simulink model "FeedBack_Linearization"  (R2021b)
(part 5 of 9)

t1997 = t961.*1.9738e-1;
t2000 = t869+t1374;
t2035 = t863+t1515;
t2039 = t1011.*1.9738e-1;
t2045 = t1013.*1.9738e-1;
t2053 = t919+t1532;
t2058 = (t1386+t7.*(t88-t617)).^2;
t2071 = t1060.*3.466000000000001e-2;
t2073 = t1064.*3.466000000000001e-2;
t2085 = t1061.*2.324e-2;
t2089 = t1063.*2.324e-2;
t2102 = t920+t1601;
t2116 = -dq7.*t8.*(t1386+t7.*(t88-t617));
t2119 = -dq7.*t15.*(t1386+t7.*(t88-t617));
t2140 = dq7.*t8.*(t1386+t7.*(t88-t617));
t2206 = t14.*t2179;
t2207 = t8.*t2182;
t2208 = t15.*t2182;
t2210 = -t2184;
t2213 = -t2186;
t2215 = -t2187;
t2216 = t6.*t2164;
t2218 = t7.*t2164;
t2220 = t7.*t2165;
t2221 = t8.*t2165;
t2222 = t13.*t2164;
t2223 = t14.*t2164;
t2224 = t14.*t2165;
t2225 = t15.*t2165;
t2229 = dq6.*t2180.*2.0;
t2231 = -t2202;
t2232 = dq5.*t2181.*2.0;
t2233 = dq6.*t2184.*2.0;
t2236 = dq5.*t2186.*2.0;
t2240 = t7.*t2179;
t2256 = t7.*t2212;
t2258 = t14.*t2212;
t2259 = t8.*t2217;
t2260 = -t2211;
t2261 = t15.*t2217;
t2265 = -t2219;
t2270 = dq7.*t1601.*(-2.324e-2);
t2273 = t1626.*(-2.324e-2);
t2278 = dq6.*t2214.*2.0;
t2280 = dq6.*t2219.*2.0;
t2288 = t1647.*(-3.466000000000001e-2);
t2289 = t916+t1792;
t2290 = t1626.*2.324e-2;
t2299 = t22.*t1601.*(-3.466000000000001e-2);
t2300 = t8.*t2262;
t2301 = t15.*t2262;
t2307 = dq7.*t2263.*2.0;
t2308 = dq7.*t2267.*2.0;
t2311 = t22.*t1601.*3.466000000000001e-2;
t2315 = t969+t1795;
t2352 = t1387+t1594;
t2357 = -t2351;
t2359 = t573.*t2165;
t2363 = t1375+t1633;
t2372 = t604.*t2164;
t2374 = t1528+t1631;
t2377 = -t2369;
t2378 = -t2370;
t2380 = t1516+t1668;
t2430 = -t2164.*(t88-t617);
C = ft_5({dq1,dq2,dq3,dq4,dq5,dq6,dq7,t10,t1000,t1001,t1003,t1004,t1007,t1008,t1010,t1012,t1013,t1014,t1015,t1016,t1017,t1018,t1019,t1020,t1021,t1022,t1023,t1024,t1025,t1026,t1029,t1031,t1032,t1033,t1034,t1035,t1036,t1038,t1039,t1040,t1041,t1044,t1045,t1046,t105,t1050,t1051,t1052,t1053,t1054,t1055,t1056,t1058,t1059,t1060,t1062,t1063,t1064,t1066,t1067,t1069,t107,t1070,t1072,t1074,t1075,t1076,t1077,t1079,t1081,t1089,t1091,t1092,t1094,t1096,t1097,t11,t1101,t1102,t1103,t1104,t1105,t1106,t1109,t1110,t1113,t1114,t1115,t1117,t1118,t1119,t112,t1123,t1125,t1126,t1128,t1130,t1132,t1135,t1136,t1137,t1138,t1139,t114,t1140,t1141,t1142,t1143,t1144,t1145,t1146,t1147,t1159,t1161,t1164,t1165,t1166,t1167,t1168,t1169,t1172,t1173,t1174,t1175,t1176,t1177,t1178,t1179,t1180,t1181,t1182,t1183,t1184,t1187,t1188,t1189,t119,t1190,t1193,t1194,t1195,t1197,t1198,t1199,t12,t1200,t1201,t1202,t1203,t1204,t1205,t1206,t1207,t1208,t1209,t1211,t1212,t1213,t1214,t1215,t1216,t1217,t1218,t1219,t122,t1220,t1224,t1225,t1226,t1228,t1229,t1231,t1232,t1238,t1242,t1243,t1244,t1246,t1249,t1250,t1253,t1256,t1257,t1263,t1264,t1265,t1267,t1268,t1269,t1270,t1273,t1274,t1275,t1286,t1287,t1288,t1289,t1290,t1291,t1292,t1293,t1295,t1296,t1299,t13,t130,t1300,t1304,t1305,t1306,t1309,t1312,t1313,t1315,t1318,t1325,t1327,t1328,t1329,t1330,t1339,t1341,t1342,t1346,t1347,t1348,t1349,t1350,t1351,t1352,t1356,t1357,t1360,t1361,t1362,t1363,t1364,t1365,t1368,t1369,t137,t1374,t1375,t1376,t1377,t1380,t1381,t1382,t1384,t1385,t1386,t1387,t1388,t1389,t139,t1390,t1391,t14,t1409,t1410,t1412,t1416,t1417,t1418,t1423,t1424,t1425,t1428,t1429,t1430,t1431,t1432,t1435,t1436,t144,t1441,t1449,t1450,t1451,t1453,t1455,t1456,t1462,t1467,t1471,t1472,t1473,t1474,t1475,t1480,t1487,t1488,t1489,t149,t1490,t1491,t1492,t1495,t1496,t1497,t1498,t15,t1506,t1508,t1509,t151,t1510,t1511,t1512,t1513,t1515,t1516,t1517,t1518,t1519,t152,t1526,t1527,t1528,t1529,t1530,t1537,t1538,t1539,t1540,t1541,t1542,t1543,t1544,t1545,t1546,t1547,t1548,t1549,t1550,t1551,t1552,t1553,t1554,t1556,t1557,t1561,t1562,t1563,t1564,t1565,t1566,t1567,t1568,t1569,t1570,t1571,t1572,t1574,t1577,t1578,t1579,t1581,t1582,t1583,t1584,t1585,t1589,t1591,t1596,t1598,t16,t160,t1601,t1603,t1604,t1605,t1606,t1607,t1608,t1609,t1611,t1612,t1613,t1616,t1618,t1622,t1624,t1625,t1626,t1627,t1629,t1630,t1633,t1634,t1635,t1636,t1637,t1638,t1642,t1643,t1644,t1647,t1648,t1649,t165,t1650,t1651,t1652,t1653,t1654,t1655,t1657,t1658,t1659,t1660,t1661,t1662,t1663,t1664,t1666,t1667,t1668,t1670,t1671,t1672,t1673,t1674,t1675,t1678,t1679,t1680,t1681,t1682,t1683,t1685,t1686,t1687,t1688,t1690,t1691,t1692,t1693,t1694,t1696,t1697,t1699,t17,t1700,t1701,t1702,t1704,t1705,t1706,t1707,t171,t1710,t1711,t1715,t1716,t1717,t1718,t1719,t1720,t1721,t1722,t1723,t1725,t1726,t1727,t1729,t1731,t1734,t1735,t1736,t1738,t1740,t1742,t1744,t1746,t1748,t1749,t175,t1751,t1752,t1757,t1759,t1760,t1761,t1762,t1763,t1765,t1766,t1769,t1770,t1772,t1773,t1774,t1775,t1776,t1779,t1780,t1782,t1786,t1790,t1791,t1792,t1793,t1795,t1798,t1799,t180,t1800,t1801,t1802,t1803,t1804,t1805,t1806,t1807,t1811,t1812,t1813,t1814,t1815,t1816,t1817,t1819,t182,t1822,t1823,t1824,t1825,t1826,t1827,t1828,t1829,t1830,t1831,t1834,t1835,t1836,t1837,t1839,t1840,t1841,t1842,t1843,t1844,t1846,t1847,t1849,t185,t1850,t1851,t1852,t1855,t1856,t1859,t186,t1860,t1861,t1863,t1864,t1865,t1866,t1867,t187,t1871,t1872,t1873,t1874,t1875,t1876,t1877,t1878,t1880,t1881,t1882,t1884,t1885,t1886,t1887,t1888,t189,t1890,t1891,t1892,t1893,t1896,t1897,t1898,t1900,t1901,t1902,t1903,t1905,t1907,t1908,t1909,t1911,t1912,t1913,t1914,t1915,t1917,t1918,t1919,t1921,t1922,t1924,t1927,t1928,t1932,t1933,t1934,t1935,t1936,t1937,t1941,t1942,t1944,t1945,t1946,t1949,t1950,t1951,t1952,t1953,t1955,t1957,t1959,t1960,t1962,t1963,t1967,t1968,t1969,t1970,t1971,t1974,t1975,t1976,t1977,t1978,t1980,t1982,t1983,t1984,t1985,t1986,t1988,t1990,t1992,t1997,t1998,t2,t2000,t2001,t2002,t2003,t2006,t2008,t2009,t2010,t2011,t2013,t2014,t2015,t2016,t2018,t2020,t2022,t2023,t2026,t2028,t2029,t2030,t2032,t2033,t2034,t2035,t2036,t2038,t2039,t2041,t2042,t2043,t2045,t2047,t2049,t2056,t2057,t2058,t2059,t2060,t2065,t2066,t2071,t2072,t2073,t2075,t2077,t2078,t208,t2082,t2083,t2085,t2086,t2089,t2093,t2094,t2098,t2099,t21,t2101,t2104,t2105,t2109,t2111,t2113,t2114,t2117,t2119,t2120,t2121,t2123,t2125,t2126,t2129,t2130,t2133,t2134,t2140,t2141,t2146,t2147,t2148,t2149,t2150,t2152,t2155,t2156,t2157,t2158,t2160,t2162,t2163,t2164,t2165,t2166,t2167,t2170,t2171,t2172,t2173,t2174,t2175,t2177,t2179,t2180,t2181,t2182,t2183,t2184,t2186,t2187,t2192,t2193,t2196,t2197,t22,t2201,t2204,t2206,t2207,t2208,t2209,t221,t2210,t2212,t2213,t2214,t2215,t2216,t2217,t2218,t2219,t2220,t2221,t2222,t2223,t2224,t2225,t2226,t2229,t223,t2230,t2231,t2232,t2233,t2236,t2240,t2249,t2251,t2256,t2258,t2259,t2260,t2261,t2262,t2263,t2265,t2266,t2267,t2270,t2272,t2277,t2278,t2280,t2284,t2285,t2288,t2289,t2290,t2292,t2293,t2296,t2298,t23,t230,t2300,t2301,t2306,t2307,t2308,t2309,t231,t2310,t2311,t2313,t2315,t2316,t2317,t2318,t232,t2327,t2331,t2333,t2336,t2337,t234,t2341,t2342,t2344,t2348,t235,t2350,t2351,t2352,t2353,t2356,t2357,t2359,t236,t2360,t2361,t2363,t2365,t2368,t2369,t237,t2370,t2372,t2374,t2376,t2377,t2378,t238,t2380,t2381,t2382,t2384,t2385,t2387,t2388,t239,t2390,t2391,t2393,t2396,t2397,t24,t240,t2400,t2402,t2403,t2404,t2405,t2406,t2407,t2408,t2409,t241,t2411,t2412,t2414,t2416,t2418,t242,t2422,t2423,t2424,t2425,t2426,t2427,t2428,t2429,t243,t2431,t2432,t2433,t2435,t2436,t2439,t244,t2440,t2441,t2442,t2443,t2444,t2447,t2449,t2451,t2453,t2455,t2456,t2458,t2459,t2462,t2463,t2464,t2466,t2467,t2468,t2469,t2470,t2471,t2472,t2473,t2474,t2475,t2479,t2480,t2481,t2484,t2490,t2492,t2493,t2494,t2496,t25,t250,t2502,t2506,t2508,t2509,t251,t2512,t2518,t252,t2525,t2526,t2527,t2528,t2529,t253,t2532,t2533,t2534,t2536,t2538,t2539,t254,t2547,t2548,t2549,t2550,t2551,t2558,t2572,t258,t2582,t2586,t259,t2594,t26,t2606,t2607,t2612,t2618,t2619,t2620,t2622,t2623,t2624,t2634,t2635,t2636,t2638,t2639,t2652,t2653,t2659,t2668,t267,t2671,t2672,t2673,t2674,t2675,t2677,t2678,t2679,t268,t2684,t2687,t269,t2690,t2691,t2693,t2696,t27,t270,t2701,t2703,t2706,t2707,t2708,t2709,t271,t2710,t2711,t2712,t2713,t2718,t272,t2720,t2722,t2725,t273,t2730,t2731,t2734,t2735,t274,t2745,t2748,t275,t2755,t2756,t2757,t2758,t276,t2760,t2761,t2762,t2765,t2766,t2768,t277,t2770,t2771,t2774,t2775,t2776,t2778,t2779,t2784,t2785,t2786,t2787,t2788,t279,t28,t280,t2802,t2805,t281,t282,t2822,t2827,t283,t2830,t2833,t2834,t284,t2844,t285,t2854,t286,t2869,t287,t2870,t288,t289,t2891,t2897,t2898,t2899,t29,t290,t2924,t2929,t293,t294,t2943,t2944,t2946,t295,t2952,t296,t2963,t297,t2971,t2972,t298,t3,t30,t301,t307,t308,t309,t31,t310,t311,t312,t313,t315,t316,t317,t318,t319,t32,t320,t322,t3248,t3249,t3252,t327,t328,t329,t33,t330,t331,t3372,t338,t34,t342,t3440,t3443,t346,t347,t3476,t348,t349,t35,t358,t36,t3669,t3672,t3673,t3679,t37,t387,t39,t390,t394,t4,t40,t406,t408,t415,t416,t417,t418,t419,t420,t427,t428,t429,t43,t431,t432,t433,t434,t435,t436,t438,t439,t441,t442,t443,t444,t446,t448,t45,t450,t451,t452,t453,t455,t456,t457,t458,t459,t46,t460,t461,t463,t464,t465,t466,t467,t468,t469,t470,t476,t477,t478,t479,t480,t481,t483,t484,t49,t494,t495,t496,t5,t50,t51,t510,t511,t512,t515,t516,t517,t518,t522,t523,t524,t525,t526,t527,t528,t529,t530,t531,t533,t534,t535,t536,t537,t538,t542,t543,t545,t546,t547,t548,t549,t55,t550,t551,t552,t553,t554,t556,t557,t558,t561,t562,t563,t564,t565,t566,t567,t568,t569,t57,t570,t571,t572,t573,t574,t575,t576,t577,t578,t579,t58,t580,t581,t582,t583,t584,t585,t586,t587,t588,t589,t590,t591,t592,t593,t594,t595,t596,t597,t598,t599,t6,t600,t601,t602,t603,t604,t605,t606,t607,t608,t609,t61,t612,t613,t614,t615,t616,t617,t618,t619,t620,t621,t622,t623,t624,t626,t627,t628,t629,t63,t631,t632,t633,t634,t635,t637,t639,t64,t640,t642,t643,t644,t646,t647,t648,t649,t650,t651,t652,t653,t654,t656,t657,t658,t660,t661,t662,t663,t664,t665,t667,t67,t670,t671,t673,t675,t676,t677,t678,t679,t680,t681,t683,t684,t685,t686,t687,t688,t689,t69,t691,t692,t693,t694,t695,t696,t697,t698,t699,t7,t70,t700,t701,t702,t703,t704,t705,t706,t707,t708,t71,t712,t713,t714,t72,t720,t721,t722,t723,t724,t725,t726,t728,t729,t73,t730,t731,t735,t74,t740,t743,t745,t748,t75,t750,t751,t753,t754,t755,t756,t757,t758,t759,t76,t760,t762,t764,t765,t766,t769,t77,t770,t773,t774,t776,t777,t778,t779,t78,t780,t782,t783,t785,t786,t787,t788,t79,t791,t792,t794,t795,t796,t797,t799,t8,t80,t800,t802,t803,t805,t806,t807,t809,t81,t810,t811,t812,t813,t814,t815,t816,t817,t818,t819,t82,t820,t821,t822,t827,t83,t831,t834,t835,t836,t837,t838,t839,t84,t840,t841,t842,t843,t845,t846,t847,t848,t849,t85,t850,t851,t853,t854,t855,t856,t857,t859,t86,t860,t862,t863,t864,t866,t867,t868,t87,t870,t871,t872,t873,t876,t877,t878,t88,t880,t881,t882,t883,t884,t885,t887,t888,t889,t89,t890,t891,t892,t893,t894,t895,t896,t897,t898,t899,t9,t90,t900,t901,t902,t903,t904,t905,t907,t908,t91,t911,t918,t92,t921,t922,t923,t926,t927,t928,t930,t931,t932,t933,t934,t935,t936,t937,t938,t939,t94,t940,t941,t942,t943,t945,t946,t947,t948,t949,t950,t951,t952,t953,t955,t957,t958,t959,t961,t963,t964,t966,t967,t969,t97,t972,t973,t974,t975,t976,t977,t978,t979,t980,t982,t983,t985,t986,t987,t988,t992,t994,t995,t997,t999});
end
function C = ft_5(ct)
dq1 = ct{1};
dq2 = ct{2};
dq3 = ct{3};
dq4 = ct{4};
dq5 = ct{5};
dq6 = ct{6};
dq7 = ct{7};
t10 = ct{8};
t1000 = ct{9};
t1001 = ct{10};
t1003 = ct{11};
t1004 = ct{12};
t1007 = ct{13};
t1008 = ct{14};
t1010 = ct{15};
t1012 = ct{16};
t1013 = ct{17};
t1014 = ct{18};
t1015 = ct{19};
t1016 = ct{20};
t1017 = ct{21};
t1018 = ct{22};
t1019 = ct{23};
t1020 = ct{24};
t1021 = ct{25};
t1022 = ct{26};
t1023 = ct{27};
t1024 = ct{28};
t1025 = ct{29};
t1026 = ct{30};
t1029 = ct{31};
t1031 = ct{32};
t1032 = ct{33};
t1033 = ct{34};
t1034 = ct{35};
t1035 = ct{36};
t1036 = ct{37};
t1038 = ct{38};
t1039 = ct{39};
t1040 = ct{40};
t1041 = ct{41};
t1044 = ct{42};
t1045 = ct{43};
t1046 = ct{44};
t105 = ct{45};
t1050 = ct{46};
t1051 = ct{47};
t1052 = ct{48};
t1053 = ct{49};
t1054 = ct{50};
t1055 = ct{51};
t1056 = ct{52};
t1058 = ct{53};
t1059 = ct{54};
t1060 = ct{55};
t1062 = ct{56};
t1063 = ct{57};
t1064 = ct{58};
t1066 = ct{59};
t1067 = ct{60};
t1069 = ct{61};
t107 = ct{62};
t1070 = ct{63};
t1072 = ct{64};
t1074 = ct{65};
t1075 = ct{66};
t1076 = ct{67};
t1077 = ct{68};
t1079 = ct{69};
t1081 = ct{70};
t1089 = ct{71};
t1091 = ct{72};
t1092 = ct{73};
t1094 = ct{74};
t1096 = ct{75};
t1097 = ct{76};
t11 = ct{77};
t1101 = ct{78};
t1102 = ct{79};
t1103 = ct{80};
t1104 = ct{81};
t1105 = ct{82};
t1106 = ct{83};
t1109 = ct{84};
t1110 = ct{85};
t1113 = ct{86};
t1114 = ct{87};
t1115 = ct{88};
t1117 = ct{89};
t1118 = ct{90};
t1119 = ct{91};
t112 = ct{92};
t1123 = ct{93};
t1125 = ct{94};
t1126 = ct{95};
t1128 = ct{96};
t1130 = ct{97};
t1132 = ct{98};
t1135 = ct{99};
t1136 = ct{100};
t1137 = ct{101};
t1138 = ct{102};
t1139 = ct{103};
t114 = ct{104};
t1140 = ct{105};
t1141 = ct{106};
t1142 = ct{107};
t1143 = ct{108};
t1144 = ct{109};
t1145 = ct{110};
t1146 = ct{111};
t1147 = ct{112};
t1159 = ct{113};
t1161 = ct{114};
t1164 = ct{115};
t1165 = ct{116};
t1166 = ct{117};
t1167 = ct{118};
t1168 = ct{119};
t1169 = ct{120};
t1172 = ct{121};
t1173 = ct{122};
t1174 = ct{123};
t1175 = ct{124};
t1176 = ct{125};
t1177 = ct{126};
t1178 = ct{127};
t1179 = ct{128};
t1180 = ct{129};
t1181 = ct{130};
t1182 = ct{131};
t1183 = ct{132};
t1184 = ct{133};
t1187 = ct{134};
t1188 = ct{135};
t1189 = ct{136};
t119 = ct{137};
t1190 = ct{138};
t1193 = ct{139};
t1194 = ct{140};
t1195 = ct{141};
t1197 = ct{142};
t1198 = ct{143};
t1199 = ct{144};
t12 = ct{145};
t1200 = ct{146};
t1201 = ct{147};
t1202 = ct{148};
t1203 = ct{149};
t1204 = ct{150};
t1205 = ct{151};
t1206 = ct{152};
t1207 = ct{153};
t1208 = ct{154};
t1209 = ct{155};
t1211 = ct{156};
t1212 = ct{157};
t1213 = ct{158};
t1214 = ct{159};
t1215 = ct{160};
t1216 = ct{161};
t1217 = ct{162};
t1218 = ct{163};
t1219 = ct{164};
t122 = ct{165};
t1220 = ct{166};
t1224 = ct{167};
t1225 = ct{168};
t1226 = ct{169};
t1228 = ct{170};
t1229 = ct{171};
t1231 = ct{172};
t1232 = ct{173};
t1238 = ct{174};
t1242 = ct{175};
t1243 = ct{176};
t1244 = ct{177};
t1246 = ct{178};
t1249 = ct{179};
t1250 = ct{180};
t1253 = ct{181};
t1256 = ct{182};
t1257 = ct{183};
t1263 = ct{184};
t1264 = ct{185};
t1265 = ct{186};
t1267 = ct{187};
t1268 = ct{188};
t1269 = ct{189};
t1270 = ct{190};
t1273 = ct{191};
t1274 = ct{192};
t1275 = ct{193};
t1286 = ct{194};
t1287 = ct{195};
t1288 = ct{196};
t1289 = ct{197};
t1290 = ct{198};
t1291 = ct{199};
t1292 = ct{200};
t1293 = ct{201};
t1295 = ct{202};
t1296 = ct{203};
t1299 = ct{204};
t13 = ct{205};
t130 = ct{206};
t1300 = ct{207};
t1304 = ct{208};
t1305 = ct{209};
t1306 = ct{210};
t1309 = ct{211};
t1312 = ct{212};
t1313 = ct{213};
t1315 = ct{214};
t1318 = ct{215};
t1325 = ct{216};
t1327 = ct{217};
t1328 = ct{218};
t1329 = ct{219};
t1330 = ct{220};
t1339 = ct{221};
t1341 = ct{222};
t1342 = ct{223};
t1346 = ct{224};
t1347 = ct{225};
t1348 = ct{226};
t1349 = ct{227};
t1350 = ct{228};
t1351 = ct{229};
t1352 = ct{230};
t1356 = ct{231};
t1357 = ct{232};
t1360 = ct{233};
t1361 = ct{234};
t1362 = ct{235};
t1363 = ct{236};
t1364 = ct{237};
t1365 = ct{238};
t1368 = ct{239};
t1369 = ct{240};
t137 = ct{241};
t1374 = ct{242};
t1375 = ct{243};
t1376 = ct{244};
t1377 = ct{245};
t1380 = ct{246};
t1381 = ct{247};
t1382 = ct{248};
t1384 = ct{249};
t1385 = ct{250};
t1386 = ct{251};
t1387 = ct{252};
t1388 = ct{253};
t1389 = ct{254};
t139 = ct{255};
t1390 = ct{256};
t1391 = ct{257};
t14 = ct{258};
t1409 = ct{259};
t1410 = ct{260};
t1412 = ct{261};
t1416 = ct{262};
t1417 = ct{263};
t1418 = ct{264};
t1423 = ct{265};
t1424 = ct{266};
t1425 = ct{267};
t1428 = ct{268};
t1429 = ct{269};
t1430 = ct{270};
t1431 = ct{271};
t1432 = ct{272};
t1435 = ct{273};
t1436 = ct{274};
t144 = ct{275};
t1441 = ct{276};
t1449 = ct{277};
t1450 = ct{278};
t1451 = ct{279};
t1453 = ct{280};
t1455 = ct{281};
t1456 = ct{282};
t1462 = ct{283};
t1467 = ct{284};
t1471 = ct{285};
t1472 = ct{286};
t1473 = ct{287};
t1474 = ct{288};
t1475 = ct{289};
t1480 = ct{290};
t1487 = ct{291};
t1488 = ct{292};
t1489 = ct{293};
t149 = ct{294};
t1490 = ct{295};
t1491 = ct{296};
t1492 = ct{297};
t1495 = ct{298};
t1496 = ct{299};
t1497 = ct{300};
t1498 = ct{301};
t15 = ct{302};
t1506 = ct{303};
t1508 = ct{304};
t1509 = ct{305};
t151 = ct{306};
t1510 = ct{307};
t1511 = ct{308};
t1512 = ct{309};
t1513 = ct{310};
t1515 = ct{311};
t1516 = ct{312};
t1517 = ct{313};
t1518 = ct{314};
t1519 = ct{315};
t152 = ct{316};
t1526 = ct{317};
t1527 = ct{318};
t1528 = ct{319};
t1529 = ct{320};
t1530 = ct{321};
t1537 = ct{322};
t1538 = ct{323};
t1539 = ct{324};
t1540 = ct{325};
t1541 = ct{326};
t1542 = ct{327};
t1543 = ct{328};
t1544 = ct{329};
t1545 = ct{330};
t1546 = ct{331};
t1547 = ct{332};
t1548 = ct{333};
t1549 = ct{334};
t1550 = ct{335};
t1551 = ct{336};
t1552 = ct{337};
t1553 = ct{338};
t1554 = ct{339};
t1556 = ct{340};
t1557 = ct{341};
t1561 = ct{342};
t1562 = ct{343};
t1563 = ct{344};
t1564 = ct{345};
t1565 = ct{346};
t1566 = ct{347};
t1567 = ct{348};
t1568 = ct{349};
t1569 = ct{350};
t1570 = ct{351};
t1571 = ct{352};
t1572 = ct{353};
t1574 = ct{354};
t1577 = ct{355};
t1578 = ct{356};
t1579 = ct{357};
t1581 = ct{358};
t1582 = ct{359};
t1583 = ct{360};
t1584 = ct{361};
t1585 = ct{362};
t1589 = ct{363};
t1591 = ct{364};
t1596 = ct{365};
t1598 = ct{366};
t16 = ct{367};
t160 = ct{368};
t1601 = ct{369};
t1603 = ct{370};
t1604 = ct{371};
t1605 = ct{372};
t1606 = ct{373};
t1607 = ct{374};
t1608 = ct{375};
t1609 = ct{376};
t1611 = ct{377};
t1612 = ct{378};
t1613 = ct{379};
t1616 = ct{380};
t1618 = ct{381};
t1622 = ct{382};
t1624 = ct{383};
t1625 = ct{384};
t1626 = ct{385};
t1627 = ct{386};
t1629 = ct{387};
t1630 = ct{388};
t1633 = ct{389};
t1634 = ct{390};
t1635 = ct{391};
t1636 = ct{392};
t1637 = ct{393};
t1638 = ct{394};
t1642 = ct{395};
t1643 = ct{396};
t1644 = ct{397};
t1647 = ct{398};
t1648 = ct{399};
t1649 = ct{400};
t165 = ct{401};
t1650 = ct{402};
t1651 = ct{403};
t1652 = ct{404};
t1653 = ct{405};
t1654 = ct{406};
t1655 = ct{407};
t1657 = ct{408};
t1658 = ct{409};
t1659 = ct{410};
t1660 = ct{411};
t1661 = ct{412};
t1662 = ct{413};
t1663 = ct{414};
t1664 = ct{415};
t1666 = ct{416};
t1667 = ct{417};
t1668 = ct{418};
t1670 = ct{419};
t1671 = ct{420};
t1672 = ct{421};
t1673 = ct{422};
t1674 = ct{423};
t1675 = ct{424};
t1678 = ct{425};
t1679 = ct{426};
t1680 = ct{427};
t1681 = ct{428};
t1682 = ct{429};
t1683 = ct{430};
t1685 = ct{431};
t1686 = ct{432};
t1687 = ct{433};
t1688 = ct{434};
t1690 = ct{435};
t1691 = ct{436};
t1692 = ct{437};
t1693 = ct{438};
t1694 = ct{439};
t1696 = ct{440};
t1697 = ct{441};
t1699 = ct{442};
t17 = ct{443};
t1700 = ct{444};
t1701 = ct{445};
t1702 = ct{446};
t1704 = ct{447};
t1705 = ct{448};
t1706 = ct{449};
t1707 = ct{450};
t171 = ct{451};
t1710 = ct{452};
t1711 = ct{453};
t1715 = ct{454};
t1716 = ct{455};
t1717 = ct{456};
t1718 = ct{457};
t1719 = ct{458};
t1720 = ct{459};
t1721 = ct{460};
t1722 = ct{461};
t1723 = ct{462};
t1725 = ct{463};
t1726 = ct{464};
t1727 = ct{465};
t1729 = ct{466};
t1731 = ct{467};
t1734 = ct{468};
t1735 = ct{469};
t1736 = ct{470};
t1738 = ct{471};
t1740 = ct{472};
t1742 = ct{473};
t1744 = ct{474};
t1746 = ct{475};
t1748 = ct{476};
t1749 = ct{477};
t175 = ct{478};
t1751 = ct{479};
t1752 = ct{480};
t1757 = ct{481};
t1759 = ct{482};
t1760 = ct{483};
t1761 = ct{484};
t1762 = ct{485};
t1763 = ct{486};
t1765 = ct{487};
t1766 = ct{488};
t1769 = ct{489};
t1770 = ct{490};
t1772 = ct{491};
t1773 = ct{492};
t1774 = ct{493};
t1775 = ct{494};
t1776 = ct{495};
t1779 = ct{496};
t1780 = ct{497};
t1782 = ct{498};
t1786 = ct{499};
t1790 = ct{500};
t1791 = ct{501};
t1792 = ct{502};
t1793 = ct{503};
t1795 = ct{504};
t1798 = ct{505};
t1799 = ct{506};
t180 = ct{507};
t1800 = ct{508};
t1801 = ct{509};
t1802 = ct{510};
t1803 = ct{511};
t1804 = ct{512};
t1805 = ct{513};
t1806 = ct{514};
t1807 = ct{515};
t1811 = ct{516};
t1812 = ct{517};
t1813 = ct{518};
t1814 = ct{519};
t1815 = ct{520};
t1816 = ct{521};
t1817 = ct{522};
t1819 = ct{523};
t182 = ct{524};
t1822 = ct{525};
t1823 = ct{526};
t1824 = ct{527};
t1825 = ct{528};
t1826 = ct{529};
t1827 = ct{530};
t1828 = ct{531};
t1829 = ct{532};
t1830 = ct{533};
t1831 = ct{534};
t1834 = ct{535};
t1835 = ct{536};
t1836 = ct{537};
t1837 = ct{538};
t1839 = ct{539};
t1840 = ct{540};
t1841 = ct{541};
t1842 = ct{542};
t1843 = ct{543};
t1844 = ct{544};
t1846 = ct{545};
t1847 = ct{546};
t1849 = ct{547};
t185 = ct{548};
t1850 = ct{549};
t1851 = ct{550};
t1852 = ct{551};
t1855 = ct{552};
t1856 = ct{553};
t1859 = ct{554};
t186 = ct{555};
t1860 = ct{556};
t1861 = ct{557};
t1863 = ct{558};
t1864 = ct{559};
t1865 = ct{560};
t1866 = ct{561};
t1867 = ct{562};
t187 = ct{563};
t1871 = ct{564};
t1872 = ct{565};
t1873 = ct{566};
t1874 = ct{567};
t1875 = ct{568};
t1876 = ct{569};
t1877 = ct{570};
t1878 = ct{571};
t1880 = ct{572};
t1881 = ct{573};
t1882 = ct{574};
t1884 = ct{575};
t1885 = ct{576};
t1886 = ct{577};
t1887 = ct{578};
t1888 = ct{579};
t189 = ct{580};
t1890 = ct{581};
t1891 = ct{582};
t1892 = ct{583};
t1893 = ct{584};
t1896 = ct{585};
t1897 = ct{586};
t1898 = ct{587};
t1900 = ct{588};
t1901 = ct{589};
t1902 = ct{590};
t1903 = ct{591};
t1905 = ct{592};
t1907 = ct{593};
t1908 = ct{594};
t1909 = ct{595};
t1911 = ct{596};
t1912 = ct{597};
t1913 = ct{598};
t1914 = ct{599};
t1915 = ct{600};
t1917 = ct{601};
t1918 = ct{602};
t1919 = ct{603};
t1921 = ct{604};
t1922 = ct{605};
t1924 = ct{606};
t1927 = ct{607};
t1928 = ct{608};
t1932 = ct{609};
t1933 = ct{610};
t1934 = ct{611};
t1935 = ct{612};
t1936 = ct{613};
t1937 = ct{614};
t1941 = ct{615};
t1942 = ct{616};
t1944 = ct{617};
t1945 = ct{618};
t1946 = ct{619};
t1949 = ct{620};
t1950 = ct{621};
t1951 = ct{622};
t1952 = ct{623};
t1953 = ct{624};
t1955 = ct{625};
t1957 = ct{626};
t1959 = ct{627};
t1960 = ct{628};
t1962 = ct{629};
t1963 = ct{630};
t1967 = ct{631};
t1968 = ct{632};
t1969 = ct{633};
t1970 = ct{634};
t1971 = ct{635};
t1974 = ct{636};
t1975 = ct{637};
t1976 = ct{638};
t1977 = ct{639};
t1978 = ct{640};
t1980 = ct{641};
t1982 = ct{642};
t1983 = ct{643};
t1984 = ct{644};
t1985 = ct{645};
t1986 = ct{646};
t1988 = ct{647};
t1990 = ct{648};
t1992 = ct{649};
t1997 = ct{650};
t1998 = ct{651};
t2 = ct{652};
t2000 = ct{653};
t2001 = ct{654};
t2002 = ct{655};
t2003 = ct{656};
t2006 = ct{657};
t2008 = ct{658};
t2009 = ct{659};
t2010 = ct{660};
t2011 = ct{661};
t2013 = ct{662};
t2014 = ct{663};
t2015 = ct{664};
t2016 = ct{665};
t2018 = ct{666};
t2020 = ct{667};
t2022 = ct{668};
t2023 = ct{669};
t2026 = ct{670};
t2028 = ct{671};
t2029 = ct{672};
t2030 = ct{673};
t2032 = ct{674};
t2033 = ct{675};
t2034 = ct{676};
t2035 = ct{677};
t2036 = ct{678};
t2038 = ct{679};
t2039 = ct{680};
t2041 = ct{681};
t2042 = ct{682};
t2043 = ct{683};
t2045 = ct{684};
t2047 = ct{685};
t2049 = ct{686};
t2056 = ct{687};
t2057 = ct{688};
t2058 = ct{689};
t2059 = ct{690};
t2060 = ct{691};
t2065 = ct{692};
t2066 = ct{693};
t2071 = ct{694};
t2072 = ct{695};
t2073 = ct{696};
t2075 = ct{697};
t2077 = ct{698};
t2078 = ct{699};
t208 = ct{700};
t2082 = ct{701};
t2083 = ct{702};
t2085 = ct{703};
t2086 = ct{704};
t2089 = ct{705};
t2093 = ct{706};
t2094 = ct{707};
t2098 = ct{708};
t2099 = ct{709};
t21 = ct{710};
t2101 = ct{711};
t2104 = ct{712};
t2105 = ct{713};
t2109 = ct{714};
t2111 = ct{715};
t2113 = ct{716};
t2114 = ct{717};
t2117 = ct{718};
t2119 = ct{719};
t2120 = ct{720};
t2121 = ct{721};
t2123 = ct{722};
t2125 = ct{723};
t2126 = ct{724};
t2129 = ct{725};
t2130 = ct{726};
t2133 = ct{727};
t2134 = ct{728};
t2140 = ct{729};
t2141 = ct{730};
t2146 = ct{731};
t2147 = ct{732};
t2148 = ct{733};
t2149 = ct{734};
t2150 = ct{735};
t2152 = ct{736};
t2155 = ct{737};
t2156 = ct{738};
t2157 = ct{739};
t2158 = ct{740};
t2160 = ct{741};
t2162 = ct{742};
t2163 = ct{743};
t2164 = ct{744};
t2165 = ct{745};
t2166 = ct{746};
t2167 = ct{747};
t2170 = ct{748};
t2171 = ct{749};
t2172 = ct{750};
t2173 = ct{751};
t2174 = ct{752};
t2175 = ct{753};
t2177 = ct{754};
t2179 = ct{755};
t2180 = ct{756};
t2181 = ct{757};
t2182 = ct{758};
t2183 = ct{759};
t2184 = ct{760};
t2186 = ct{761};
t2187 = ct{762};
t2192 = ct{763};
t2193 = ct{764};
t2196 = ct{765};
t2197 = ct{766};
t22 = ct{767};
t2201 = ct{768};
t2204 = ct{769};
t2206 = ct{770};
t2207 = ct{771};
t2208 = ct{772};
t2209 = ct{773};
t221 = ct{774};
t2210 = ct{775};
t2212 = ct{776};
t2213 = ct{777};
t2214 = ct{778};
t2215 = ct{779};
t2216 = ct{780};
t2217 = ct{781};
t2218 = ct{782};
t2219 = ct{783};
t2220 = ct{784};
t2221 = ct{785};
t2222 = ct{786};
t2223 = ct{787};
t2224 = ct{788};
t2225 = ct{789};
t2226 = ct{790};
t2229 = ct{791};
t223 = ct{792};
t2230 = ct{793};
t2231 = ct{794};
t2232 = ct{795};
t2233 = ct{796};
t2236 = ct{797};
t2240 = ct{798};
t2249 = ct{799};
t2251 = ct{800};
t2256 = ct{801};
t2258 = ct{802};
t2259 = ct{803};
t2260 = ct{804};
t2261 = ct{805};
t2262 = ct{806};
t2263 = ct{807};
t2265 = ct{808};
t2266 = ct{809};
t2267 = ct{810};
t2270 = ct{811};
t2272 = ct{812};
t2277 = ct{813};
t2278 = ct{814};
t2280 = ct{815};
t2284 = ct{816};
t2285 = ct{817};
t2288 = ct{818};
t2289 = ct{819};
t2290 = ct{820};
t2292 = ct{821};
t2293 = ct{822};
t2296 = ct{823};
t2298 = ct{824};
t23 = ct{825};
t230 = ct{826};
t2300 = ct{827};
t2301 = ct{828};
t2306 = ct{829};
t2307 = ct{830};
t2308 = ct{831};
t2309 = ct{832};
t231 = ct{833};
t2310 = ct{834};
t2311 = ct{835};
t2313 = ct{836};
t2315 = ct{837};
t2316 = ct{838};
t2317 = ct{839};
t2318 = ct{840};
t232 = ct{841};
t2327 = ct{842};
t2331 = ct{843};
t2333 = ct{844};
t2336 = ct{845};
t2337 = ct{846};
t234 = ct{847};
t2341 = ct{848};
t2342 = ct{849};
t2344 = ct{850};
t2348 = ct{851};
t235 = ct{852};
t2350 = ct{853};
t2351 = ct{854};
t2352 = ct{855};
t2353 = ct{856};
t2356 = ct{857};
t2357 = ct{858};
t2359 = ct{859};
t236 = ct{860};
t2360 = ct{861};
t2361 = ct{862};
t2363 = ct{863};
t2365 = ct{864};
t2368 = ct{865};
t2369 = ct{866};
t237 = ct{867};
t2370 = ct{868};
t2372 = ct{869};
t2374 = ct{870};
t2376 = ct{871};
t2377 = ct{872};
t2378 = ct{873};
t238 = ct{874};
t2380 = ct{875};
t2381 = ct{876};
t2382 = ct{877};
t2384 = ct{878};
t2385 = ct{879};
t2387 = ct{880};
t2388 = ct{881};
t239 = ct{882};
t2390 = ct{883};
t2391 = ct{884};
t2393 = ct{885};
t2396 = ct{886};
t2397 = ct{887};
t24 = ct{888};
t240 = ct{889};
t2400 = ct{890};
t2402 = ct{891};
t2403 = ct{892};
t2404 = ct{893};
t2405 = ct{894};
t2406 = ct{895};
t2407 = ct{896};
t2408 = ct{897};
t2409 = ct{898};
t241 = ct{899};
t2411 = ct{900};
t2412 = ct{901};
t2414 = ct{902};
t2416 = ct{903};
t2418 = ct{904};
t242 = ct{905};
t2422 = ct{906};
t2423 = ct{907};
t2424 = ct{908};
t2425 = ct{909};
t2426 = ct{910};
t2427 = ct{911};
t2428 = ct{912};
t2429 = ct{913};
t243 = ct{914};
t2431 = ct{915};
t2432 = ct{916};
t2433 = ct{917};
t2435 = ct{918};
t2436 = ct{919};
t2439 = ct{920};
t244 = ct{921};
t2440 = ct{922};
t2441 = ct{923};
t2442 = ct{924};
t2443 = ct{925};
t2444 = ct{926};
t2447 = ct{927};
t2449 = ct{928};
t2451 = ct{929};
t2453 = ct{930};
t2455 = ct{931};
t2456 = ct{932};
t2458 = ct{933};
t2459 = ct{934};
t2462 = ct{935};
t2463 = ct{936};
t2464 = ct{937};
t2466 = ct{938};
t2467 = ct{939};
t2468 = ct{940};
t2469 = ct{941};
t2470 = ct{942};
t2471 = ct{943};
t2472 = ct{944};
t2473 = ct{945};
t2474 = ct{946};
t2475 = ct{947};
t2479 = ct{948};
t2480 = ct{949};
t2481 = ct{950};
t2484 = ct{951};
t2490 = ct{952};
t2492 = ct{953};
t2493 = ct{954};
t2494 = ct{955};
t2496 = ct{956};
t25 = ct{957};
t250 = ct{958};
t2502 = ct{959};
t2506 = ct{960};
t2508 = ct{961};
t2509 = ct{962};
t251 = ct{963};
t2512 = ct{964};
t2518 = ct{965};
t252 = ct{966};
t2525 = ct{967};
t2526 = ct{968};
t2527 = ct{969};
t2528 = ct{970};
t2529 = ct{971};
t253 = ct{972};
t2532 = ct{973};
t2533 = ct{974};
t2534 = ct{975};
t2536 = ct{976};
t2538 = ct{977};
t2539 = ct{978};
t254 = ct{979};
t2547 = ct{980};
t2548 = ct{981};
t2549 = ct{982};
t2550 = ct{983};
t2551 = ct{984};
t2558 = ct{985};
t2572 = ct{986};
t258 = ct{987};
t2582 = ct{988};
t2586 = ct{989};
t259 = ct{990};
t2594 = ct{991};
t26 = ct{992};
t2606 = ct{993};
t2607 = ct{994};
t2612 = ct{995};
t2618 = ct{996};
t2619 = ct{997};
t2620 = ct{998};
t2622 = ct{999};
t2623 = ct{1000};
t2624 = ct{1001};
t2634 = ct{1002};
t2635 = ct{1003};
t2636 = ct{1004};
t2638 = ct{1005};
t2639 = ct{1006};
t2652 = ct{1007};
t2653 = ct{1008};
t2659 = ct{1009};
t2668 = ct{1010};
t267 = ct{1011};
t2671 = ct{1012};
t2672 = ct{1013};
t2673 = ct{1014};
t2674 = ct{1015};
t2675 = ct{1016};
t2677 = ct{1017};
t2678 = ct{1018};
t2679 = ct{1019};
t268 = ct{1020};
t2684 = ct{1021};
t2687 = ct{1022};
t269 = ct{1023};
t2690 = ct{1024};
t2691 = ct{1025};
t2693 = ct{1026};
t2696 = ct{1027};
t27 = ct{1028};
t270 = ct{1029};
t2701 = ct{1030};
t2703 = ct{1031};
t2706 = ct{1032};
t2707 = ct{1033};
t2708 = ct{1034};
t2709 = ct{1035};
t271 = ct{1036};
t2710 = ct{1037};
t2711 = ct{1038};
t2712 = ct{1039};
t2713 = ct{1040};
t2718 = ct{1041};
t272 = ct{1042};
t2720 = ct{1043};
t2722 = ct{1044};
t2725 = ct{1045};
t273 = ct{1046};
t2730 = ct{1047};
t2731 = ct{1048};
t2734 = ct{1049};
t2735 = ct{1050};
t274 = ct{1051};
t2745 = ct{1052};
t2748 = ct{1053};
t275 = ct{1054};
t2755 = ct{1055};
t2756 = ct{1056};
t2757 = ct{1057};
t2758 = ct{1058};
t276 = ct{1059};
t2760 = ct{1060};
t2761 = ct{1061};
t2762 = ct{1062};
t2765 = ct{1063};
t2766 = ct{1064};
t2768 = ct{1065};
t277 = ct{1066};
t2770 = ct{1067};
t2771 = ct{1068};
t2774 = ct{1069};
t2775 = ct{1070};
t2776 = ct{1071};
t2778 = ct{1072};
t2779 = ct{1073};
t2784 = ct{1074};
t2785 = ct{1075};
t2786 = ct{1076};
t2787 = ct{1077};
t2788 = ct{1078};
t279 = ct{1079};
t28 = ct{1080};
t280 = ct{1081};
t2802 = ct{1082};
t2805 = ct{1083};
t281 = ct{1084};
t282 = ct{1085};
t2822 = ct{1086};
t2827 = ct{1087};
t283 = ct{1088};
t2830 = ct{1089};
t2833 = ct{1090};
t2834 = ct{1091};
t284 = ct{1092};
t2844 = ct{1093};
t285 = ct{1094};
t2854 = ct{1095};
t286 = ct{1096};
t2869 = ct{1097};
t287 = ct{1098};
t2870 = ct{1099};
t288 = ct{1100};
t289 = ct{1101};
t2891 = ct{1102};
t2897 = ct{1103};
t2898 = ct{1104};
t2899 = ct{1105};
t29 = ct{1106};
t290 = ct{1107};
t2924 = ct{1108};
t2929 = ct{1109};
t293 = ct{1110};
t294 = ct{1111};
t2943 = ct{1112};
t2944 = ct{1113};
t2946 = ct{1114};
t295 = ct{1115};
t2952 = ct{1116};
t296 = ct{1117};
t2963 = ct{1118};
t297 = ct{1119};
t2971 = ct{1120};
t2972 = ct{1121};
t298 = ct{1122};
t3 = ct{1123};
t30 = ct{1124};
t301 = ct{1125};
t307 = ct{1126};
t308 = ct{1127};
t309 = ct{1128};
t31 = ct{1129};
t310 = ct{1130};
t311 = ct{1131};
t312 = ct{1132};
t313 = ct{1133};
t315 = ct{1134};
t316 = ct{1135};
t317 = ct{1136};
t318 = ct{1137};
t319 = ct{1138};
t32 = ct{1139};
t320 = ct{1140};
t322 = ct{1141};
t3248 = ct{1142};
t3249 = ct{1143};
t3252 = ct{1144};
t327 = ct{1145};
t328 = ct{1146};
t329 = ct{1147};
t33 = ct{1148};
t330 = ct{1149};
t331 = ct{1150};
t3372 = ct{1151};
t338 = ct{1152};
t34 = ct{1153};
t342 = ct{1154};
t3440 = ct{1155};
t3443 = ct{1156};
t346 = ct{1157};
t347 = ct{1158};
t3476 = ct{1159};
t348 = ct{1160};
t349 = ct{1161};
t35 = ct{1162};
t358 = ct{1163};
t36 = ct{1164};
t3669 = ct{1165};
t3672 = ct{1166};
t3673 = ct{1167};
t3679 = ct{1168};
t37 = ct{1169};
t387 = ct{1170};
t39 = ct{1171};
t390 = ct{1172};
t394 = ct{1173};
t4 = ct{1174};
t40 = ct{1175};
t406 = ct{1176};
t408 = ct{1177};
t415 = ct{1178};
t416 = ct{1179};
t417 = ct{1180};
t418 = ct{1181};
t419 = ct{1182};
t420 = ct{1183};
t427 = ct{1184};
t428 = ct{1185};
t429 = ct{1186};
t43 = ct{1187};
t431 = ct{1188};
t432 = ct{1189};
t433 = ct{1190};
t434 = ct{1191};
t435 = ct{1192};
t436 = ct{1193};
t438 = ct{1194};
t439 = ct{1195};
t441 = ct{1196};
t442 = ct{1197};
t443 = ct{1198};
t444 = ct{1199};
t446 = ct{1200};
t448 = ct{1201};
t45 = ct{1202};
t450 = ct{1203};
t451 = ct{1204};
t452 = ct{1205};
t453 = ct{1206};
t455 = ct{1207};
t456 = ct{1208};
t457 = ct{1209};
t458 = ct{1210};
t459 = ct{1211};
t46 = ct{1212};
t460 = ct{1213};
t461 = ct{1214};
t463 = ct{1215};
t464 = ct{1216};
t465 = ct{1217};
t466 = ct{1218};
t467 = ct{1219};
t468 = ct{1220};
t469 = ct{1221};
t470 = ct{1222};
t476 = ct{1223};
t477 = ct{1224};
t478 = ct{1225};
t479 = ct{1226};
t480 = ct{1227};
t481 = ct{1228};
t483 = ct{1229};
t484 = ct{1230};
t49 = ct{1231};
t494 = ct{1232};
t495 = ct{1233};
t496 = ct{1234};
t5 = ct{1235};
t50 = ct{1236};
t51 = ct{1237};
t510 = ct{1238};
t511 = ct{1239};
t512 = ct{1240};
t515 = ct{1241};
t516 = ct{1242};
t517 = ct{1243};
t518 = ct{1244};
t522 = ct{1245};
t523 = ct{1246};
t524 = ct{1247};
t525 = ct{1248};
t526 = ct{1249};
t527 = ct{1250};
t528 = ct{1251};
t529 = ct{1252};
t530 = ct{1253};
t531 = ct{1254};
t533 = ct{1255};
t534 = ct{1256};
t535 = ct{1257};
t536 = ct{1258};
t537 = ct{1259};
t538 = ct{1260};
t542 = ct{1261};
t543 = ct{1262};
t545 = ct{1263};
t546 = ct{1264};
t547 = ct{1265};
t548 = ct{1266};
t549 = ct{1267};
t55 = ct{1268};
t550 = ct{1269};
t551 = ct{1270};
t552 = ct{1271};
t553 = ct{1272};
t554 = ct{1273};
t556 = ct{1274};
t557 = ct{1275};
t558 = ct{1276};
t561 = ct{1277};
t562 = ct{1278};
t563 = ct{1279};
t564 = ct{1280};
t565 = ct{1281};
t566 = ct{1282};
t567 = ct{1283};
t568 = ct{1284};
t569 = ct{1285};
t57 = ct{1286};
t570 = ct{1287};
t571 = ct{1288};
t572 = ct{1289};
t573 = ct{1290};
t574 = ct{1291};
t575 = ct{1292};
t576 = ct{1293};
t577 = ct{1294};
t578 = ct{1295};
t579 = ct{1296};
t58 = ct{1297};
t580 = ct{1298};
t581 = ct{1299};
t582 = ct{1300};
t583 = ct{1301};
t584 = ct{1302};
t585 = ct{1303};
t586 = ct{1304};
t587 = ct{1305};
t588 = ct{1306};
t589 = ct{1307};
t590 = ct{1308};
t591 = ct{1309};
t592 = ct{1310};
t593 = ct{1311};
t594 = ct{1312};
t595 = ct{1313};
t596 = ct{1314};
t597 = ct{1315};
t598 = ct{1316};
t599 = ct{1317};
t6 = ct{1318};
t600 = ct{1319};
t601 = ct{1320};
t602 = ct{1321};
t603 = ct{1322};
t604 = ct{1323};
t605 = ct{1324};
t606 = ct{1325};
t607 = ct{1326};
t608 = ct{1327};
t609 = ct{1328};
t61 = ct{1329};
t612 = ct{1330};
t613 = ct{1331};
t614 = ct{1332};
t615 = ct{1333};
t616 = ct{1334};
t617 = ct{1335};
t618 = ct{1336};
t619 = ct{1337};
t620 = ct{1338};
t621 = ct{1339};
t622 = ct{1340};
t623 = ct{1341};
t624 = ct{1342};
t626 = ct{1343};
t627 = ct{1344};
t628 = ct{1345};
t629 = ct{1346};
t63 = ct{1347};
t631 = ct{1348};
t632 = ct{1349};
t633 = ct{1350};
t634 = ct{1351};
t635 = ct{1352};
t637 = ct{1353};
t639 = ct{1354};
t64 = ct{1355};
t640 = ct{1356};
t642 = ct{1357};
t643 = ct{1358};
t644 = ct{1359};
t646 = ct{1360};
t647 = ct{1361};
t648 = ct{1362};
t649 = ct{1363};
t650 = ct{1364};
t651 = ct{1365};
t652 = ct{1366};
t653 = ct{1367};
t654 = ct{1368};
t656 = ct{1369};
t657 = ct{1370};
t658 = ct{1371};
t660 = ct{1372};
t661 = ct{1373};
t662 = ct{1374};
t663 = ct{1375};
t664 = ct{1376};
t665 = ct{1377};
t667 = ct{1378};
t67 = ct{1379};
t670 = ct{1380};
t671 = ct{1381};
t673 = ct{1382};
t675 = ct{1383};
t676 = ct{1384};
t677 = ct{1385};
t678 = ct{1386};
t679 = ct{1387};
t680 = ct{1388};
t681 = ct{1389};
t683 = ct{1390};
t684 = ct{1391};
t685 = ct{1392};
t686 = ct{1393};
t687 = ct{1394};
t688 = ct{1395};
t689 = ct{1396};
t69 = ct{1397};
t691 = ct{1398};
t692 = ct{1399};
t693 = ct{1400};
t694 = ct{1401};
t695 = ct{1402};
t696 = ct{1403};
t697 = ct{1404};
t698 = ct{1405};
t699 = ct{1406};
t7 = ct{1407};
t70 = ct{1408};
t700 = ct{1409};
t701 = ct{1410};
t702 = ct{1411};
t703 = ct{1412};
t704 = ct{1413};
t705 = ct{1414};
t706 = ct{1415};
t707 = ct{1416};
t708 = ct{1417};
t71 = ct{1418};
t712 = ct{1419};
t713 = ct{1420};
t714 = ct{1421};
t72 = ct{1422};
t720 = ct{1423};
t721 = ct{1424};
t722 = ct{1425};
t723 = ct{1426};
t724 = ct{1427};
t725 = ct{1428};
t726 = ct{1429};
t728 = ct{1430};
t729 = ct{1431};
t73 = ct{1432};
t730 = ct{1433};
t731 = ct{1434};
t735 = ct{1435};
t74 = ct{1436};
t740 = ct{1437};
t743 = ct{1438};
t745 = ct{1439};
t748 = ct{1440};
t75 = ct{1441};
t750 = ct{1442};
t751 = ct{1443};
t753 = ct{1444};
t754 = ct{1445};
t755 = ct{1446};
t756 = ct{1447};
t757 = ct{1448};
t758 = ct{1449};
t759 = ct{1450};
t76 = ct{1451};
t760 = ct{1452};
t762 = ct{1453};
t764 = ct{1454};
t765 = ct{1455};
t766 = ct{1456};
t769 = ct{1457};
t77 = ct{1458};
t770 = ct{1459};
t773 = ct{1460};
t774 = ct{1461};
t776 = ct{1462};
t777 = ct{1463};
t778 = ct{1464};
t779 = ct{1465};
t78 = ct{1466};
t780 = ct{1467};
t782 = ct{1468};
t783 = ct{1469};
t785 = ct{1470};
t786 = ct{1471};
t787 = ct{1472};
t788 = ct{1473};
t79 = ct{1474};
t791 = ct{1475};
t792 = ct{1476};
t794 = ct{1477};
t795 = ct{1478};
t796 = ct{1479};
t797 = ct{1480};
t799 = ct{1481};
t8 = ct{1482};
t80 = ct{1483};
t800 = ct{1484};
t802 = ct{1485};
t803 = ct{1486};
t805 = ct{1487};
t806 = ct{1488};
t807 = ct{1489};
t809 = ct{1490};
t81 = ct{1491};
t810 = ct{1492};
t811 = ct{1493};
t812 = ct{1494};
t813 = ct{1495};
t814 = ct{1496};
t815 = ct{1497};
t816 = ct{1498};
t817 = ct{1499};
t818 = ct{1500};
t819 = ct{1501};
t82 = ct{1502};
t820 = ct{1503};
t821 = ct{1504};
t822 = ct{1505};
t827 = ct{1506};
t83 = ct{1507};
t831 = ct{1508};
t834 = ct{1509};
t835 = ct{1510};
t836 = ct{1511};
t837 = ct{1512};
t838 = ct{1513};
t839 = ct{1514};
t84 = ct{1515};
t840 = ct{1516};
t841 = ct{1517};
t842 = ct{1518};
t843 = ct{1519};
t845 = ct{1520};
t846 = ct{1521};
t847 = ct{1522};
t848 = ct{1523};
t849 = ct{1524};
t85 = ct{1525};
t850 = ct{1526};
t851 = ct{1527};
t853 = ct{1528};
t854 = ct{1529};
t855 = ct{1530};
t856 = ct{1531};
t857 = ct{1532};
t859 = ct{1533};
t86 = ct{1534};
t860 = ct{1535};
t862 = ct{1536};
t863 = ct{1537};
t864 = ct{1538};
t866 = ct{1539};
t867 = ct{1540};
t868 = ct{1541};
t87 = ct{1542};
t870 = ct{1543};
t871 = ct{1544};
t872 = ct{1545};
t873 = ct{1546};
t876 = ct{1547};
t877 = ct{1548};
t878 = ct{1549};
t88 = ct{1550};
t880 = ct{1551};
t881 = ct{1552};
t882 = ct{1553};
t883 = ct{1554};
t884 = ct{1555};
t885 = ct{1556};
t887 = ct{1557};
t888 = ct{1558};
t889 = ct{1559};
t89 = ct{1560};
t890 = ct{1561};
t891 = ct{1562};
t892 = ct{1563};
t893 = ct{1564};
t894 = ct{1565};
t895 = ct{1566};
t896 = ct{1567};
t897 = ct{1568};
t898 = ct{1569};
t899 = ct{1570};
t9 = ct{1571};
t90 = ct{1572};
t900 = ct{1573};
t901 = ct{1574};
t902 = ct{1575};
t903 = ct{1576};
t904 = ct{1577};
t905 = ct{1578};
t907 = ct{1579};
t908 = ct{1580};
t91 = ct{1581};
t911 = ct{1582};
t918 = ct{1583};
t92 = ct{1584};
t921 = ct{1585};
t922 = ct{1586};
t923 = ct{1587};
t926 = ct{1588};
t927 = ct{1589};
t928 = ct{1590};
t930 = ct{1591};
t931 = ct{1592};
t932 = ct{1593};
t933 = ct{1594};
t934 = ct{1595};
t935 = ct{1596};
t936 = ct{1597};
t937 = ct{1598};
t938 = ct{1599};
t939 = ct{1600};
t94 = ct{1601};
t940 = ct{1602};
t941 = ct{1603};
t942 = ct{1604};
t943 = ct{1605};
t945 = ct{1606};
t946 = ct{1607};
t947 = ct{1608};
t948 = ct{1609};
t949 = ct{1610};
t950 = ct{1611};
t951 = ct{1612};
t952 = ct{1613};
t953 = ct{1614};
t955 = ct{1615};
t957 = ct{1616};
t958 = ct{1617};
t959 = ct{1618};
t961 = ct{1619};
t963 = ct{1620};
t964 = ct{1621};
t966 = ct{1622};
t967 = ct{1623};
t969 = ct{1624};
t97 = ct{1625};
t972 = ct{1626};
t973 = ct{1627};
t974 = ct{1628};
t975 = ct{1629};
t976 = ct{1630};
t977 = ct{1631};
t978 = ct{1632};
t979 = ct{1633};
t980 = ct{1634};
t982 = ct{1635};
t983 = ct{1636};
t985 = ct{1637};
t986 = ct{1638};
t987 = ct{1639};
t988 = ct{1640};
t992 = ct{1641};
t994 = ct{1642};
t995 = ct{1643};
t997 = ct{1644};
t999 = ct{1645};
t2445 = t2164.*(t88-t617);
t2446 = -t2165.*(t92-t663);
t2460 = t877+t2182;
t2476 = t949+t2179;
t2477 = t892+t2212;
t2486 = -t2481;
t2488 = t948+t2217;
t2497 = -t7.*(t882-t2179);
t2498 = -t14.*(t882-t2179);
t2507 = t952+t2266;
t2513 = t14.*(t882-t2179);
t2519 = t2186.*2.37e-3;
t2520 = dq5.*t2181.*4.74e-3;
t2521 = t994+t2262;
t2522 = t2182.*2.75e-2;
t2523 = t2186.*2.75e-2;
t2530 = t1040.*t2164;
t2537 = t2184.*4.9e-4;
t2541 = t2187.*4.9e-4;
t2545 = -t2526;
t2546 = dq5.*t2181.*5.5e-2;
t2552 = t2181.*5.000000000000001e-5;
t2554 = t2217.*2.75e-2;
t2555 = dq6.*t2180.*9.8e-4;
t2557 = -t2527;
t2560 = t2180.*2.019e-2;
t2561 = t2183.*2.019e-2;
t2563 = t1070.*t2165;
t2564 = -t2550;
t2565 = dq6.*t2184.*4.038e-2;
t2566 = t2219.*4.9e-4;
t2573 = dq5.*t2186.*1.0e-4;
t2581 = dq6.*t2214.*9.8e-4;
t2584 = t322+t810+t857+t1914;
t2585 = t331+t760+t903+t1919;
t2588 = t2214.*2.019e-2;
t2592 = dq6.*t2219.*4.038e-2;
t2596 = -t2582;
t2605 = -t2594;
t2614 = t2267.*3.466000000000001e-2;
t2616 = t2180.*1.9738e-1;
t2617 = t2183.*1.9738e-1;
t2621 = t1206.*t2164;
t2629 = dq7.*t2267.*4.648e-2;
t2630 = t294+t820+t900+t1903;
t2631 = t315+t802+t955+t1907;
t2632 = dq7.*t2263.*6.932000000000001e-2;
t2633 = dq6.*t2184.*3.9476e-1;
t2637 = t2263.*2.324e-2;
t2644 = t2214.*1.9738e-1;
t2648 = -t2619;
t2650 = -t2620;
t2651 = -t2165.*(t621-t864);
t2657 = dq6.*t2219.*3.9476e-1;
t2662 = t15.*t2634;
t2663 = t2266.*1.9738e-1;
t2670 = t8.*t2634;
t2680 = t14.*t2659;
t2681 = -t2673;
t2685 = t7.*t2659;
t2689 = t695+t713+t1050+t1799;
t2692 = t7.*t2672;
t2694 = t14.*t2672;
t2699 = t7.*t2687;
t2700 = t14.*t2687;
t2702 = -t2691;
t2714 = t671+t764+t1074+t1801;
t2717 = -t2709;
t2721 = t627+t807+t1118+t1804;
t2723 = t627+t778+t807+t1113+t1118;
t2728 = t8.*t2707;
t2729 = t15.*t2707;
t2732 = t699+t783+t1229+t1802;
t2733 = t745+t766+t1123+t1805;
t2737 = t7.*t2720;
t2739 = t14.*t2720;
t2741 = t7.*t2722;
t2742 = t14.*t2722;
t2753 = t8.*t2734;
t2754 = t15.*t2734;
t2759 = -t2758;
t2763 = -t2761;
t2764 = -t2762;
t2767 = -t2765;
t2773 = -t2770;
t2777 = t2165.*(t92-t663).*(-4.466636216449161e-20);
t2780 = t2356.*9.999999999999998e-6;
t2783 = t2370.*9.999999999999998e-6;
t2789 = t2350.*3.844e-2;
t2790 = t2351.*3.844e-2;
t2791 = t2356.*2.769999999999999e-3;
t2793 = -t2787;
t2794 = t2356.*1.0e-5;
t2796 = t2350.*1.12e-3;
t2797 = t2351.*1.12e-3;
t2798 = t2350.*8.8e-4;
t2799 = t2351.*8.8e-4;
t2800 = t2370.*2.769999999999999e-3;
t2801 = t2370.*1.0e-5;
t2803 = t2369.*3.844e-2;
t2807 = t2163.*t2164;
t2810 = t2369.*8.8e-4;
t2812 = -t2805;
t2813 = t2369.*1.12e-3;
t2817 = t2165.*t2196;
t2829 = t2412.*1.11e-3;
t2831 = t714+t947+t1128+t2181;
t2835 = t8.*t2822;
t2836 = t15.*t2822;
t2839 = t2618.*4.466636216449161e-20;
t2840 = t2619.*4.466636216449161e-20;
t2841 = t2620.*4.466636216449161e-20;
t2847 = -t2830;
t2848 = -t2834;
t2849 = t2165.*(t92-t663).*(-9.999999999999998e-6);
t2855 = t2165.*(t92-t663).*9.999999999999998e-6;
t2856 = -t7.*(t639-t1128-t2181+dq5.*t13.*(t86-t652));
t2858 = -t8.*(t639-t1128-t2181+dq5.*t13.*(t86-t652));
t2860 = -t14.*(t639-t1128-t2181+dq5.*t13.*(t86-t652));
t2862 = -t15.*(t639-t1128-t2181+dq5.*t13.*(t86-t652));
t2868 = t2412.*1.12e-3;
t2877 = dq6.*t7.*(t639-t1128-t2181+dq5.*t13.*(t86-t652)).*-2.0;
t2879 = dq6.*t14.*(t639-t1128-t2181+dq5.*t13.*(t86-t652)).*-2.0;
t2885 = -t2870;
t2886 = dq6.*t7.*(t639-t1128-t2181+dq5.*t13.*(t86-t652)).*2.0;
t2887 = dq6.*t14.*(t639-t1128-t2181+dq5.*t13.*(t86-t652)).*2.0;
t2895 = -t2891;
t2900 = t2412.*4.988e-2;
t2901 = -t2899;
t2903 = t2165.*(t92-t663).*(-1.2e-4);
t2906 = t2528.*1.11e-3;
t2907 = t2586.*9.999999999999998e-6;
t2909 = t2529.*3.844e-2;
t2910 = t2527.*3.844e-2;
t2911 = t2529.*8.8e-4;
t2913 = t2527.*1.12e-3;
t2916 = t2527.*8.8e-4;
t2917 = t2529.*1.12e-3;
t2918 = t2528.*8.8e-4;
t2922 = t2586.*2.769999999999999e-3;
t2923 = t2586.*1.0e-5;
t2925 = t2165.*(t621-t864).*(-4.000000000000028e-5);
t2930 = t2618.*1.0e-5;
t2931 = t2619.*1.0e-5;
t2933 = t2620.*1.0e-5;
t2934 = t2528.*1.144e-2;
t2936 = t2165.*(t621-t864).*(-5.0e-5);
t2942 = t2165.*(t621-t864).*5.0e-5;
t2945 = t2165.*(t621-t864).*(-2.81e-3);
t2948 = -t831.*(t639-t1128-t2181+dq5.*t13.*(t86-t652));
t2951 = t2165.*(t621-t864).*2.81e-3;
t2954 = t2618.*2.840000000000012e-3;
t2955 = t2619.*2.840000000000012e-3;
t2956 = t2620.*2.840000000000012e-3;
t2958 = -t2854.*(t92-t663);
t2962 = t415+t416+t417+t476+t477+t478+t679+t1242+t2156;
t2964 = t387+t390+t394+t406+t408+t470+t750+t1290+t2192;
t2968 = t7.*t2963;
t2969 = t14.*t2963;
t2974 = t418+t419+t420+t479+t480+t481+t748+t1187+t2292;
t2975 = t15.*t2972;
t2977 = t6.*t2971;
t2978 = t13.*t2971;
t2979 = t8.*t2972;
t2989 = t7.*(t639-t1128-t2181+dq5.*t13.*(t86-t652)).*(-4.9e-4);
t2990 = dq6.*t14.*(t639-t1128-t2181+dq5.*t13.*(t86-t652)).*(-9.8e-4);
t2992 = t14.*(t639-t1128-t2181+dq5.*t13.*(t86-t652)).*(-2.019e-2);
t2994 = t7.*(t639-t1128-t2181+dq5.*t13.*(t86-t652)).*4.9e-4;
t2995 = dq6.*t7.*(t639-t1128-t2181+dq5.*t13.*(t86-t652)).*(-4.038e-2);
t2999 = t1207.*t2822;
t3000 = t15.*(t639-t1128-t2181+dq5.*t13.*(t86-t652)).*(-3.466000000000001e-2);
t3006 = t8.*(t639-t1128-t2181+dq5.*t13.*(t86-t652)).*(-2.324e-2);
t3015 = t572.*t2963;
t3019 = t14.*(t639-t1128-t2181+dq5.*t13.*(t86-t652)).*(-1.9738e-1);
t3026 = t14.*(t639-t1128-t2181+dq5.*t13.*(t86-t652)).*1.9738e-1;
t3028 = dq6.*t7.*(t639-t1128-t2181+dq5.*t13.*(t86-t652)).*(-3.9476e-1);
t3031 = (t614+t13.*(t86-t652)).*(t639-t1128-t2181+dq5.*t13.*(t86-t652));
t3032 = dq6.*t7.*(t639-t1128-t2181+dq5.*t13.*(t86-t652)).*3.9476e-1;
t3034 = t573.*t2972;
t3046 = t2788.*1.11e-3;
t3051 = t831.*t2971;
t3053 = t2788.*1.12e-3;
t3063 = t2788.*4.988e-2;
t3092 = t1295.*t2963;
t3108 = -t2972.*(t621-t864);
t3111 = -t2854.*(t1529+t15.*(t92-t663));
t3114 = -t2147.*(t639-t1128-t2181+dq5.*t13.*(t86-t652));
t3142 = t831.*(t639-t1128-t2181+dq5.*t13.*(t86-t652)).*(-9.999999999999998e-6);
t3150 = t831.*(t639-t1128-t2181+dq5.*t13.*(t86-t652)).*9.999999999999998e-6;
t3175 = t831.*(t639-t1128-t2181+dq5.*t13.*(t86-t652)).*(-2.769999999999999e-3);
t3178 = t831.*(t639-t1128-t2181+dq5.*t13.*(t86-t652)).*(-1.0e-5);
t3180 = t2854.*(t92-t663).*(-3.0e-5);
t3186 = t2854.*(t92-t663).*(-5.0e-5);
t3200 = t2854.*(t92-t663).*(-5.000000000000004e-4);
t3243 = t2147.*(t639-t1128-t2181+dq5.*t13.*(t86-t652)).*(-4.466636216449161e-20);
t3271 = t2972.*(t621-t864).*(-4.000000000000028e-5);
t3275 = t2972.*(t621-t864).*4.000000000000028e-5;
t3276 = t2972.*(t621-t864).*(-5.0e-5);
t3278 = t2972.*(t621-t864).*(-2.81e-3);
t3282 = t2972.*(t621-t864).*2.81e-3;
t3285 = t2854.*(t1529+t15.*(t92-t663)).*(-1.089e-2);
t3286 = t2854.*(t1529+t15.*(t92-t663)).*(-2.9e-4);
t3287 = t2854.*(t1529+t15.*(t92-t663)).*(-2.2e-4);
t3295 = t2147.*(t639-t1128-t2181+dq5.*t13.*(t86-t652)).*(-1.0e-5);
t3297 = t2147.*(t639-t1128-t2181+dq5.*t13.*(t86-t652)).*1.0e-5;
t3309 = t2147.*(t639-t1128-t2181+dq5.*t13.*(t86-t652)).*(-2.840000000000012e-3);
t3364 = t623+t868+t1181+t1182+t1287+t1409+t2226+t2306;
t3628 = t358+t1101+t1102+t1145+t1147+t1184+t1193+t1291+t1292+t1380+t1381+t1382+t1670+t1722+t2043+t2113;
t3640 = t468+t531+t1253+t1293+t1300+t1348+t1349+t1388+t1390+t1430+t1480+t1544+t1545+t1692+t1763+t2016+t2038;
t3641 = t464+t467+t1249+t1250+t1327+t1376+t1377+t1425+t1428+t1432+t1492+t1495+t1496+t1666+t1716+t2120+t2134;
t3667 = t2003+t2150+t2158+t2317+t2353+t2423+t2442+t2453+t2490;
t3668 = t1983+t2099+t2272+t2298+t2344+t2403+t2416+t2480+t2548;
t3780 = t588+t592+t593+t1270+t1364+t1365+t1410+t1436+t1450+t1451+t1490+t1491+t1517+t1518+t1519+t1547+t1548+t1549+t1561+t1562+t1563+t1570+t1571+t1572+t1696+t1744+t2101+t2146+t2518+t2532;
t3781 = t557+t590+t591+t1265+t1356+t1357+t1384+t1385+t1429+t1453+t1474+t1475+t1508+t1509+t1510+t1511+t1512+t1540+t1541+t1542+t1556+t1566+t1567+t1568+t1761+t1793+t2020+t2082+t2607+t2639;
t3816 = t2059+t2121+t2155+t2174+t2175+t2336+t2342+t2408+t2425+t2427+t2428+t2436+t2441+t2493+t2512+t2713+t2725+t2760+t2768+t2779+t2785;
t981 = -t927;
t984 = -t932;
t1088 = dq6.*t1077;
t1090 = -t1059;
t1093 = dq6.*t1081;
t1587 = -t1487;
t1590 = -t1489;
t1617 = -t1578;
t1619 = -t1579;
t1645 = t21.*t1598;
t1732 = t8.*t1681;
t1737 = t15.*t1681;
t1743 = t8.*t1685;
t1745 = t15.*t1685;
t1778 = t731+t1081;
t1809 = t918+t976;
t1810 = t794+t1077;
t1833 = -t1806;
t1845 = -t8.*(t735-t1077);
t1848 = -t15.*(t735-t1077);
t1853 = dq7.*t1844;
t1857 = dq7.*t1847;
t1883 = t15.*(t735-t1077);
t1899 = -t1890;
t1906 = t932.*4.9e-4;
t1923 = t927.*2.019e-2;
t1929 = -t1902;
t1938 = -t1921;
t1939 = -t1922;
t1954 = -t1933;
t1961 = -t1942;
t1993 = t927.*1.9738e-1;
t2021 = t862+t1530;
t2044 = t8.*t2000;
t2046 = t15.*t2000;
t2054 = -t2039;
t2070 = t1059.*3.466000000000001e-2;
t2074 = t860+t1598;
t2080 = t8.*t2035;
t2081 = t15.*t2035;
t2088 = t1062.*2.324e-2;
t2096 = -t2071;
t2176 = t1487.*4.9e-4;
t2191 = t1471.*2.019e-2;
t2198 = t1557.*4.9e-4;
t2203 = t1472.*3.466000000000001e-2;
t2205 = t1582.*4.9e-4;
t2227 = t1578.*2.019e-2;
t2228 = t1488.*2.324e-2;
t2239 = t1564.*2.019e-2;
t2241 = t1606.*4.9e-4;
t2245 = -t2229;
t2246 = t1579.*3.466000000000001e-2;
t2248 = -t2232;
t2250 = -t2236;
t2254 = -t2206;
t2255 = -t2207;
t2264 = -t2218;
t2268 = -t2221;
t2269 = t1584.*2.324e-2;
t2279 = dq5.*t2216.*2.0;
t2281 = dq6.*t2220.*2.0;
t2282 = dq5.*t2222.*2.0;
t2283 = dq6.*t2224.*2.0;
t2286 = t1607.*2.019e-2;
t2287 = -t2240;
t2291 = t1658.*(-3.466000000000001e-2);
t2297 = t1471.*1.9738e-1;
t2302 = -t2261;
t2312 = t1564.*1.9738e-1;
t2319 = t1578.*1.9738e-1;
t2329 = t1607.*1.9738e-1;
t2330 = t911+t1844;
t2346 = t967+t1847;
t2375 = t1806.*3.466000000000001e-2;
t2379 = t1803.*2.324e-2;
t2394 = t1888.*(-3.466000000000001e-2);
t2398 = t1886.*(-2.324e-2);
t2399 = dq7.*t8.*(t735-t1077).*(-2.324e-2);
t2482 = t8.*t2460;
t2483 = t15.*t2460;
t2501 = t7.*t2477;
t2503 = t14.*t2477;
t2514 = t8.*t2488;
t2516 = t15.*t2488;
t2531 = t2222.*2.37e-3;
t2540 = -t2520;
t2543 = -t2523;
t2553 = dq5.*t2216.*4.74e-3;
t2556 = t2222.*2.75e-2;
t2559 = -t2546;
t2562 = -t2530;
t2567 = t2220.*4.9e-4;
t2569 = t2223.*4.9e-4;
t2570 = t8.*t2521;
t2571 = t15.*t2521;
t2574 = dq5.*t2216.*5.5e-2;
t2575 = t2224.*2.019e-2;
t2577 = -t2565;
t2578 = -t2566;
t2580 = t2216.*5.000000000000001e-5;
t2583 = dq6.*t2224.*9.8e-4;
t2589 = -t2563;
t2590 = t2218.*2.019e-2;
t2591 = t2225.*3.466000000000001e-2;
t2593 = dq6.*t2220.*4.038e-2;
t2598 = dq5.*t2222.*1.0e-4;
t2599 = -t2588;
t2602 = -t2592;
t2609 = t316+t822+t856+t1912;
t2610 = t329+t805+t901+t1918;
t2611 = t2221.*2.324e-2;
t2613 = t8.*t2584;
t2615 = t15.*t2584;
t2628 = -t2616;
t2645 = t2218.*1.9738e-1;
t2646 = -t2632;
t2647 = t2224.*1.9738e-1;
t2658 = dq6.*t2220.*3.9476e-1;
t2664 = t7.*t2630;
t2665 = t8.*t2631;
t2666 = t14.*t2630;
t2667 = t15.*t2631;
t2686 = -t2670;
t2695 = -t2685;
t2697 = t7.*t2689;
t2698 = t14.*t2689;
t2704 = -t2694;
t2716 = -t2699;
t2726 = t8.*t2714;
t2727 = t15.*t2714;
t2738 = t8.*t2721;
t2740 = t15.*t2721;
t2743 = t8.*t2723;
t2744 = t15.*t2723;
t2747 = t8.*t2732;
t2749 = -t2739;
t2751 = t15.*t2732;
t2752 = -t2741;
t2781 = t2359.*9.999999999999998e-6;
t2792 = t2359.*2.769999999999999e-3;
t2795 = t2359.*1.0e-5;
t2804 = t2372.*3.844e-2;
t2806 = -t2800;
t2808 = -t2801;
t2809 = -t2803;
t2811 = t2372.*8.8e-4;
t2814 = t2372.*1.12e-3;
t2815 = -t2810;
t2816 = t670+t849+t1076+t2222;
t2818 = t2563.*4.466636216449161e-20;
t2819 = -t2813;
t2821 = -t2817;
t2828 = t712+t893+t1135+t2216;
t2832 = t628+t941+t1117+t2213;
t2842 = t2621.*4.466636216449161e-20;
t2843 = -t2829;
t2850 = t720+t957+t1137+t2220;
t2851 = t675+t885+t1228+t2224;
t2852 = -t2841;
t2853 = t2445.*(-1.11e-3);
t2872 = -t8.*(t642+t896-t1137-t2220);
t2873 = -t8.*(t631-t885+t1132-t2224);
t2874 = -t15.*(t642+t896-t1137-t2220);
t2875 = -t15.*(t631-t885+t1132-t2224);
t2876 = -t2868;
t2888 = t2445.*(-1.12e-3);
t2890 = t8.*(t642+t896-t1137-t2220);
t2893 = dq7.*t15.*(t642+t896-t1137-t2220).*-2.0;
t2902 = -t2900;
t2904 = t2445.*(-4.988e-2);
t2905 = t2530.*1.11e-3;
t2908 = -t2906;
t2912 = t2530.*8.8e-4;
t2914 = t2563.*1.0e-5;
t2915 = -t2910;
t2919 = -t2913;
t2920 = -t2916;
t2921 = -t2918;
t2926 = -t2923;
t2935 = t2621.*1.0e-5;
t2937 = t2530.*1.144e-2;
t2938 = -t2931;
t2939 = -t2933;
t2940 = -t2934;
t2941 = t2563.*2.840000000000012e-3;
t2957 = t2621.*2.840000000000012e-3;
t2959 = -t2956;
t2960 = (t92-t663).*(t642+t896-t1137-t2220);
t2961 = (t92-t663).*(t631-t885+t1132-t2224);
t2965 = t6.*t2962;
t2966 = t13.*t2962;
t2967 = t14.*t2964;
t2970 = t7.*t2964;
t2983 = t7.*t2974;
t2984 = t14.*t2974;
t2987 = -t2977;
t2988 = -t2979;
t3011 = t2817.*4.466636216449161e-20;
t3017 = dq7.*t15.*(t642+t896-t1137-t2220).*(-6.932000000000001e-2);
t3018 = t15.*(t642+t896-t1137-t2220).*(-2.324e-2);
t3023 = dq7.*t15.*(t642+t896-t1137-t2220).*6.932000000000001e-2;
t3025 = -t1207.*(t642+t896-t1137-t2220);
t3027 = -t3015;
t3029 = t604.*t2964;
t3036 = -t3031;
t3037 = -t3034;
t3044 = -t2962.*(t88-t617);
t3049 = -t3046;
t3052 = t2817.*9.999999999999998e-6;
t3054 = t2807.*1.11e-3;
t3056 = -t3053;
t3058 = -t3051;
t3059 = -t2974.*(t92-t663);
t3060 = t1225+t2350+t2377;
t3061 = t2807.*1.12e-3;
t3064 = -t3063;
t3067 = t2817.*1.2e-4;
t3069 = t2807.*4.988e-2;
t3074 = t2969.*4.9e-4;
t3077 = t2968.*2.019e-2;
t3081 = t2978.*2.37e-3;
t3084 = t2978.*2.75e-2;
t3085 = t1206.*t2964;
t3087 = -t2035.*(t639-t1128-t2181+dq5.*t13.*(t86-t652));
t3089 = t2977.*5.000000000000001e-5;
t3094 = t2968.*1.9738e-1;
t3095 = t2975.*3.466000000000001e-2;
t3097 = t811+t978+t1911+t2662;
t3100 = t2979.*2.324e-2;
t3112 = (t1529+t15.*(t92-t663)).*(t642+t896-t1137-t2220);
t3113 = (t1529+t15.*(t92-t663)).*(t631-t885+t1132-t2224);
t3120 = t809+t1013+t1952+t2680;
t3125 = t803+t1035+t1905+t2692;
t3127 = t689+t780+t1089+t1309+t2700;
t3132 = t850+t934+t937+t2223+t2256;
t3135 = -t8.*(-t694+t777+t1161+t1215+t2699);
t3136 = -t15.*(-t694+t777+t1161+t1215+t2699);
t3137 = -t8.*(t755+t1012-t1905-t2692);
t3138 = -t15.*(t755+t1012-t1905-t2692);
t3139 = -t2196.*(t642+t896-t1137-t2220);
t3140 = -t2196.*(t631-t885+t1132-t2224);
t3141 = t698+t700+t1064+t1325+t2753;
t3148 = t15.*(-t694+t777+t1161+t1215+t2699);
t3149 = t2196.*(t631-t885+t1132-t2224);
t3159 = t706+t765+t1092+t1220+t2754;
t3181 = t3031.*4.466636216449161e-20;
t3188 = -t8.*(t932+t942+t2215+t7.*(t882-t2179));
t3189 = -t15.*(t932+t942+t2215+t7.*(t882-t2179));
t3192 = t1630+t2412+t2445;
t3203 = t887+t1016+t1017+t2225+t2300;
t3205 = t2999.*4.000000000000028e-5;
t3206 = t2999.*3.0e-5;
t3209 = t1207.*(t642+t896-t1137-t2220).*(-4.000000000000028e-5);
t3210 = t2999.*2.32e-3;
t3211 = t1207.*(t642+t896-t1137-t2220).*(-3.0e-5);
t3212 = t1207.*(t642+t896-t1137-t2220).*4.000000000000028e-5;
t3213 = t3031.*9.999999999999998e-6;
t3214 = t2974.*(t92-t663).*(-4.466636216449161e-20);
t3215 = t3034.*9.999999999999998e-6;
t3217 = t3015.*3.844e-2;
t3218 = t1207.*(t642+t896-t1137-t2220).*(-2.32e-3);
t3219 = t3015.*1.12e-3;
t3221 = t3015.*8.8e-4;
t3222 = t1207.*(t642+t896-t1137-t2220).*2.32e-3;
t3226 = t3034.*1.0e-5;
t3229 = t3034.*2.769999999999999e-3;
t3232 = t3031.*1.2e-4;
t3234 = t2962.*(t88-t617).*(-1.11e-3);
t3236 = t2962.*(t88-t617).*1.11e-3;
t3238 = t3092.*4.466636216449161e-20;
t3239 = t2962.*(t88-t617).*(-1.12e-3);
t3240 = t2962.*(t88-t617).*1.12e-3;
t3241 = t3051.*1.11e-3;
t3242 = t2974.*(t92-t663).*(-9.999999999999998e-6);
t3244 = t3051.*1.12e-3;
t3245 = t2962.*(t88-t617).*(-4.988e-2);
t3247 = t2962.*(t88-t617).*4.988e-2;
t3251 = t3051.*4.988e-2;
t3254 = t2974.*(t92-t663).*(-1.2e-4);
t3258 = t2035.*(t639-t1128-t2181+dq5.*t13.*(t86-t652)).*(-4.000000000000028e-5);
t3261 = t2035.*(t639-t1128-t2181+dq5.*t13.*(t86-t652)).*(-5.0e-5);
t3266 = t2035.*(t639-t1128-t2181+dq5.*t13.*(t86-t652)).*(-2.81e-3);
t3269 = t3092.*1.0e-5;
t3272 = t1846+t2618+t2650;
C = ft_6({dq1,dq2,dq3,dq4,dq5,dq6,dq7,t10,t1000,t1001,t1003,t1004,t1007,t1008,t1010,t1012,t1013,t1014,t1015,t1016,t1017,t1018,t1019,t1020,t1021,t1022,t1023,t1024,t1025,t1026,t1029,t1031,t1032,t1033,t1034,t1035,t1036,t1038,t1039,t1040,t1041,t1044,t1045,t1046,t105,t1051,t1052,t1053,t1054,t1055,t1056,t1058,t1059,t1060,t1062,t1063,t1064,t1066,t1067,t1069,t107,t1070,t1072,t1075,t1077,t1079,t1081,t1088,t1090,t1091,t1092,t1093,t1094,t1096,t1097,t11,t1103,t1104,t1105,t1106,t1109,t1110,t1113,t1114,t1115,t1119,t112,t1123,t1125,t1126,t1128,t1130,t1132,t1136,t1137,t1138,t1139,t114,t1140,t1141,t1142,t1143,t1144,t1146,t1159,t1161,t1164,t1165,t1166,t1167,t1168,t1169,t1172,t1173,t1174,t1175,t1176,t1177,t1178,t1179,t1180,t1183,t1188,t1189,t119,t1190,t1194,t1195,t1197,t1198,t1199,t12,t1200,t1201,t1202,t1203,t1204,t1205,t1206,t1207,t1208,t1209,t1211,t1212,t1213,t1214,t1215,t1216,t1217,t1218,t1219,t122,t1220,t1224,t1226,t1231,t1232,t1238,t1243,t1244,t1246,t1256,t1257,t1263,t1264,t1267,t1268,t1269,t1273,t1274,t1275,t1286,t1288,t1289,t1295,t1296,t1299,t13,t130,t1304,t1305,t1306,t1312,t1313,t1315,t1318,t1328,t1329,t1330,t1339,t1341,t1342,t1346,t1347,t1350,t1351,t1352,t1360,t1361,t1362,t1363,t1368,t1369,t137,t1374,t1375,t1386,t1387,t1389,t139,t1391,t14,t1412,t1416,t1417,t1418,t1423,t1424,t1431,t1435,t144,t1441,t1449,t1455,t1456,t1462,t1467,t1471,t1472,t1473,t1487,t1488,t1489,t149,t1497,t1498,t15,t1506,t151,t1513,t1515,t1516,t152,t1526,t1527,t1528,t1529,t1537,t1538,t1539,t1543,t1546,t1550,t1551,t1552,t1553,t1554,t1557,t1564,t1565,t1569,t1574,t1577,t1578,t1579,t1581,t1582,t1583,t1584,t1585,t1587,t1589,t1590,t1591,t1596,t16,t160,t1601,t1603,t1604,t1605,t1606,t1608,t1609,t1611,t1612,t1613,t1616,t1617,t1618,t1619,t1622,t1624,t1625,t1626,t1627,t1629,t1633,t1634,t1635,t1636,t1637,t1638,t1642,t1643,t1644,t1645,t1647,t1648,t1649,t165,t1650,t1651,t1652,t1653,t1654,t1655,t1657,t1658,t1659,t1660,t1661,t1662,t1663,t1664,t1667,t1668,t1671,t1672,t1673,t1674,t1675,t1678,t1679,t1680,t1681,t1682,t1683,t1685,t1686,t1687,t1688,t1690,t1691,t1693,t1694,t1697,t1699,t17,t1700,t1701,t1702,t1704,t1705,t1706,t1707,t171,t1710,t1711,t1715,t1717,t1718,t1719,t1720,t1721,t1723,t1725,t1726,t1727,t1729,t1731,t1732,t1734,t1735,t1736,t1737,t1738,t1740,t1742,t1743,t1745,t1746,t1748,t1749,t175,t1751,t1752,t1757,t1759,t1760,t1762,t1765,t1766,t1769,t1770,t1772,t1773,t1774,t1775,t1776,t1778,t1779,t1780,t1782,t1786,t1790,t1791,t1792,t1795,t1798,t1799,t180,t1800,t1801,t1802,t1803,t1804,t1805,t1806,t1807,t1811,t1812,t1813,t1814,t1815,t1816,t1817,t1819,t182,t1822,t1823,t1824,t1825,t1826,t1827,t1828,t1829,t1830,t1831,t1833,t1834,t1835,t1836,t1837,t1839,t1840,t1841,t1842,t1843,t1845,t1846,t1848,t1849,t185,t1850,t1851,t1852,t1853,t1855,t1856,t1857,t1859,t186,t1860,t1861,t1863,t1864,t1865,t1866,t1867,t187,t1871,t1872,t1873,t1874,t1875,t1876,t1877,t1878,t1880,t1881,t1882,t1883,t1884,t1885,t1886,t1887,t1888,t189,t1890,t1891,t1892,t1893,t1896,t1897,t1898,t1899,t1900,t1901,t1902,t1903,t1905,t1906,t1907,t1908,t1909,t1911,t1912,t1913,t1914,t1915,t1917,t1918,t1919,t1923,t1924,t1927,t1928,t1932,t1934,t1935,t1936,t1937,t1938,t1939,t1941,t1942,t1944,t1945,t1946,t1949,t1950,t1951,t1952,t1953,t1954,t1955,t1957,t1959,t1960,t1962,t1963,t1967,t1968,t1969,t1970,t1971,t1974,t1975,t1976,t1977,t1978,t1980,t1982,t1984,t1985,t1986,t1988,t1990,t1992,t1993,t1997,t1998,t2,t2000,t2001,t2002,t2003,t2006,t2008,t2009,t2010,t2011,t2013,t2014,t2015,t2018,t2022,t2023,t2026,t2028,t2029,t2030,t2032,t2033,t2034,t2035,t2036,t2041,t2042,t2044,t2045,t2046,t2047,t2049,t2054,t2056,t2057,t2058,t2060,t2065,t2066,t2070,t2071,t2072,t2073,t2074,t2075,t2077,t2078,t208,t2080,t2081,t2083,t2085,t2086,t2088,t2089,t2093,t2094,t2096,t2098,t2104,t2105,t2109,t2111,t2114,t2117,t2119,t2123,t2125,t2126,t2129,t2130,t2133,t2140,t2141,t2147,t2148,t2149,t2152,t2157,t2160,t2162,t2163,t2164,t2165,t2166,t2167,t2170,t2171,t2172,t2173,t2176,t2177,t2179,t2180,t2181,t2182,t2183,t2184,t2187,t2191,t2193,t2196,t2197,t2198,t22,t2201,t2203,t2204,t2205,t2206,t2207,t2208,t2209,t221,t2210,t2212,t2214,t2215,t2217,t2218,t2219,t2220,t2223,t2224,t2225,t2227,t2228,t223,t2230,t2231,t2233,t2239,t2240,t2241,t2245,t2246,t2248,t2249,t2250,t2251,t2254,t2255,t2256,t2258,t2259,t2260,t2261,t2262,t2263,t2264,t2265,t2266,t2267,t2268,t2269,t2270,t2277,t2278,t2279,t2280,t2281,t2282,t2283,t2284,t2285,t2286,t2287,t2288,t2289,t2290,t2293,t2296,t2297,t23,t230,t2300,t2301,t2302,t2307,t2308,t2309,t231,t2310,t2311,t2312,t2313,t2315,t2316,t2318,t2319,t232,t2327,t2329,t2330,t2331,t2333,t2337,t234,t2341,t2348,t235,t2350,t2351,t2352,t2356,t2357,t2359,t236,t2360,t2361,t2363,t2365,t2368,t2369,t237,t2370,t2372,t2374,t2375,t2376,t2378,t2379,t238,t2380,t2381,t2382,t2384,t2385,t2387,t2388,t239,t2390,t2391,t2393,t2396,t2397,t2399,t24,t240,t2400,t2402,t2404,t2405,t2406,t2407,t2409,t241,t2411,t2414,t2418,t242,t2422,t2424,t2426,t2429,t243,t2431,t2432,t2433,t2435,t2439,t244,t2440,t2443,t2444,t2445,t2446,t2447,t2449,t2451,t2455,t2456,t2458,t2459,t2460,t2462,t2463,t2464,t2466,t2467,t2468,t2469,t2470,t2471,t2472,t2473,t2474,t2475,t2477,t2479,t2482,t2483,t2484,t2486,t2488,t2492,t2494,t2496,t2497,t25,t250,t2501,t2502,t2503,t2506,t2507,t2508,t2509,t251,t2513,t2514,t2516,t2519,t252,t2521,t2522,t2523,t2525,t2528,t2529,t253,t2531,t2533,t2534,t2536,t2537,t2538,t2539,t254,t2540,t2541,t2543,t2545,t2547,t2549,t2551,t2552,t2553,t2554,t2555,t2556,t2557,t2558,t2559,t2560,t2561,t2562,t2563,t2564,t2567,t2569,t2570,t2571,t2572,t2573,t2574,t2575,t2577,t2578,t258,t2580,t2581,t2583,t2584,t2585,t2586,t2589,t259,t2590,t2591,t2593,t2596,t2598,t2599,t26,t2602,t2605,t2606,t2609,t2610,t2611,t2612,t2613,t2614,t2615,t2617,t2618,t2620,t2621,t2622,t2623,t2624,t2628,t2629,t2630,t2631,t2633,t2634,t2635,t2636,t2637,t2638,t2644,t2645,t2646,t2647,t2648,t2651,t2652,t2653,t2657,t2658,t2659,t2662,t2663,t2664,t2665,t2666,t2667,t2668,t267,t2670,t2671,t2672,t2674,t2675,t2677,t2678,t2679,t268,t2680,t2681,t2684,t2685,t2686,t2687,t2689,t269,t2690,t2691,t2692,t2693,t2694,t2695,t2696,t2697,t2698,t2699,t27,t270,t2700,t2701,t2702,t2703,t2704,t2706,t2707,t2708,t271,t2710,t2711,t2712,t2714,t2716,t2717,t2718,t272,t2720,t2721,t2722,t2723,t2726,t2727,t2728,t2729,t273,t2730,t2731,t2732,t2734,t2735,t2737,t2738,t2739,t274,t2740,t2741,t2742,t2743,t2744,t2745,t2747,t2748,t2749,t275,t2751,t2752,t2753,t2754,t2755,t2756,t2757,t2759,t276,t2763,t2764,t2765,t2766,t2767,t277,t2771,t2773,t2774,t2775,t2776,t2777,t2778,t2780,t2781,t2783,t2784,t2786,t2788,t2789,t279,t2790,t2791,t2792,t2793,t2794,t2795,t2796,t2797,t2798,t2799,t28,t280,t2801,t2802,t2803,t2804,t2806,t2807,t2808,t2809,t281,t2810,t2811,t2812,t2813,t2814,t2815,t2816,t2817,t2818,t2819,t282,t2821,t2827,t2828,t2829,t283,t2832,t2833,t2835,t2836,t2839,t284,t2840,t2841,t2842,t2843,t2844,t2847,t2848,t285,t2852,t2853,t2854,t2855,t2856,t2858,t286,t2860,t2862,t2868,t2869,t287,t2873,t2874,t2875,t2876,t288,t2885,t2886,t2887,t2888,t289,t2890,t2891,t2893,t2895,t2897,t2898,t29,t290,t2900,t2901,t2902,t2903,t2904,t2905,t2907,t2908,t2909,t2911,t2912,t2914,t2915,t2917,t2919,t2920,t2921,t2922,t2923,t2924,t2925,t2926,t2929,t293,t2930,t2931,t2935,t2936,t2937,t2939,t2940,t2941,t2942,t2943,t2944,t2945,t2946,t2948,t295,t2952,t2954,t2955,t2956,t2957,t2959,t296,t2960,t2961,t2962,t2965,t2966,t2967,t2968,t2969,t297,t2970,t2972,t2974,t2975,t2978,t2979,t298,t2983,t2984,t2987,t2988,t2989,t2990,t2992,t2994,t2995,t2999,t3,t30,t301,t3011,t3018,t3023,t3025,t3026,t3027,t3029,t3031,t3032,t3036,t3037,t3044,t3049,t3051,t3052,t3054,t3056,t3058,t3059,t3060,t3061,t3064,t3067,t3069,t307,t3074,t3077,t308,t3081,t3084,t3085,t3089,t309,t3092,t3094,t3095,t3097,t31,t310,t3100,t3108,t311,t3112,t3113,t3114,t312,t3120,t313,t3132,t3135,t3137,t3138,t3139,t3140,t3141,t3142,t3148,t3149,t3159,t317,t3175,t318,t3181,t3186,t3188,t3189,t319,t3192,t32,t320,t3203,t3205,t3206,t3210,t3211,t3212,t3213,t3214,t3215,t3217,t3219,t3221,t3222,t3226,t3229,t3232,t3236,t3238,t3240,t3241,t3242,t3243,t3244,t3247,t3248,t3249,t3251,t3252,t3254,t3261,t3269,t327,t3272,t3275,t3276,t328,t3282,t3285,t3286,t3287,t329,t3295,t3297,t33,t330,t3309,t331,t3364,t3372,t338,t34,t342,t3440,t3443,t346,t347,t3476,t348,t349,t35,t358,t36,t3628,t3640,t3641,t3667,t3668,t3669,t3672,t3673,t3679,t37,t3780,t3781,t3816,t39,t4,t40,t427,t428,t429,t43,t431,t432,t433,t434,t435,t436,t438,t439,t441,t442,t443,t444,t446,t448,t45,t450,t451,t452,t453,t455,t456,t457,t458,t459,t46,t460,t461,t463,t464,t465,t466,t467,t468,t469,t483,t484,t49,t494,t495,t496,t5,t50,t51,t510,t511,t512,t515,t516,t517,t518,t522,t523,t524,t525,t526,t527,t528,t529,t530,t531,t533,t534,t535,t536,t537,t538,t542,t543,t545,t546,t547,t548,t549,t55,t550,t551,t552,t553,t554,t556,t557,t558,t561,t562,t563,t564,t565,t566,t567,t568,t569,t57,t570,t571,t572,t573,t574,t575,t576,t577,t578,t579,t58,t580,t581,t582,t583,t584,t585,t586,t587,t588,t589,t590,t591,t592,t593,t594,t595,t596,t597,t598,t599,t6,t600,t601,t602,t603,t604,t605,t606,t607,t608,t609,t61,t612,t613,t614,t615,t616,t617,t618,t619,t620,t621,t622,t624,t626,t629,t63,t631,t632,t633,t634,t635,t637,t639,t64,t640,t642,t643,t644,t646,t647,t648,t649,t650,t651,t652,t653,t654,t656,t657,t658,t660,t661,t662,t663,t664,t665,t667,t67,t673,t676,t677,t678,t680,t681,t683,t684,t685,t686,t687,t688,t689,t69,t691,t692,t693,t694,t696,t697,t698,t7,t70,t700,t701,t702,t703,t704,t705,t706,t707,t708,t71,t72,t721,t722,t723,t724,t725,t726,t728,t729,t73,t730,t731,t735,t74,t740,t743,t75,t751,t753,t754,t755,t756,t757,t758,t759,t76,t760,t762,t769,t77,t770,t773,t774,t776,t777,t778,t779,t78,t782,t785,t786,t787,t788,t79,t791,t792,t795,t796,t797,t799,t8,t80,t800,t803,t805,t806,t809,t81,t811,t812,t813,t814,t815,t816,t817,t818,t819,t82,t821,t827,t83,t831,t834,t835,t836,t837,t838,t839,t84,t840,t841,t842,t843,t845,t846,t847,t848,t85,t850,t851,t853,t854,t855,t856,t857,t859,t86,t860,t863,t864,t866,t867,t87,t870,t871,t872,t873,t876,t877,t878,t88,t880,t881,t882,t883,t884,t885,t887,t888,t889,t89,t890,t891,t894,t895,t896,t897,t898,t899,t9,t90,t900,t902,t904,t905,t907,t908,t91,t911,t92,t921,t922,t923,t926,t927,t928,t930,t931,t932,t933,t935,t936,t937,t938,t939,t94,t940,t942,t943,t945,t946,t948,t949,t950,t951,t952,t953,t958,t959,t961,t963,t964,t966,t969,t97,t972,t973,t974,t975,t977,t978,t979,t980,t981,t982,t983,t984,t985,t986,t987,t988,t992,t994,t995,t997,t999});
end
function C = ft_6(ct)
dq1 = ct{1};
dq2 = ct{2};
dq3 = ct{3};
dq4 = ct{4};
dq5 = ct{5};
dq6 = ct{6};
dq7 = ct{7};
t10 = ct{8};
t1000 = ct{9};
t1001 = ct{10};
t1003 = ct{11};
t1004 = ct{12};
t1007 = ct{13};
t1008 = ct{14};
t1010 = ct{15};
t1012 = ct{16};
t1013 = ct{17};
t1014 = ct{18};
t1015 = ct{19};
t1016 = ct{20};
t1017 = ct{21};
t1018 = ct{22};
t1019 = ct{23};
t1020 = ct{24};
t1021 = ct{25};
t1022 = ct{26};
t1023 = ct{27};
t1024 = ct{28};
t1025 = ct{29};
t1026 = ct{30};
t1029 = ct{31};
t1031 = ct{32};
t1032 = ct{33};
t1033 = ct{34};
t1034 = ct{35};
t1035 = ct{36};
t1036 = ct{37};
t1038 = ct{38};
t1039 = ct{39};
t1040 = ct{40};
t1041 = ct{41};
t1044 = ct{42};
t1045 = ct{43};
t1046 = ct{44};
t105 = ct{45};
t1051 = ct{46};
t1052 = ct{47};
t1053 = ct{48};
t1054 = ct{49};
t1055 = ct{50};
t1056 = ct{51};
t1058 = ct{52};
t1059 = ct{53};
t1060 = ct{54};
t1062 = ct{55};
t1063 = ct{56};
t1064 = ct{57};
t1066 = ct{58};
t1067 = ct{59};
t1069 = ct{60};
t107 = ct{61};
t1070 = ct{62};
t1072 = ct{63};
t1075 = ct{64};
t1077 = ct{65};
t1079 = ct{66};
t1081 = ct{67};
t1088 = ct{68};
t1090 = ct{69};
t1091 = ct{70};
t1092 = ct{71};
t1093 = ct{72};
t1094 = ct{73};
t1096 = ct{74};
t1097 = ct{75};
t11 = ct{76};
t1103 = ct{77};
t1104 = ct{78};
t1105 = ct{79};
t1106 = ct{80};
t1109 = ct{81};
t1110 = ct{82};
t1113 = ct{83};
t1114 = ct{84};
t1115 = ct{85};
t1119 = ct{86};
t112 = ct{87};
t1123 = ct{88};
t1125 = ct{89};
t1126 = ct{90};
t1128 = ct{91};
t1130 = ct{92};
t1132 = ct{93};
t1136 = ct{94};
t1137 = ct{95};
t1138 = ct{96};
t1139 = ct{97};
t114 = ct{98};
t1140 = ct{99};
t1141 = ct{100};
t1142 = ct{101};
t1143 = ct{102};
t1144 = ct{103};
t1146 = ct{104};
t1159 = ct{105};
t1161 = ct{106};
t1164 = ct{107};
t1165 = ct{108};
t1166 = ct{109};
t1167 = ct{110};
t1168 = ct{111};
t1169 = ct{112};
t1172 = ct{113};
t1173 = ct{114};
t1174 = ct{115};
t1175 = ct{116};
t1176 = ct{117};
t1177 = ct{118};
t1178 = ct{119};
t1179 = ct{120};
t1180 = ct{121};
t1183 = ct{122};
t1188 = ct{123};
t1189 = ct{124};
t119 = ct{125};
t1190 = ct{126};
t1194 = ct{127};
t1195 = ct{128};
t1197 = ct{129};
t1198 = ct{130};
t1199 = ct{131};
t12 = ct{132};
t1200 = ct{133};
t1201 = ct{134};
t1202 = ct{135};
t1203 = ct{136};
t1204 = ct{137};
t1205 = ct{138};
t1206 = ct{139};
t1207 = ct{140};
t1208 = ct{141};
t1209 = ct{142};
t1211 = ct{143};
t1212 = ct{144};
t1213 = ct{145};
t1214 = ct{146};
t1215 = ct{147};
t1216 = ct{148};
t1217 = ct{149};
t1218 = ct{150};
t1219 = ct{151};
t122 = ct{152};
t1220 = ct{153};
t1224 = ct{154};
t1226 = ct{155};
t1231 = ct{156};
t1232 = ct{157};
t1238 = ct{158};
t1243 = ct{159};
t1244 = ct{160};
t1246 = ct{161};
t1256 = ct{162};
t1257 = ct{163};
t1263 = ct{164};
t1264 = ct{165};
t1267 = ct{166};
t1268 = ct{167};
t1269 = ct{168};
t1273 = ct{169};
t1274 = ct{170};
t1275 = ct{171};
t1286 = ct{172};
t1288 = ct{173};
t1289 = ct{174};
t1295 = ct{175};
t1296 = ct{176};
t1299 = ct{177};
t13 = ct{178};
t130 = ct{179};
t1304 = ct{180};
t1305 = ct{181};
t1306 = ct{182};
t1312 = ct{183};
t1313 = ct{184};
t1315 = ct{185};
t1318 = ct{186};
t1328 = ct{187};
t1329 = ct{188};
t1330 = ct{189};
t1339 = ct{190};
t1341 = ct{191};
t1342 = ct{192};
t1346 = ct{193};
t1347 = ct{194};
t1350 = ct{195};
t1351 = ct{196};
t1352 = ct{197};
t1360 = ct{198};
t1361 = ct{199};
t1362 = ct{200};
t1363 = ct{201};
t1368 = ct{202};
t1369 = ct{203};
t137 = ct{204};
t1374 = ct{205};
t1375 = ct{206};
t1386 = ct{207};
t1387 = ct{208};
t1389 = ct{209};
t139 = ct{210};
t1391 = ct{211};
t14 = ct{212};
t1412 = ct{213};
t1416 = ct{214};
t1417 = ct{215};
t1418 = ct{216};
t1423 = ct{217};
t1424 = ct{218};
t1431 = ct{219};
t1435 = ct{220};
t144 = ct{221};
t1441 = ct{222};
t1449 = ct{223};
t1455 = ct{224};
t1456 = ct{225};
t1462 = ct{226};
t1467 = ct{227};
t1471 = ct{228};
t1472 = ct{229};
t1473 = ct{230};
t1487 = ct{231};
t1488 = ct{232};
t1489 = ct{233};
t149 = ct{234};
t1497 = ct{235};
t1498 = ct{236};
t15 = ct{237};
t1506 = ct{238};
t151 = ct{239};
t1513 = ct{240};
t1515 = ct{241};
t1516 = ct{242};
t152 = ct{243};
t1526 = ct{244};
t1527 = ct{245};
t1528 = ct{246};
t1529 = ct{247};
t1537 = ct{248};
t1538 = ct{249};
t1539 = ct{250};
t1543 = ct{251};
t1546 = ct{252};
t1550 = ct{253};
t1551 = ct{254};
t1552 = ct{255};
t1553 = ct{256};
t1554 = ct{257};
t1557 = ct{258};
t1564 = ct{259};
t1565 = ct{260};
t1569 = ct{261};
t1574 = ct{262};
t1577 = ct{263};
t1578 = ct{264};
t1579 = ct{265};
t1581 = ct{266};
t1582 = ct{267};
t1583 = ct{268};
t1584 = ct{269};
t1585 = ct{270};
t1587 = ct{271};
t1589 = ct{272};
t1590 = ct{273};
t1591 = ct{274};
t1596 = ct{275};
t16 = ct{276};
t160 = ct{277};
t1601 = ct{278};
t1603 = ct{279};
t1604 = ct{280};
t1605 = ct{281};
t1606 = ct{282};
t1608 = ct{283};
t1609 = ct{284};
t1611 = ct{285};
t1612 = ct{286};
t1613 = ct{287};
t1616 = ct{288};
t1617 = ct{289};
t1618 = ct{290};
t1619 = ct{291};
t1622 = ct{292};
t1624 = ct{293};
t1625 = ct{294};
t1626 = ct{295};
t1627 = ct{296};
t1629 = ct{297};
t1633 = ct{298};
t1634 = ct{299};
t1635 = ct{300};
t1636 = ct{301};
t1637 = ct{302};
t1638 = ct{303};
t1642 = ct{304};
t1643 = ct{305};
t1644 = ct{306};
t1645 = ct{307};
t1647 = ct{308};
t1648 = ct{309};
t1649 = ct{310};
t165 = ct{311};
t1650 = ct{312};
t1651 = ct{313};
t1652 = ct{314};
t1653 = ct{315};
t1654 = ct{316};
t1655 = ct{317};
t1657 = ct{318};
t1658 = ct{319};
t1659 = ct{320};
t1660 = ct{321};
t1661 = ct{322};
t1662 = ct{323};
t1663 = ct{324};
t1664 = ct{325};
t1667 = ct{326};
t1668 = ct{327};
t1671 = ct{328};
t1672 = ct{329};
t1673 = ct{330};
t1674 = ct{331};
t1675 = ct{332};
t1678 = ct{333};
t1679 = ct{334};
t1680 = ct{335};
t1681 = ct{336};
t1682 = ct{337};
t1683 = ct{338};
t1685 = ct{339};
t1686 = ct{340};
t1687 = ct{341};
t1688 = ct{342};
t1690 = ct{343};
t1691 = ct{344};
t1693 = ct{345};
t1694 = ct{346};
t1697 = ct{347};
t1699 = ct{348};
t17 = ct{349};
t1700 = ct{350};
t1701 = ct{351};
t1702 = ct{352};
t1704 = ct{353};
t1705 = ct{354};
t1706 = ct{355};
t1707 = ct{356};
t171 = ct{357};
t1710 = ct{358};
t1711 = ct{359};
t1715 = ct{360};
t1717 = ct{361};
t1718 = ct{362};
t1719 = ct{363};
t1720 = ct{364};
t1721 = ct{365};
t1723 = ct{366};
t1725 = ct{367};
t1726 = ct{368};
t1727 = ct{369};
t1729 = ct{370};
t1731 = ct{371};
t1732 = ct{372};
t1734 = ct{373};
t1735 = ct{374};
t1736 = ct{375};
t1737 = ct{376};
t1738 = ct{377};
t1740 = ct{378};
t1742 = ct{379};
t1743 = ct{380};
t1745 = ct{381};
t1746 = ct{382};
t1748 = ct{383};
t1749 = ct{384};
t175 = ct{385};
t1751 = ct{386};
t1752 = ct{387};
t1757 = ct{388};
t1759 = ct{389};
t1760 = ct{390};
t1762 = ct{391};
t1765 = ct{392};
t1766 = ct{393};
t1769 = ct{394};
t1770 = ct{395};
t1772 = ct{396};
t1773 = ct{397};
t1774 = ct{398};
t1775 = ct{399};
t1776 = ct{400};
t1778 = ct{401};
t1779 = ct{402};
t1780 = ct{403};
t1782 = ct{404};
t1786 = ct{405};
t1790 = ct{406};
t1791 = ct{407};
t1792 = ct{408};
t1795 = ct{409};
t1798 = ct{410};
t1799 = ct{411};
t180 = ct{412};
t1800 = ct{413};
t1801 = ct{414};
t1802 = ct{415};
t1803 = ct{416};
t1804 = ct{417};
t1805 = ct{418};
t1806 = ct{419};
t1807 = ct{420};
t1811 = ct{421};
t1812 = ct{422};
t1813 = ct{423};
t1814 = ct{424};
t1815 = ct{425};
t1816 = ct{426};
t1817 = ct{427};
t1819 = ct{428};
t182 = ct{429};
t1822 = ct{430};
t1823 = ct{431};
t1824 = ct{432};
t1825 = ct{433};
t1826 = ct{434};
t1827 = ct{435};
t1828 = ct{436};
t1829 = ct{437};
t1830 = ct{438};
t1831 = ct{439};
t1833 = ct{440};
t1834 = ct{441};
t1835 = ct{442};
t1836 = ct{443};
t1837 = ct{444};
t1839 = ct{445};
t1840 = ct{446};
t1841 = ct{447};
t1842 = ct{448};
t1843 = ct{449};
t1845 = ct{450};
t1846 = ct{451};
t1848 = ct{452};
t1849 = ct{453};
t185 = ct{454};
t1850 = ct{455};
t1851 = ct{456};
t1852 = ct{457};
t1853 = ct{458};
t1855 = ct{459};
t1856 = ct{460};
t1857 = ct{461};
t1859 = ct{462};
t186 = ct{463};
t1860 = ct{464};
t1861 = ct{465};
t1863 = ct{466};
t1864 = ct{467};
t1865 = ct{468};
t1866 = ct{469};
t1867 = ct{470};
t187 = ct{471};
t1871 = ct{472};
t1872 = ct{473};
t1873 = ct{474};
t1874 = ct{475};
t1875 = ct{476};
t1876 = ct{477};
t1877 = ct{478};
t1878 = ct{479};
t1880 = ct{480};
t1881 = ct{481};
t1882 = ct{482};
t1883 = ct{483};
t1884 = ct{484};
t1885 = ct{485};
t1886 = ct{486};
t1887 = ct{487};
t1888 = ct{488};
t189 = ct{489};
t1890 = ct{490};
t1891 = ct{491};
t1892 = ct{492};
t1893 = ct{493};
t1896 = ct{494};
t1897 = ct{495};
t1898 = ct{496};
t1899 = ct{497};
t1900 = ct{498};
t1901 = ct{499};
t1902 = ct{500};
t1903 = ct{501};
t1905 = ct{502};
t1906 = ct{503};
t1907 = ct{504};
t1908 = ct{505};
t1909 = ct{506};
t1911 = ct{507};
t1912 = ct{508};
t1913 = ct{509};
t1914 = ct{510};
t1915 = ct{511};
t1917 = ct{512};
t1918 = ct{513};
t1919 = ct{514};
t1923 = ct{515};
t1924 = ct{516};
t1927 = ct{517};
t1928 = ct{518};
t1932 = ct{519};
t1934 = ct{520};
t1935 = ct{521};
t1936 = ct{522};
t1937 = ct{523};
t1938 = ct{524};
t1939 = ct{525};
t1941 = ct{526};
t1942 = ct{527};
t1944 = ct{528};
t1945 = ct{529};
t1946 = ct{530};
t1949 = ct{531};
t1950 = ct{532};
t1951 = ct{533};
t1952 = ct{534};
t1953 = ct{535};
t1954 = ct{536};
t1955 = ct{537};
t1957 = ct{538};
t1959 = ct{539};
t1960 = ct{540};
t1962 = ct{541};
t1963 = ct{542};
t1967 = ct{543};
t1968 = ct{544};
t1969 = ct{545};
t1970 = ct{546};
t1971 = ct{547};
t1974 = ct{548};
t1975 = ct{549};
t1976 = ct{550};
t1977 = ct{551};
t1978 = ct{552};
t1980 = ct{553};
t1982 = ct{554};
t1984 = ct{555};
t1985 = ct{556};
t1986 = ct{557};
t1988 = ct{558};
t1990 = ct{559};
t1992 = ct{560};
t1993 = ct{561};
t1997 = ct{562};
t1998 = ct{563};
t2 = ct{564};
t2000 = ct{565};
t2001 = ct{566};
t2002 = ct{567};
t2003 = ct{568};
t2006 = ct{569};
t2008 = ct{570};
t2009 = ct{571};
t2010 = ct{572};
t2011 = ct{573};
t2013 = ct{574};
t2014 = ct{575};
t2015 = ct{576};
t2018 = ct{577};
t2022 = ct{578};
t2023 = ct{579};
t2026 = ct{580};
t2028 = ct{581};
t2029 = ct{582};
t2030 = ct{583};
t2032 = ct{584};
t2033 = ct{585};
t2034 = ct{586};
t2035 = ct{587};
t2036 = ct{588};
t2041 = ct{589};
t2042 = ct{590};
t2044 = ct{591};
t2045 = ct{592};
t2046 = ct{593};
t2047 = ct{594};
t2049 = ct{595};
t2054 = ct{596};
t2056 = ct{597};
t2057 = ct{598};
t2058 = ct{599};
t2060 = ct{600};
t2065 = ct{601};
t2066 = ct{602};
t2070 = ct{603};
t2071 = ct{604};
t2072 = ct{605};
t2073 = ct{606};
t2074 = ct{607};
t2075 = ct{608};
t2077 = ct{609};
t2078 = ct{610};
t208 = ct{611};
t2080 = ct{612};
t2081 = ct{613};
t2083 = ct{614};
t2085 = ct{615};
t2086 = ct{616};
t2088 = ct{617};
t2089 = ct{618};
t2093 = ct{619};
t2094 = ct{620};
t2096 = ct{621};
t2098 = ct{622};
t2104 = ct{623};
t2105 = ct{624};
t2109 = ct{625};
t2111 = ct{626};
t2114 = ct{627};
t2117 = ct{628};
t2119 = ct{629};
t2123 = ct{630};
t2125 = ct{631};
t2126 = ct{632};
t2129 = ct{633};
t2130 = ct{634};
t2133 = ct{635};
t2140 = ct{636};
t2141 = ct{637};
t2147 = ct{638};
t2148 = ct{639};
t2149 = ct{640};
t2152 = ct{641};
t2157 = ct{642};
t2160 = ct{643};
t2162 = ct{644};
t2163 = ct{645};
t2164 = ct{646};
t2165 = ct{647};
t2166 = ct{648};
t2167 = ct{649};
t2170 = ct{650};
t2171 = ct{651};
t2172 = ct{652};
t2173 = ct{653};
t2176 = ct{654};
t2177 = ct{655};
t2179 = ct{656};
t2180 = ct{657};
t2181 = ct{658};
t2182 = ct{659};
t2183 = ct{660};
t2184 = ct{661};
t2187 = ct{662};
t2191 = ct{663};
t2193 = ct{664};
t2196 = ct{665};
t2197 = ct{666};
t2198 = ct{667};
t22 = ct{668};
t2201 = ct{669};
t2203 = ct{670};
t2204 = ct{671};
t2205 = ct{672};
t2206 = ct{673};
t2207 = ct{674};
t2208 = ct{675};
t2209 = ct{676};
t221 = ct{677};
t2210 = ct{678};
t2212 = ct{679};
t2214 = ct{680};
t2215 = ct{681};
t2217 = ct{682};
t2218 = ct{683};
t2219 = ct{684};
t2220 = ct{685};
t2223 = ct{686};
t2224 = ct{687};
t2225 = ct{688};
t2227 = ct{689};
t2228 = ct{690};
t223 = ct{691};
t2230 = ct{692};
t2231 = ct{693};
t2233 = ct{694};
t2239 = ct{695};
t2240 = ct{696};
t2241 = ct{697};
t2245 = ct{698};
t2246 = ct{699};
t2248 = ct{700};
t2249 = ct{701};
t2250 = ct{702};
t2251 = ct{703};
t2254 = ct{704};
t2255 = ct{705};
t2256 = ct{706};
t2258 = ct{707};
t2259 = ct{708};
t2260 = ct{709};
t2261 = ct{710};
t2262 = ct{711};
t2263 = ct{712};
t2264 = ct{713};
t2265 = ct{714};
t2266 = ct{715};
t2267 = ct{716};
t2268 = ct{717};
t2269 = ct{718};
t2270 = ct{719};
t2277 = ct{720};
t2278 = ct{721};
t2279 = ct{722};
t2280 = ct{723};
t2281 = ct{724};
t2282 = ct{725};
t2283 = ct{726};
t2284 = ct{727};
t2285 = ct{728};
t2286 = ct{729};
t2287 = ct{730};
t2288 = ct{731};
t2289 = ct{732};
t2290 = ct{733};
t2293 = ct{734};
t2296 = ct{735};
t2297 = ct{736};
t23 = ct{737};
t230 = ct{738};
t2300 = ct{739};
t2301 = ct{740};
t2302 = ct{741};
t2307 = ct{742};
t2308 = ct{743};
t2309 = ct{744};
t231 = ct{745};
t2310 = ct{746};
t2311 = ct{747};
t2312 = ct{748};
t2313 = ct{749};
t2315 = ct{750};
t2316 = ct{751};
t2318 = ct{752};
t2319 = ct{753};
t232 = ct{754};
t2327 = ct{755};
t2329 = ct{756};
t2330 = ct{757};
t2331 = ct{758};
t2333 = ct{759};
t2337 = ct{760};
t234 = ct{761};
t2341 = ct{762};
t2348 = ct{763};
t235 = ct{764};
t2350 = ct{765};
t2351 = ct{766};
t2352 = ct{767};
t2356 = ct{768};
t2357 = ct{769};
t2359 = ct{770};
t236 = ct{771};
t2360 = ct{772};
t2361 = ct{773};
t2363 = ct{774};
t2365 = ct{775};
t2368 = ct{776};
t2369 = ct{777};
t237 = ct{778};
t2370 = ct{779};
t2372 = ct{780};
t2374 = ct{781};
t2375 = ct{782};
t2376 = ct{783};
t2378 = ct{784};
t2379 = ct{785};
t238 = ct{786};
t2380 = ct{787};
t2381 = ct{788};
t2382 = ct{789};
t2384 = ct{790};
t2385 = ct{791};
t2387 = ct{792};
t2388 = ct{793};
t239 = ct{794};
t2390 = ct{795};
t2391 = ct{796};
t2393 = ct{797};
t2396 = ct{798};
t2397 = ct{799};
t2399 = ct{800};
t24 = ct{801};
t240 = ct{802};
t2400 = ct{803};
t2402 = ct{804};
t2404 = ct{805};
t2405 = ct{806};
t2406 = ct{807};
t2407 = ct{808};
t2409 = ct{809};
t241 = ct{810};
t2411 = ct{811};
t2414 = ct{812};
t2418 = ct{813};
t242 = ct{814};
t2422 = ct{815};
t2424 = ct{816};
t2426 = ct{817};
t2429 = ct{818};
t243 = ct{819};
t2431 = ct{820};
t2432 = ct{821};
t2433 = ct{822};
t2435 = ct{823};
t2439 = ct{824};
t244 = ct{825};
t2440 = ct{826};
t2443 = ct{827};
t2444 = ct{828};
t2445 = ct{829};
t2446 = ct{830};
t2447 = ct{831};
t2449 = ct{832};
t2451 = ct{833};
t2455 = ct{834};
t2456 = ct{835};
t2458 = ct{836};
t2459 = ct{837};
t2460 = ct{838};
t2462 = ct{839};
t2463 = ct{840};
t2464 = ct{841};
t2466 = ct{842};
t2467 = ct{843};
t2468 = ct{844};
t2469 = ct{845};
t2470 = ct{846};
t2471 = ct{847};
t2472 = ct{848};
t2473 = ct{849};
t2474 = ct{850};
t2475 = ct{851};
t2477 = ct{852};
t2479 = ct{853};
t2482 = ct{854};
t2483 = ct{855};
t2484 = ct{856};
t2486 = ct{857};
t2488 = ct{858};
t2492 = ct{859};
t2494 = ct{860};
t2496 = ct{861};
t2497 = ct{862};
t25 = ct{863};
t250 = ct{864};
t2501 = ct{865};
t2502 = ct{866};
t2503 = ct{867};
t2506 = ct{868};
t2507 = ct{869};
t2508 = ct{870};
t2509 = ct{871};
t251 = ct{872};
t2513 = ct{873};
t2514 = ct{874};
t2516 = ct{875};
t2519 = ct{876};
t252 = ct{877};
t2521 = ct{878};
t2522 = ct{879};
t2523 = ct{880};
t2525 = ct{881};
t2528 = ct{882};
t2529 = ct{883};
t253 = ct{884};
t2531 = ct{885};
t2533 = ct{886};
t2534 = ct{887};
t2536 = ct{888};
t2537 = ct{889};
t2538 = ct{890};
t2539 = ct{891};
t254 = ct{892};
t2540 = ct{893};
t2541 = ct{894};
t2543 = ct{895};
t2545 = ct{896};
t2547 = ct{897};
t2549 = ct{898};
t2551 = ct{899};
t2552 = ct{900};
t2553 = ct{901};
t2554 = ct{902};
t2555 = ct{903};
t2556 = ct{904};
t2557 = ct{905};
t2558 = ct{906};
t2559 = ct{907};
t2560 = ct{908};
t2561 = ct{909};
t2562 = ct{910};
t2563 = ct{911};
t2564 = ct{912};
t2567 = ct{913};
t2569 = ct{914};
t2570 = ct{915};
t2571 = ct{916};
t2572 = ct{917};
t2573 = ct{918};
t2574 = ct{919};
t2575 = ct{920};
t2577 = ct{921};
t2578 = ct{922};
t258 = ct{923};
t2580 = ct{924};
t2581 = ct{925};
t2583 = ct{926};
t2584 = ct{927};
t2585 = ct{928};
t2586 = ct{929};
t2589 = ct{930};
t259 = ct{931};
t2590 = ct{932};
t2591 = ct{933};
t2593 = ct{934};
t2596 = ct{935};
t2598 = ct{936};
t2599 = ct{937};
t26 = ct{938};
t2602 = ct{939};
t2605 = ct{940};
t2606 = ct{941};
t2609 = ct{942};
t2610 = ct{943};
t2611 = ct{944};
t2612 = ct{945};
t2613 = ct{946};
t2614 = ct{947};
t2615 = ct{948};
t2617 = ct{949};
t2618 = ct{950};
t2620 = ct{951};
t2621 = ct{952};
t2622 = ct{953};
t2623 = ct{954};
t2624 = ct{955};
t2628 = ct{956};
t2629 = ct{957};
t2630 = ct{958};
t2631 = ct{959};
t2633 = ct{960};
t2634 = ct{961};
t2635 = ct{962};
t2636 = ct{963};
t2637 = ct{964};
t2638 = ct{965};
t2644 = ct{966};
t2645 = ct{967};
t2646 = ct{968};
t2647 = ct{969};
t2648 = ct{970};
t2651 = ct{971};
t2652 = ct{972};
t2653 = ct{973};
t2657 = ct{974};
t2658 = ct{975};
t2659 = ct{976};
t2662 = ct{977};
t2663 = ct{978};
t2664 = ct{979};
t2665 = ct{980};
t2666 = ct{981};
t2667 = ct{982};
t2668 = ct{983};
t267 = ct{984};
t2670 = ct{985};
t2671 = ct{986};
t2672 = ct{987};
t2674 = ct{988};
t2675 = ct{989};
t2677 = ct{990};
t2678 = ct{991};
t2679 = ct{992};
t268 = ct{993};
t2680 = ct{994};
t2681 = ct{995};
t2684 = ct{996};
t2685 = ct{997};
t2686 = ct{998};
t2687 = ct{999};
t2689 = ct{1000};
t269 = ct{1001};
t2690 = ct{1002};
t2691 = ct{1003};
t2692 = ct{1004};
t2693 = ct{1005};
t2694 = ct{1006};
t2695 = ct{1007};
t2696 = ct{1008};
t2697 = ct{1009};
t2698 = ct{1010};
t2699 = ct{1011};
t27 = ct{1012};
t270 = ct{1013};
t2700 = ct{1014};
t2701 = ct{1015};
t2702 = ct{1016};
t2703 = ct{1017};
t2704 = ct{1018};
t2706 = ct{1019};
t2707 = ct{1020};
t2708 = ct{1021};
t271 = ct{1022};
t2710 = ct{1023};
t2711 = ct{1024};
t2712 = ct{1025};
t2714 = ct{1026};
t2716 = ct{1027};
t2717 = ct{1028};
t2718 = ct{1029};
t272 = ct{1030};
t2720 = ct{1031};
t2721 = ct{1032};
t2722 = ct{1033};
t2723 = ct{1034};
t2726 = ct{1035};
t2727 = ct{1036};
t2728 = ct{1037};
t2729 = ct{1038};
t273 = ct{1039};
t2730 = ct{1040};
t2731 = ct{1041};
t2732 = ct{1042};
t2734 = ct{1043};
t2735 = ct{1044};
t2737 = ct{1045};
t2738 = ct{1046};
t2739 = ct{1047};
t274 = ct{1048};
t2740 = ct{1049};
t2741 = ct{1050};
t2742 = ct{1051};
t2743 = ct{1052};
t2744 = ct{1053};
t2745 = ct{1054};
t2747 = ct{1055};
t2748 = ct{1056};
t2749 = ct{1057};
t275 = ct{1058};
t2751 = ct{1059};
t2752 = ct{1060};
t2753 = ct{1061};
t2754 = ct{1062};
t2755 = ct{1063};
t2756 = ct{1064};
t2757 = ct{1065};
t2759 = ct{1066};
t276 = ct{1067};
t2763 = ct{1068};
t2764 = ct{1069};
t2765 = ct{1070};
t2766 = ct{1071};
t2767 = ct{1072};
t277 = ct{1073};
t2771 = ct{1074};
t2773 = ct{1075};
t2774 = ct{1076};
t2775 = ct{1077};
t2776 = ct{1078};
t2777 = ct{1079};
t2778 = ct{1080};
t2780 = ct{1081};
t2781 = ct{1082};
t2783 = ct{1083};
t2784 = ct{1084};
t2786 = ct{1085};
t2788 = ct{1086};
t2789 = ct{1087};
t279 = ct{1088};
t2790 = ct{1089};
t2791 = ct{1090};
t2792 = ct{1091};
t2793 = ct{1092};
t2794 = ct{1093};
t2795 = ct{1094};
t2796 = ct{1095};
t2797 = ct{1096};
t2798 = ct{1097};
t2799 = ct{1098};
t28 = ct{1099};
t280 = ct{1100};
t2801 = ct{1101};
t2802 = ct{1102};
t2803 = ct{1103};
t2804 = ct{1104};
t2806 = ct{1105};
t2807 = ct{1106};
t2808 = ct{1107};
t2809 = ct{1108};
t281 = ct{1109};
t2810 = ct{1110};
t2811 = ct{1111};
t2812 = ct{1112};
t2813 = ct{1113};
t2814 = ct{1114};
t2815 = ct{1115};
t2816 = ct{1116};
t2817 = ct{1117};
t2818 = ct{1118};
t2819 = ct{1119};
t282 = ct{1120};
t2821 = ct{1121};
t2827 = ct{1122};
t2828 = ct{1123};
t2829 = ct{1124};
t283 = ct{1125};
t2832 = ct{1126};
t2833 = ct{1127};
t2835 = ct{1128};
t2836 = ct{1129};
t2839 = ct{1130};
t284 = ct{1131};
t2840 = ct{1132};
t2841 = ct{1133};
t2842 = ct{1134};
t2843 = ct{1135};
t2844 = ct{1136};
t2847 = ct{1137};
t2848 = ct{1138};
t285 = ct{1139};
t2852 = ct{1140};
t2853 = ct{1141};
t2854 = ct{1142};
t2855 = ct{1143};
t2856 = ct{1144};
t2858 = ct{1145};
t286 = ct{1146};
t2860 = ct{1147};
t2862 = ct{1148};
t2868 = ct{1149};
t2869 = ct{1150};
t287 = ct{1151};
t2873 = ct{1152};
t2874 = ct{1153};
t2875 = ct{1154};
t2876 = ct{1155};
t288 = ct{1156};
t2885 = ct{1157};
t2886 = ct{1158};
t2887 = ct{1159};
t2888 = ct{1160};
t289 = ct{1161};
t2890 = ct{1162};
t2891 = ct{1163};
t2893 = ct{1164};
t2895 = ct{1165};
t2897 = ct{1166};
t2898 = ct{1167};
t29 = ct{1168};
t290 = ct{1169};
t2900 = ct{1170};
t2901 = ct{1171};
t2902 = ct{1172};
t2903 = ct{1173};
t2904 = ct{1174};
t2905 = ct{1175};
t2907 = ct{1176};
t2908 = ct{1177};
t2909 = ct{1178};
t2911 = ct{1179};
t2912 = ct{1180};
t2914 = ct{1181};
t2915 = ct{1182};
t2917 = ct{1183};
t2919 = ct{1184};
t2920 = ct{1185};
t2921 = ct{1186};
t2922 = ct{1187};
t2923 = ct{1188};
t2924 = ct{1189};
t2925 = ct{1190};
t2926 = ct{1191};
t2929 = ct{1192};
t293 = ct{1193};
t2930 = ct{1194};
t2931 = ct{1195};
t2935 = ct{1196};
t2936 = ct{1197};
t2937 = ct{1198};
t2939 = ct{1199};
t2940 = ct{1200};
t2941 = ct{1201};
t2942 = ct{1202};
t2943 = ct{1203};
t2944 = ct{1204};
t2945 = ct{1205};
t2946 = ct{1206};
t2948 = ct{1207};
t295 = ct{1208};
t2952 = ct{1209};
t2954 = ct{1210};
t2955 = ct{1211};
t2956 = ct{1212};
t2957 = ct{1213};
t2959 = ct{1214};
t296 = ct{1215};
t2960 = ct{1216};
t2961 = ct{1217};
t2962 = ct{1218};
t2965 = ct{1219};
t2966 = ct{1220};
t2967 = ct{1221};
t2968 = ct{1222};
t2969 = ct{1223};
t297 = ct{1224};
t2970 = ct{1225};
t2972 = ct{1226};
t2974 = ct{1227};
t2975 = ct{1228};
t2978 = ct{1229};
t2979 = ct{1230};
t298 = ct{1231};
t2983 = ct{1232};
t2984 = ct{1233};
t2987 = ct{1234};
t2988 = ct{1235};
t2989 = ct{1236};
t2990 = ct{1237};
t2992 = ct{1238};
t2994 = ct{1239};
t2995 = ct{1240};
t2999 = ct{1241};
t3 = ct{1242};
t30 = ct{1243};
t301 = ct{1244};
t3011 = ct{1245};
t3018 = ct{1246};
t3023 = ct{1247};
t3025 = ct{1248};
t3026 = ct{1249};
t3027 = ct{1250};
t3029 = ct{1251};
t3031 = ct{1252};
t3032 = ct{1253};
t3036 = ct{1254};
t3037 = ct{1255};
t3044 = ct{1256};
t3049 = ct{1257};
t3051 = ct{1258};
t3052 = ct{1259};
t3054 = ct{1260};
t3056 = ct{1261};
t3058 = ct{1262};
t3059 = ct{1263};
t3060 = ct{1264};
t3061 = ct{1265};
t3064 = ct{1266};
t3067 = ct{1267};
t3069 = ct{1268};
t307 = ct{1269};
t3074 = ct{1270};
t3077 = ct{1271};
t308 = ct{1272};
t3081 = ct{1273};
t3084 = ct{1274};
t3085 = ct{1275};
t3089 = ct{1276};
t309 = ct{1277};
t3092 = ct{1278};
t3094 = ct{1279};
t3095 = ct{1280};
t3097 = ct{1281};
t31 = ct{1282};
t310 = ct{1283};
t3100 = ct{1284};
t3108 = ct{1285};
t311 = ct{1286};
t3112 = ct{1287};
t3113 = ct{1288};
t3114 = ct{1289};
t312 = ct{1290};
t3120 = ct{1291};
t313 = ct{1292};
t3132 = ct{1293};
t3135 = ct{1294};
t3137 = ct{1295};
t3138 = ct{1296};
t3139 = ct{1297};
t3140 = ct{1298};
t3141 = ct{1299};
t3142 = ct{1300};
t3148 = ct{1301};
t3149 = ct{1302};
t3159 = ct{1303};
t317 = ct{1304};
t3175 = ct{1305};
t318 = ct{1306};
t3181 = ct{1307};
t3186 = ct{1308};
t3188 = ct{1309};
t3189 = ct{1310};
t319 = ct{1311};
t3192 = ct{1312};
t32 = ct{1313};
t320 = ct{1314};
t3203 = ct{1315};
t3205 = ct{1316};
t3206 = ct{1317};
t3210 = ct{1318};
t3211 = ct{1319};
t3212 = ct{1320};
t3213 = ct{1321};
t3214 = ct{1322};
t3215 = ct{1323};
t3217 = ct{1324};
t3219 = ct{1325};
t3221 = ct{1326};
t3222 = ct{1327};
t3226 = ct{1328};
t3229 = ct{1329};
t3232 = ct{1330};
t3236 = ct{1331};
t3238 = ct{1332};
t3240 = ct{1333};
t3241 = ct{1334};
t3242 = ct{1335};
t3243 = ct{1336};
t3244 = ct{1337};
t3247 = ct{1338};
t3248 = ct{1339};
t3249 = ct{1340};
t3251 = ct{1341};
t3252 = ct{1342};
t3254 = ct{1343};
t3261 = ct{1344};
t3269 = ct{1345};
t327 = ct{1346};
t3272 = ct{1347};
t3275 = ct{1348};
t3276 = ct{1349};
t328 = ct{1350};
t3282 = ct{1351};
t3285 = ct{1352};
t3286 = ct{1353};
t3287 = ct{1354};
t329 = ct{1355};
t3295 = ct{1356};
t3297 = ct{1357};
t33 = ct{1358};
t330 = ct{1359};
t3309 = ct{1360};
t331 = ct{1361};
t3364 = ct{1362};
t3372 = ct{1363};
t338 = ct{1364};
t34 = ct{1365};
t342 = ct{1366};
t3440 = ct{1367};
t3443 = ct{1368};
t346 = ct{1369};
t347 = ct{1370};
t3476 = ct{1371};
t348 = ct{1372};
t349 = ct{1373};
t35 = ct{1374};
t358 = ct{1375};
t36 = ct{1376};
t3628 = ct{1377};
t3640 = ct{1378};
t3641 = ct{1379};
t3667 = ct{1380};
t3668 = ct{1381};
t3669 = ct{1382};
t3672 = ct{1383};
t3673 = ct{1384};
t3679 = ct{1385};
t37 = ct{1386};
t3780 = ct{1387};
t3781 = ct{1388};
t3816 = ct{1389};
t39 = ct{1390};
t4 = ct{1391};
t40 = ct{1392};
t427 = ct{1393};
t428 = ct{1394};
t429 = ct{1395};
t43 = ct{1396};
t431 = ct{1397};
t432 = ct{1398};
t433 = ct{1399};
t434 = ct{1400};
t435 = ct{1401};
t436 = ct{1402};
t438 = ct{1403};
t439 = ct{1404};
t441 = ct{1405};
t442 = ct{1406};
t443 = ct{1407};
t444 = ct{1408};
t446 = ct{1409};
t448 = ct{1410};
t45 = ct{1411};
t450 = ct{1412};
t451 = ct{1413};
t452 = ct{1414};
t453 = ct{1415};
t455 = ct{1416};
t456 = ct{1417};
t457 = ct{1418};
t458 = ct{1419};
t459 = ct{1420};
t46 = ct{1421};
t460 = ct{1422};
t461 = ct{1423};
t463 = ct{1424};
t464 = ct{1425};
t465 = ct{1426};
t466 = ct{1427};
t467 = ct{1428};
t468 = ct{1429};
t469 = ct{1430};
t483 = ct{1431};
t484 = ct{1432};
t49 = ct{1433};
t494 = ct{1434};
t495 = ct{1435};
t496 = ct{1436};
t5 = ct{1437};
t50 = ct{1438};
t51 = ct{1439};
t510 = ct{1440};
t511 = ct{1441};
t512 = ct{1442};
t515 = ct{1443};
t516 = ct{1444};
t517 = ct{1445};
t518 = ct{1446};
t522 = ct{1447};
t523 = ct{1448};
t524 = ct{1449};
t525 = ct{1450};
t526 = ct{1451};
t527 = ct{1452};
t528 = ct{1453};
t529 = ct{1454};
t530 = ct{1455};
t531 = ct{1456};
t533 = ct{1457};
t534 = ct{1458};
t535 = ct{1459};
t536 = ct{1460};
t537 = ct{1461};
t538 = ct{1462};
t542 = ct{1463};
t543 = ct{1464};
t545 = ct{1465};
t546 = ct{1466};
t547 = ct{1467};
t548 = ct{1468};
t549 = ct{1469};
t55 = ct{1470};
t550 = ct{1471};
t551 = ct{1472};
t552 = ct{1473};
t553 = ct{1474};
t554 = ct{1475};
t556 = ct{1476};
t557 = ct{1477};
t558 = ct{1478};
t561 = ct{1479};
t562 = ct{1480};
t563 = ct{1481};
t564 = ct{1482};
t565 = ct{1483};
t566 = ct{1484};
t567 = ct{1485};
t568 = ct{1486};
t569 = ct{1487};
t57 = ct{1488};
t570 = ct{1489};
t571 = ct{1490};
t572 = ct{1491};
t573 = ct{1492};
t574 = ct{1493};
t575 = ct{1494};
t576 = ct{1495};
t577 = ct{1496};
t578 = ct{1497};
t579 = ct{1498};
t58 = ct{1499};
t580 = ct{1500};
t581 = ct{1501};
t582 = ct{1502};
t583 = ct{1503};
t584 = ct{1504};
t585 = ct{1505};
t586 = ct{1506};
t587 = ct{1507};
t588 = ct{1508};
t589 = ct{1509};
t590 = ct{1510};
t591 = ct{1511};
t592 = ct{1512};
t593 = ct{1513};
t594 = ct{1514};
t595 = ct{1515};
t596 = ct{1516};
t597 = ct{1517};
t598 = ct{1518};
t599 = ct{1519};
t6 = ct{1520};
t600 = ct{1521};
t601 = ct{1522};
t602 = ct{1523};
t603 = ct{1524};
t604 = ct{1525};
t605 = ct{1526};
t606 = ct{1527};
t607 = ct{1528};
t608 = ct{1529};
t609 = ct{1530};
t61 = ct{1531};
t612 = ct{1532};
t613 = ct{1533};
t614 = ct{1534};
t615 = ct{1535};
t616 = ct{1536};
t617 = ct{1537};
t618 = ct{1538};
t619 = ct{1539};
t620 = ct{1540};
t621 = ct{1541};
t622 = ct{1542};
t624 = ct{1543};
t626 = ct{1544};
t629 = ct{1545};
t63 = ct{1546};
t631 = ct{1547};
t632 = ct{1548};
t633 = ct{1549};
t634 = ct{1550};
t635 = ct{1551};
t637 = ct{1552};
t639 = ct{1553};
t64 = ct{1554};
t640 = ct{1555};
t642 = ct{1556};
t643 = ct{1557};
t644 = ct{1558};
t646 = ct{1559};
t647 = ct{1560};
t648 = ct{1561};
t649 = ct{1562};
t650 = ct{1563};
t651 = ct{1564};
t652 = ct{1565};
t653 = ct{1566};
t654 = ct{1567};
t656 = ct{1568};
t657 = ct{1569};
t658 = ct{1570};
t660 = ct{1571};
t661 = ct{1572};
t662 = ct{1573};
t663 = ct{1574};
t664 = ct{1575};
t665 = ct{1576};
t667 = ct{1577};
t67 = ct{1578};
t673 = ct{1579};
t676 = ct{1580};
t677 = ct{1581};
t678 = ct{1582};
t680 = ct{1583};
t681 = ct{1584};
t683 = ct{1585};
t684 = ct{1586};
t685 = ct{1587};
t686 = ct{1588};
t687 = ct{1589};
t688 = ct{1590};
t689 = ct{1591};
t69 = ct{1592};
t691 = ct{1593};
t692 = ct{1594};
t693 = ct{1595};
t694 = ct{1596};
t696 = ct{1597};
t697 = ct{1598};
t698 = ct{1599};
t7 = ct{1600};
t70 = ct{1601};
t700 = ct{1602};
t701 = ct{1603};
t702 = ct{1604};
t703 = ct{1605};
t704 = ct{1606};
t705 = ct{1607};
t706 = ct{1608};
t707 = ct{1609};
t708 = ct{1610};
t71 = ct{1611};
t72 = ct{1612};
t721 = ct{1613};
t722 = ct{1614};
t723 = ct{1615};
t724 = ct{1616};
t725 = ct{1617};
t726 = ct{1618};
t728 = ct{1619};
t729 = ct{1620};
t73 = ct{1621};
t730 = ct{1622};
t731 = ct{1623};
t735 = ct{1624};
t74 = ct{1625};
t740 = ct{1626};
t743 = ct{1627};
t75 = ct{1628};
t751 = ct{1629};
t753 = ct{1630};
t754 = ct{1631};
t755 = ct{1632};
t756 = ct{1633};
t757 = ct{1634};
t758 = ct{1635};
t759 = ct{1636};
t76 = ct{1637};
t760 = ct{1638};
t762 = ct{1639};
t769 = ct{1640};
t77 = ct{1641};
t770 = ct{1642};
t773 = ct{1643};
t774 = ct{1644};
t776 = ct{1645};
t777 = ct{1646};
t778 = ct{1647};
t779 = ct{1648};
t78 = ct{1649};
t782 = ct{1650};
t785 = ct{1651};
t786 = ct{1652};
t787 = ct{1653};
t788 = ct{1654};
t79 = ct{1655};
t791 = ct{1656};
t792 = ct{1657};
t795 = ct{1658};
t796 = ct{1659};
t797 = ct{1660};
t799 = ct{1661};
t8 = ct{1662};
t80 = ct{1663};
t800 = ct{1664};
t803 = ct{1665};
t805 = ct{1666};
t806 = ct{1667};
t809 = ct{1668};
t81 = ct{1669};
t811 = ct{1670};
t812 = ct{1671};
t813 = ct{1672};
t814 = ct{1673};
t815 = ct{1674};
t816 = ct{1675};
t817 = ct{1676};
t818 = ct{1677};
t819 = ct{1678};
t82 = ct{1679};
t821 = ct{1680};
t827 = ct{1681};
t83 = ct{1682};
t831 = ct{1683};
t834 = ct{1684};
t835 = ct{1685};
t836 = ct{1686};
t837 = ct{1687};
t838 = ct{1688};
t839 = ct{1689};
t84 = ct{1690};
t840 = ct{1691};
t841 = ct{1692};
t842 = ct{1693};
t843 = ct{1694};
t845 = ct{1695};
t846 = ct{1696};
t847 = ct{1697};
t848 = ct{1698};
t85 = ct{1699};
t850 = ct{1700};
t851 = ct{1701};
t853 = ct{1702};
t854 = ct{1703};
t855 = ct{1704};
t856 = ct{1705};
t857 = ct{1706};
t859 = ct{1707};
t86 = ct{1708};
t860 = ct{1709};
t863 = ct{1710};
t864 = ct{1711};
t866 = ct{1712};
t867 = ct{1713};
t87 = ct{1714};
t870 = ct{1715};
t871 = ct{1716};
t872 = ct{1717};
t873 = ct{1718};
t876 = ct{1719};
t877 = ct{1720};
t878 = ct{1721};
t88 = ct{1722};
t880 = ct{1723};
t881 = ct{1724};
t882 = ct{1725};
t883 = ct{1726};
t884 = ct{1727};
t885 = ct{1728};
t887 = ct{1729};
t888 = ct{1730};
t889 = ct{1731};
t89 = ct{1732};
t890 = ct{1733};
t891 = ct{1734};
t894 = ct{1735};
t895 = ct{1736};
t896 = ct{1737};
t897 = ct{1738};
t898 = ct{1739};
t899 = ct{1740};
t9 = ct{1741};
t90 = ct{1742};
t900 = ct{1743};
t902 = ct{1744};
t904 = ct{1745};
t905 = ct{1746};
t907 = ct{1747};
t908 = ct{1748};
t91 = ct{1749};
t911 = ct{1750};
t92 = ct{1751};
t921 = ct{1752};
t922 = ct{1753};
t923 = ct{1754};
t926 = ct{1755};
t927 = ct{1756};
t928 = ct{1757};
t930 = ct{1758};
t931 = ct{1759};
t932 = ct{1760};
t933 = ct{1761};
t935 = ct{1762};
t936 = ct{1763};
t937 = ct{1764};
t938 = ct{1765};
t939 = ct{1766};
t94 = ct{1767};
t940 = ct{1768};
t942 = ct{1769};
t943 = ct{1770};
t945 = ct{1771};
t946 = ct{1772};
t948 = ct{1773};
t949 = ct{1774};
t950 = ct{1775};
t951 = ct{1776};
t952 = ct{1777};
t953 = ct{1778};
t958 = ct{1779};
t959 = ct{1780};
t961 = ct{1781};
t963 = ct{1782};
t964 = ct{1783};
t966 = ct{1784};
t969 = ct{1785};
t97 = ct{1786};
t972 = ct{1787};
t973 = ct{1788};
t974 = ct{1789};
t975 = ct{1790};
t977 = ct{1791};
t978 = ct{1792};
t979 = ct{1793};
t980 = ct{1794};
t981 = ct{1795};
t982 = ct{1796};
t983 = ct{1797};
t984 = ct{1798};
t985 = ct{1799};
t986 = ct{1800};
t987 = ct{1801};
t988 = ct{1802};
t992 = ct{1803};
t994 = ct{1804};
t995 = ct{1805};
t997 = ct{1806};
t999 = ct{1807};
t3292 = t3092.*2.840000000000012e-3;
t3299 = t2196.*(t642+t896-t1137-t2220).*(-4.000000000000028e-5);
t3302 = t2196.*(t642+t896-t1137-t2220).*4.000000000000028e-5;
t3304 = t2196.*(t642+t896-t1137-t2220).*(-5.0e-5);
t3308 = t2196.*(t642+t896-t1137-t2220).*(-2.81e-3);
t3310 = t2196.*(t642+t896-t1137-t2220).*2.81e-3;
t3313 = t848+t1624+t2260+t2835;
t3314 = t851+t1659+t2209+t2836;
t3318 = t943+t1582+t2210+t2856;
t3320 = -t8.*(t878-t1582+t2184+t7.*(t639-t1128-t2181+dq5.*t13.*(t86-t652)));
t3321 = -t8.*(t884+t1578-t2180+t14.*(t639-t1128-t2181+dq5.*t13.*(t86-t652)));
t3322 = -t15.*(t878-t1582+t2184+t7.*(t639-t1128-t2181+dq5.*t13.*(t86-t652)));
t3323 = -t15.*(t884+t1578-t2180+t14.*(t639-t1128-t2181+dq5.*t13.*(t86-t652)));
t3329 = t15.*(t878-t1582+t2184+t7.*(t639-t1128-t2181+dq5.*t13.*(t86-t652)));
t3331 = dq7.*t8.*(t878-t1582+t2184+t7.*(t639-t1128-t2181+dq5.*t13.*(t86-t652))).*-2.0;
t3339 = (t631-t885+t1132-t2224).*(t642+t896-t1137-t2220);
t3343 = t8.*(t878-t1582+t2184+t7.*(t639-t1128-t2181+dq5.*t13.*(t86-t652))).*(-3.466000000000001e-2);
t3344 = dq7.*t8.*(t878-t1582+t2184+t7.*(t639-t1128-t2181+dq5.*t13.*(t86-t652))).*(-4.648e-2);
t3351 = dq7.*t8.*(t878-t1582+t2184+t7.*(t639-t1128-t2181+dq5.*t13.*(t86-t652))).*4.648e-2;
t3357 = (t614+t13.*(t86-t652)).*(t878-t1582+t2184+t7.*(t639-t1128-t2181+dq5.*t13.*(t86-t652)));
t3358 = (t614+t13.*(t86-t652)).*(t884+t1578-t2180+t14.*(t639-t1128-t2181+dq5.*t13.*(t86-t652)));
t3359 = -t1207.*(t958-t2263+dq7.*t1601+t15.*(t642+t896-t1137-t2220));
t3365 = t1207.*(t958-t2263+dq7.*t1601+t15.*(t642+t896-t1137-t2220));
t3522 = (t958-t2263+dq7.*t1601+t15.*(t642+t896-t1137-t2220)).*(t631-t885+t1132-t2224);
t3622 = (t878-t1582+t2184+t7.*(t639-t1128-t2181+dq5.*t13.*(t86-t652))).*(t884+t1578-t2180+t14.*(t639-t1128-t2181+dq5.*t13.*(t86-t652)));
t3671 = t460+t537+t1139+t1173+t1176+t1637+t1653+t1691+t1887+t1937+t1968+t2057+t2117+t2519+t2552;
t3779 = t496+t1105+t1106+t1109+t1168+t1169+t1195+t1202+t1204+t1205+t1257+t1305+t1306+t1361+t1362+t1363+t1537+t1538+t1539+t1550+t1551+t1552+t1690+t1757+t2083+t2123+t2564+t2605;
t3811 = t1990+t2015+t2129+t2284+t2285+t2318+t2361+t2381+t2390+t2405+t2406+t2422+t2426+t2468+t2479+t2745+t2755+t2759+t2764+t2786+t2802;
t3812 = t2023+t2030+t2162+t2166+t2167+t2331+t2337+t2396+t2397+t2432+t2433+t2449+t2451+t2484+t2502+t2712+t2731+t2763+t2773+t2778+t2784;
t1158 = -t1088;
t1160 = -t1093;
t1750 = dq7.*t1737;
t1753 = dq7.*t1743;
t1755 = dq7.*t1745;
t1771 = dq7.*t1732;
t1783 = -t1745;
t1854 = dq7.*t1845;
t1858 = dq7.*t1848;
t1889 = dq7.*t1883;
t1931 = -t1906;
t1940 = -t1923;
t2005 = -t1993;
t2051 = t1093.*4.9e-4;
t2064 = dq7.*t2044;
t2067 = dq7.*t2046;
t2090 = t1088.*2.019e-2;
t2095 = -t2070;
t2100 = t22.*t2044;
t2103 = t22.*t2046;
t2108 = t2074.^2;
t2110 = dq7.*t2080;
t2112 = dq7.*t2081;
t2132 = t22.*t2081;
t2138 = dq7.*t8.*t2074;
t2139 = dq7.*t15.*t2074;
t2142 = t22.*t2080;
t2151 = t1088.*1.9738e-1;
t2195 = -t2176;
t2200 = -t2191;
t2234 = -t2203;
t2237 = -t2205;
t2242 = -t2227;
t2253 = -t2239;
t2257 = -t2241;
t2276 = -t2246;
t2294 = -t2279;
t2295 = -t2281;
t2323 = t1032+t1743;
t2326 = t1029+t1732;
t2339 = -t2329;
t2343 = t1044+t1737;
t2383 = t1054+t1845;
t2392 = t1051+t1883;
t2499 = -t2483;
t2515 = -t2503;
t2568 = -t2553;
t2576 = t1527+t2046;
t2579 = -t2567;
t2587 = -t2574;
t2597 = -t2583;
t2600 = -t2591;
t2601 = t1604+t2044;
t2603 = -t2593;
t2625 = -t2611;
t2627 = t1596+t2081;
t2640 = t7.*t2609;
t2641 = t8.*t2610;
t2642 = t14.*t2609;
t2643 = t15.*t2610;
t2654 = t1635+t2080;
t2655 = -t2645;
t2669 = -t2658;
t2682 = -t2666;
t2683 = -t2667;
t2715 = -t2698;
t2736 = -t2727;
t2750 = -t2740;
t2782 = -t2781;
t2820 = -t2818;
t2823 = t7.*t2816;
t2824 = t8.*t2816;
t2825 = t14.*t2816;
t2826 = t15.*t2816;
t2857 = t7.*t2832;
t2859 = t8.*t2832;
t2861 = t14.*t2832;
t2863 = t15.*t2832;
t2864 = t7.*t2828;
t2865 = t8.*t2828;
t2866 = t14.*t2828;
t2867 = t15.*t2828;
t2892 = dq7.*t2890.*-2.0;
t2896 = dq7.*t2890.*2.0;
t2928 = -t2816.*(t88-t617);
t2947 = -t2941;
t2949 = t831.*t2832;
t2950 = -t2828.*(t88-t617);
t2953 = t2828.*(t88-t617);
t2973 = -t2967;
t3009 = t2890.*(-3.466000000000001e-2);
t3013 = t2890.*3.466000000000001e-2;
t3014 = dq7.*t2890.*(-4.648e-2);
t3016 = -t3011;
t3021 = dq7.*t2890.*4.648e-2;
t3024 = -t2828.*(t653-t838);
t3039 = t1473+t2875;
t3043 = t1590+t2873;
t3055 = -t3052;
t3057 = -t3054;
t3062 = -t3061;
t3065 = t2966.*2.37e-3;
t3066 = t2966.*2.75e-2;
t3068 = t2965.*5.000000000000001e-5;
t3070 = -t3067;
t3071 = t2000.*t2816;
t3072 = t2967.*4.9e-4;
t3073 = -t3069;
t3076 = t811+t978+t1874+t2615;
t3078 = t2970.*2.019e-2;
t3079 = -t3074;
t3080 = -t3077;
t3083 = t2000.*t2828;
t3086 = t806+t1015+t1915+t2613;
t3088 = t2035.*t2832;
t3090 = t2970.*1.9738e-1;
t3091 = t2983.*4.9e-4;
t3093 = -t3085;
t3101 = t2984.*2.019e-2;
t3102 = -t3095;
t3103 = -t3100;
t3105 = t803+t1035+t1873+t2664;
t3109 = t2163.*t2816;
t3110 = t821+t979+t1917+t2686;
t3115 = t2147.*t2832;
t3116 = t2984.*1.9738e-1;
t3117 = -t8.*(t755+t1012-t1873-t2664);
t3118 = -t15.*(t755+t1012-t1873-t2664);
t3121 = t759+t1014+t1955+t2695;
t3122 = t2163.*t2828;
t3123 = t694+t696+t1094+t1318+t2716;
t3124 = t758+t1033+t1901+t2704;
t3126 = t2816.*(t88-t617).*(-9.999999999999998e-6);
t3130 = t2816.*(t88-t617).*9.999999999999998e-6;
t3131 = t850+t937+t2223+t2501;
t3134 = t777+t1161+t1828+t2697;
t3145 = -t8.*(t696+t1094-t2697+t14.*(t637-t1126));
t3146 = -t15.*(t696+t1094-t2697+t14.*(t637-t1126));
t3147 = t2816.*(t88-t617).*(-1.0e-5);
t3154 = t8.*t3132;
t3155 = t15.*t3132;
t3156 = t2816.*(t88-t617).*(-2.769999999999999e-3);
t3157 = t928+t932+t942+t2215+t2287;
t3158 = t935+t950+t981+t2183+t2254;
t3161 = t853+t945+t983+t2258+t2264;
t3162 = t706+t1092+t1829+t2751;
t3163 = t700+t1064+t1861+t2747;
t3165 = t762+t813+t1088+t1216+t2742;
t3166 = t774+t776+t1093+t1224+t2752;
t3167 = t2828.*(t653-t838).*(-4.466636216449161e-20);
t3168 = t950+t981+t2183+t2513;
t3169 = t984+t992+t2187+t2497;
t3170 = t2960.*3.0e-5;
t3171 = t2961.*3.0e-5;
t3173 = -t8.*(-t928+t984+t992+t2187+t2240);
t3174 = -t15.*(-t928+t984+t992+t2187+t2240);
t3187 = -t3181;
t3190 = t2960.*5.0e-5;
t3191 = t2961.*5.0e-5;
t3195 = t2960.*5.000000000000004e-4;
t3196 = t2961.*5.000000000000004e-4;
t3197 = -t8.*(t776+t1093-t2737+t14.*(t708-t1079));
t3198 = -t15.*(t776+t1093-t2737+t14.*(t708-t1079));
t3201 = t887+t1017+t2225+t2570;
t3202 = t897+t986+t2268+t2571;
t3204 = t897+t986+t1018+t2268+t2301;
t3207 = t2828.*(t653-t838).*(-9.999999999999998e-6);
t3208 = t2828.*(t653-t838).*9.999999999999998e-6;
t3216 = -t3215;
t3220 = -t3217;
t3223 = -t3219;
t3224 = -t3221;
t3225 = t3029.*3.844e-2;
t3227 = t3029.*1.12e-3;
t3228 = t3029.*8.8e-4;
t3230 = -t3229;
t3231 = t2828.*(t653-t838).*(-1.2e-4);
t3233 = -t3232;
t3235 = t3085.*4.466636216449161e-20;
t3264 = t3085.*1.0e-5;
t3274 = -t3269;
t3277 = t3085.*2.840000000000012e-3;
t3288 = t3112.*1.089e-2;
t3289 = t3113.*1.089e-2;
t3290 = t3112.*2.9e-4;
t3291 = t3113.*2.9e-4;
t3293 = t3112.*2.2e-4;
t3294 = t3113.*2.2e-4;
t3300 = t3149.*(-3.0e-5);
t3305 = t3149.*(-5.0e-5);
t3306 = t3149.*5.0e-5;
t3307 = t3149.*(-5.000000000000004e-4);
t3319 = t951+t1617+t2180+t2860;
t3324 = t2816.*t2828;
t3332 = dq7.*t3329.*-2.0;
t3335 = t995+t1585+t2263+t2874;
t3336 = t953+t1589+t2267+t2890;
t3337 = dq7.*t3329.*2.0;
t3338 = -t2832.*(t639-t1128-t2181+dq5.*t13.*(t86-t652));
t3342 = t1207.*t3314;
t3346 = dq7.*t3329.*(-6.932000000000001e-2);
t3349 = t3329.*(-2.324e-2);
t3352 = dq7.*t3329.*6.932000000000001e-2;
t3354 = t3329.*2.324e-2;
t3361 = -t3357;
t3362 = -t3358;
t3368 = t2832.*(t639-t1128-t2181+dq5.*t13.*(t86-t652)).*(-4.466636216449161e-20);
t3371 = t2832.*(t639-t1128-t2181+dq5.*t13.*(t86-t652)).*(-9.999999999999998e-6);
t3373 = t3339.*4.000000000000028e-5;
t3374 = t3339.*3.0e-5;
t3376 = -t3313.*(t8.*(t92-t663)+t15.*(t621-t864));
t3379 = -t2074.*(t878-t1582+t2184+t7.*(t639-t1128-t2181+dq5.*t13.*(t86-t652)));
t3381 = t3339.*2.32e-3;
t3383 = t2832.*(t639-t1128-t2181+dq5.*t13.*(t86-t652)).*(-1.2e-4);
t3395 = t3357.*3.0e-5;
t3396 = t3358.*3.0e-5;
t3400 = t3357.*5.0e-5;
t3401 = t3358.*5.0e-5;
t3405 = t3357.*5.000000000000004e-4;
t3406 = t3358.*5.000000000000004e-4;
t3409 = t3365.*(-2.2e-4);
t3411 = t3365.*(-2.900000000000001e-4);
t3415 = t3365.*(-7.950000000000001e-3);
t3422 = t751+t904+t1103+t2277+t2282+t2965;
t3433 = t683+t997+t1238+t2160+t2250+t2987;
t3435 = t680+t1019+t1243+t2157+t2248+t2978;
t3447 = t753+t964+t1244+t2204+t2283+t2983;
t3453 = -t8.*(t684-t964+t1188+t2172-t2283-t2983);
t3454 = -t15.*(t684-t964+t1188+t2172-t2283-t2983);
t3456 = t988+t1886+t2482+t3189;
t3458 = t2074.*(t878-t1582+t2184+t7.*(t639-t1128-t2181+dq5.*t13.*(t86-t652))).*(-3.0e-5);
t3461 = t2074.*(t878-t1582+t2184+t7.*(t639-t1128-t2181+dq5.*t13.*(t86-t652))).*(-4.000000000000028e-5);
t3462 = t2074.*(t878-t1582+t2184+t7.*(t639-t1128-t2181+dq5.*t13.*(t86-t652))).*4.000000000000028e-5;
t3464 = t3313.*(t8.*(t92-t663)+t15.*(t621-t864)).*(-2.900000000000001e-4);
t3465 = t3313.*(t8.*(t92-t663)+t15.*(t621-t864)).*(-2.9e-4);
t3466 = t2074.*(t878-t1582+t2184+t7.*(t639-t1128-t2181+dq5.*t13.*(t86-t652))).*(-2.32e-3);
t3467 = t2074.*(t878-t1582+t2184+t7.*(t639-t1128-t2181+dq5.*t13.*(t86-t652))).*2.32e-3;
t3468 = t3313.*(t8.*(t92-t663)+t15.*(t621-t864)).*(-2.94e-3);
t3485 = t1091+t1826+t2729+t3135;
t3486 = t1063+t1824+t2728+t3148;
t3502 = -t2832.*(t878-t1582+t2184+t7.*(t639-t1128-t2181+dq5.*t13.*(t86-t652)));
t3503 = -t2832.*(t884+t1578-t2180+t14.*(t639-t1128-t2181+dq5.*t13.*(t86-t652)));
t3512 = t2832.*(t878-t1582+t2184+t7.*(t639-t1128-t2181+dq5.*t13.*(t86-t652)));
t3517 = t8.*(t684-t964+t1188+t2172-t2283-t2983).*(-3.466000000000001e-2);
t3519 = t15.*(t684-t964+t1188+t2172-t2283-t2983).*(-2.324e-2);
t3520 = t8.*(t684-t964+t1188+t2172-t2283-t2983).*3.466000000000001e-2;
t3524 = -t1207.*(t684-t964+t1188+t2172-t2283-t2983);
t3525 = t1207.*(t684-t964+t1188+t2172-t2283-t2983);
t3546 = t1140+t1629+t2414+t2431+t2528+t2562;
t3577 = t2832.*(t884+t1578-t2180+t14.*(t639-t1128-t2181+dq5.*t13.*(t86-t652))).*(-3.0e-5);
t3579 = t2832.*(t884+t1578-t2180+t14.*(t639-t1128-t2181+dq5.*t13.*(t86-t652))).*3.0e-5;
t3581 = t2832.*(t884+t1578-t2180+t14.*(t639-t1128-t2181+dq5.*t13.*(t86-t652))).*(-5.0e-5);
t3583 = t2832.*(t884+t1578-t2180+t14.*(t639-t1128-t2181+dq5.*t13.*(t86-t652))).*(-5.000000000000004e-4);
t3585 = t2832.*(t884+t1578-t2180+t14.*(t639-t1128-t2181+dq5.*t13.*(t86-t652))).*5.000000000000004e-4;
t3594 = t3522.*2.2e-4;
t3596 = t3522.*2.900000000000001e-4;
t3599 = t3522.*7.950000000000001e-3;
t3631 = t3622.*3.0e-5;
t3633 = t3622.*4.000000000000028e-5;
t3634 = t3622.*2.32e-3;
t3666 = t1288+t1289+t2201+t2529+t2557+t3027+t3029;
t3670 = t464+t467+t1141+t1144+t1183+t1612+t1671+t1706+t1815+t1882+t2013+t2014+t2094+t2531+t2580;
t3675 = t2104+t2360+t2788+t2807+t3044+t3058;
t3726 = (t8.*(t92-t663)+t15.*(t621-t864)).*(t977-t2307-t2975+t8.*(t684-t964+t1188+t2172-t2283-t2983)+t22.*t1601+dq7.*t15.*(t642+t896-t1137-t2220).*2.0);
t3765 = t2368+t2456+t2549+t2653+t2696+t2789+t2809+t2876+t2888;
t3767 = t2391+t2467+t2508+t2693+t2730+t2798+t2815+t2843+t2853;
t3768 = t2348+t2463+t2612+t2636+t2678+t2796+t2819+t2902+t2904;
t3786 = t557+t590+t591+t1164+t1165+t1197+t1198+t1199+t1208+t1664+t1673+t1727+t1935+t1967+t1992+t2086+t2133+t2492+t2540+t2545+t2547+t2573+t3081+t3089;
t1787 = -t1755;
t1797 = -t1771;
t2076 = -t2051;
t2115 = -t2090;
t2161 = -t2139;
t2338 = t1031+t1783;
t2355 = t1755.*3.466000000000001e-2;
t2358 = t1750.*3.466000000000001e-2;
t2366 = t1771.*2.324e-2;
t2367 = t1753.*2.324e-2;
t2395 = t1889.*(-3.466000000000001e-2);
t2485 = t2067.*3.466000000000001e-2;
t2487 = t2064.*2.324e-2;
t2500 = t2112.*3.466000000000001e-2;
t2504 = t2100.*3.466000000000001e-2;
t2505 = t2110.*2.324e-2;
t2510 = t2103.*2.324e-2;
t2517 = t2142.*3.466000000000001e-2;
t2524 = t2132.*2.324e-2;
t2604 = t2576.^2;
t2656 = t2627.^2;
t2660 = -t2640;
t2661 = -t2641;
t2837 = t8.*t2823;
t2838 = t15.*t2823;
t2845 = dq7.*t2824.*2.0;
t2846 = dq7.*t2826.*2.0;
t2871 = -t2865;
t2878 = dq7.*t2859.*2.0;
t2880 = dq7.*t2863.*2.0;
t2881 = dq6.*t2864.*2.0;
t2882 = dq6.*t2866.*2.0;
t2883 = t8.*t2857;
t2884 = t15.*t2857;
t2976 = t2826.*3.466000000000001e-2;
t2980 = dq7.*t2826.*4.648e-2;
t2981 = dq7.*t2824.*6.932000000000001e-2;
t2982 = t2824.*2.324e-2;
t2985 = t2864.*4.9e-4;
t2991 = dq6.*t2866.*9.8e-4;
t2993 = t2866.*2.019e-2;
t2996 = t2867.*3.466000000000001e-2;
t2997 = dq6.*t2864.*4.038e-2;
t2998 = t2825.*1.9738e-1;
t3001 = t2863.*3.466000000000001e-2;
t3003 = dq7.*t2863.*4.648e-2;
t3005 = dq7.*t2859.*6.932000000000001e-2;
t3007 = t2859.*2.324e-2;
t3008 = t2865.*2.324e-2;
t3020 = t2861.*1.9738e-1;
t3022 = t2866.*1.9738e-1;
t3030 = dq6.*t2864.*3.9476e-1;
t3035 = t1581+t2825;
t3038 = t1625+t2823;
t3042 = t1616+t2861;
t3045 = t1661+t2857;
t3075 = -t3072;
t3082 = -t3078;
t3096 = -t3091;
t3098 = t809+t1013+t1909+t2642;
t3104 = t758+t1033+t1871+t2682;
t3119 = -t3109;
t3128 = t8.*t3121;
t3129 = t15.*t3121;
t3133 = t704+t1159+t1825+t2715;
t3143 = t2949.*9.999999999999998e-6;
t3144 = t2953.*(-9.999999999999998e-6);
t3152 = t8.*t3131;
t3153 = t15.*t3131;
t3160 = t895+t931+t2218+t2515;
t3172 = t2953.*(-1.0e-5);
t3176 = t2949.*2.769999999999999e-3;
t3177 = t2953.*(-2.769999999999999e-3);
t3179 = t2949.*1.0e-5;
t3182 = -t3171;
t3183 = t2953.*1.0e-5;
t3184 = t779+t1158+t1827+t2749;
t3185 = t812+t1160+t1831+t2737;
t3193 = t8.*t3166;
t3194 = t15.*t3166;
t3237 = -t3235;
t3246 = t3122.*4.466636216449161e-20;
t3250 = t3071.*4.000000000000028e-5;
t3253 = t3071.*5.0e-5;
t3255 = t3083.*4.000000000000028e-5;
t3256 = t3071.*2.81e-3;
t3257 = t3083.*5.0e-5;
t3259 = t3088.*4.000000000000028e-5;
t3262 = t3088.*5.0e-5;
t3263 = t3083.*2.81e-3;
t3267 = t3088.*2.81e-3;
t3268 = t3109.*9.999999999999998e-6;
t3273 = t3115.*9.999999999999998e-6;
t3279 = t3109.*1.0e-5;
t3280 = t3109.*2.769999999999999e-3;
t3281 = -t3277;
t3284 = t3115.*2.769999999999999e-3;
t3296 = t3115.*1.0e-5;
t3301 = t3122.*1.0e-5;
t3311 = t3122.*2.840000000000012e-3;
t3312 = t894+t1471+t2214+t2866;
t3317 = t883+t1587+t2265+t2864;
t3325 = -t8.*(t1487+t2219-t2864+dq6.*t7.*(t88-t617));
t3326 = -t15.*(t1487+t2219-t2864+dq6.*t7.*(t88-t617));
t3327 = dq7.*t8.*(t1487+t2219-t2864+dq6.*t7.*(t88-t617)).*-2.0;
t3328 = dq7.*t15.*(t1487+t2219-t2864+dq6.*t7.*(t88-t617)).*-2.0;
t3330 = -t3324;
t3333 = t8.*(t1487+t2219-t2864+dq6.*t7.*(t88-t617));
t3345 = t15.*(t1487+t2219-t2864+dq6.*t7.*(t88-t617)).*(-2.324e-2);
t3350 = dq7.*t15.*(t1487+t2219-t2864+dq6.*t7.*(t88-t617)).*(-6.932000000000001e-2);
t3355 = dq7.*t15.*(t1487+t2219-t2864+dq6.*t7.*(t88-t617)).*6.932000000000001e-2;
t3356 = (t653-t838).*(t1487+t2219-t2864+dq6.*t7.*(t88-t617));
t3360 = t1207.*t3336;
t3363 = t3324.*4.466636216449161e-20;
t3369 = t3324.*9.999999999999998e-6;
t3375 = t3324.*1.2e-4;
t3377 = (t1386+t7.*(t88-t617)).*(t1487+t2219-t2864+dq6.*t7.*(t88-t617));
t3385 = -t3336.*(t8.*(t92-t663)+t15.*(t621-t864));
t3386 = t2138+t3323;
t3393 = t3342.*2.900000000000001e-4;
t3394 = t3342.*2.2e-4;
t3398 = -t3395;
t3399 = t3342.*7.950000000000001e-3;
t3403 = -t3400;
t3404 = -t3401;
t3407 = -t3405;
t3408 = -t3406;
t3420 = -t2601.*(t1487+t2219-t2864+dq6.*t7.*(t88-t617));
t3421 = t2601.*(t1487+t2219-t2864+dq6.*t7.*(t88-t617));
t3423 = t799+t872+t1104+t2230+t2294+t2966;
t3424 = -t2654.*(t878-t1582+t2184+t7.*(t639-t1128-t2181+dq5.*t13.*(t86-t652)));
t3425 = -t2654.*(t884+t1578-t2180+t14.*(t639-t1128-t2181+dq5.*t13.*(t86-t652)));
t3427 = t7.*t3422;
t3428 = t14.*t3422;
t3429 = t946+t982+t1803+t2259+t3155;
t3432 = t936+t938+t1833+t2302+t3154;
t3436 = t681+t923+t1246+t2170+t2295+t2984;
t3441 = t7.*t3433;
t3442 = t14.*t3433;
t3444 = t930+t933+t1888+t2208+t3173;
t3445 = t8.*t3435;
t3446 = t15.*t3435;
t3449 = t939+t980+t1853+t2255+t3174;
t3455 = t985+t1857+t2499+t3188;
t3459 = t1045+t1750+t2683+t3117;
t3471 = t1045+t1750+t2702+t3137;
t3473 = t3336.*(t8.*(t92-t663)+t15.*(t621-t864)).*(-2.9e-4);
t3474 = t3336.*(t8.*(t92-t663)+t15.*(t621-t864)).*(-2.900000000000001e-4);
t3475 = t2378+t2928+t2949;
t3477 = t3336.*(t8.*(t92-t663)+t15.*(t621-t864)).*(-2.94e-3);
t3484 = t831.*t3435;
t3488 = t1063+t1824+t2726+t3146;
t3490 = t1060+t1859+t2736+t3145;
t3497 = -t2816.*(t1487+t2219-t2864+dq6.*t7.*(t88-t617));
t3504 = t1062+t1854+t2738+t3198;
t3510 = -t3422.*(t653-t838);
t3514 = t1059+t1889+t2750+t3197;
t3521 = -t3433.*(t614+t13.*(t86-t652));
t3523 = -t3336.*(t631-t885+t1132-t2224);
t3538 = t2654.*(t878-t1582+t2184+t7.*(t639-t1128-t2181+dq5.*t13.*(t86-t652))).*(-1.089e-2);
t3539 = t2654.*(t884+t1578-t2180+t14.*(t639-t1128-t2181+dq5.*t13.*(t86-t652))).*(-1.089e-2);
t3540 = t2654.*(t878-t1582+t2184+t7.*(t639-t1128-t2181+dq5.*t13.*(t86-t652))).*(-2.9e-4);
t3541 = t2654.*(t884+t1578-t2180+t14.*(t639-t1128-t2181+dq5.*t13.*(t86-t652))).*(-2.9e-4);
t3542 = t2654.*(t878-t1582+t2184+t7.*(t639-t1128-t2181+dq5.*t13.*(t86-t652))).*(-2.2e-4);
t3543 = t2654.*(t884+t1578-t2180+t14.*(t639-t1128-t2181+dq5.*t13.*(t86-t652))).*(-2.2e-4);
t3547 = t2035.*t3435;
t3548 = t2446+t3024+t3036;
t3553 = t3422.*(t653-t838).*(-4.466636216449161e-20);
t3562 = t3433.*(t614+t13.*(t86-t652)).*(-4.466636216449161e-20);
t3570 = t2816.*(t1487+t2219-t2864+dq6.*t7.*(t88-t617)).*(-4.000000000000028e-5);
t3572 = t2816.*(t1487+t2219-t2864+dq6.*t7.*(t88-t617)).*4.000000000000028e-5;
t3573 = t2816.*(t1487+t2219-t2864+dq6.*t7.*(t88-t617)).*(-5.0e-5);
t3574 = t3422.*(t653-t838).*(-9.999999999999998e-6);
t3575 = t2816.*(t1487+t2219-t2864+dq6.*t7.*(t88-t617)).*(-2.81e-3);
t3576 = t3512.*(-4.000000000000028e-5);
t3578 = t2816.*(t1487+t2219-t2864+dq6.*t7.*(t88-t617)).*2.81e-3;
t3580 = t3512.*(-5.0e-5);
t3582 = t3512.*5.0e-5;
t3584 = t3512.*(-2.81e-3);
t3586 = t3433.*(t614+t13.*(t86-t652)).*(-9.999999999999998e-6);
t3587 = t3525.*(-4.000000000000028e-5);
t3588 = t3525.*(-3.0e-5);
t3589 = t3525.*4.000000000000028e-5;
t3590 = t3422.*(t653-t838).*(-1.2e-4);
t3591 = t3525.*3.0e-5;
t3592 = t3336.*(t631-t885+t1132-t2224).*(-1.089e-2);
t3593 = t3336.*(t631-t885+t1132-t2224).*(-2.9e-4);
t3595 = t3336.*(t631-t885+t1132-t2224).*(-2.2e-4);
t3597 = t3525.*(-2.32e-3);
t3598 = t3525.*2.32e-3;
t3600 = t3433.*(t614+t13.*(t86-t652)).*(-1.2e-4);
t3610 = t2668+t3071+t3088;
t3619 = t1618+t2112+t2863+t3320;
t3620 = t1662+t2110+t2859+t3329;
t3623 = -t3336.*(t958-t2263+dq7.*t1601+t15.*(t642+t896-t1137-t2220));
t3635 = t3336.*(t958-t2263+dq7.*t1601+t15.*(t642+t896-t1137-t2220)).*(-2.9e-4);
t3636 = t3336.*(t958-t2263+dq7.*t1601+t15.*(t642+t896-t1137-t2220)).*(-2.900000000000001e-4);
t3637 = t3336.*(t958-t2263+dq7.*t1601+t15.*(t642+t896-t1137-t2220)).*(-2.94e-3);
t3674 = t236+t237+t239+t463+t516+t518+t1263+t1264+t1328+t1674+t1693+t1699+t1878+t1891+t2093+t2114+t2126+t2575+t2579;
t3692 = t1010+t1609+t2307+t2893+t2975+t3453;
t3693 = t1000+t1611+t2308+t2896+t2988+t3454;
t3722 = -t1207.*(-t2308+t2892+t2979+t15.*(t684-t964+t1188+t2172-t2283-t2983)+t8.*t22.*(t92-t663)+t15.*t22.*(t621-t864));
t3723 = t1207.*(-t2308+t2892+t2979+t15.*(t684-t964+t1188+t2172-t2283-t2983)+t8.*t22.*(t92-t663)+t15.*t22.*(t621-t864));
C = ft_7({dq1,dq2,dq3,dq4,dq5,dq6,dq7,t10,t1001,t1003,t1004,t1007,t1008,t1012,t1014,t1015,t1016,t1017,t1018,t1020,t1021,t1022,t1023,t1024,t1025,t1026,t1034,t1036,t1038,t1039,t1040,t1041,t1044,t1046,t105,t1051,t1052,t1053,t1054,t1055,t1056,t1058,t1059,t1060,t1062,t1066,t1067,t1069,t107,t1070,t1072,t1075,t1077,t1079,t1081,t1088,t1090,t1093,t1094,t1096,t1097,t11,t1110,t1113,t1114,t1115,t1119,t112,t1123,t1125,t1126,t1128,t1130,t1132,t1136,t1137,t1138,t114,t1142,t1143,t1146,t1159,t1161,t1166,t1167,t1172,t1174,t1175,t1177,t1178,t1179,t1180,t1189,t119,t1190,t1194,t12,t1200,t1201,t1203,t1206,t1207,t1209,t1211,t1212,t1213,t1214,t1215,t1217,t1218,t1219,t122,t1220,t1226,t1231,t1232,t1256,t1267,t1268,t1269,t1273,t1274,t1275,t1286,t1295,t1296,t1299,t13,t130,t1304,t1312,t1313,t1315,t1329,t1330,t1339,t1341,t1342,t1346,t1347,t1350,t1351,t1352,t1360,t1368,t1369,t137,t1374,t1375,t1386,t1387,t1389,t139,t1391,t14,t1412,t1416,t1417,t1418,t1423,t1424,t1431,t1435,t144,t1441,t1449,t1455,t1456,t1462,t1467,t1472,t1487,t1488,t1489,t149,t1497,t1498,t15,t1506,t151,t1513,t1515,t1516,t152,t1526,t1528,t1529,t1543,t1546,t1553,t1554,t1557,t1564,t1565,t1569,t1574,t1577,t1578,t1579,t1581,t1582,t1583,t1584,t1591,t16,t160,t1601,t1603,t1604,t1605,t1606,t1608,t1613,t1616,t1619,t1622,t1625,t1626,t1627,t1633,t1634,t1635,t1636,t1638,t1642,t1643,t1644,t1645,t1647,t1648,t1649,t165,t1650,t1651,t1652,t1654,t1655,t1657,t1658,t1660,t1661,t1662,t1663,t1667,t1668,t1672,t1675,t1678,t1679,t1680,t1681,t1682,t1683,t1685,t1686,t1687,t1688,t1694,t1697,t17,t1700,t1701,t1702,t1704,t1705,t1707,t171,t1710,t1711,t1715,t1717,t1718,t1719,t1720,t1721,t1723,t1725,t1726,t1729,t1731,t1732,t1734,t1735,t1736,t1737,t1738,t1740,t1742,t1743,t1745,t1746,t1748,t1749,t175,t1750,t1751,t1752,t1753,t1755,t1759,t1760,t1762,t1765,t1766,t1769,t1770,t1771,t1772,t1773,t1774,t1775,t1776,t1778,t1779,t1780,t1782,t1786,t1787,t1790,t1791,t1792,t1795,t1797,t1798,t1799,t180,t1800,t1801,t1802,t1803,t1804,t1805,t1806,t1807,t1811,t1812,t1813,t1814,t1816,t1817,t1819,t182,t1822,t1823,t1830,t1834,t1835,t1836,t1837,t1839,t1840,t1841,t1842,t1843,t1846,t1849,t185,t1850,t1851,t1852,t1853,t1854,t1855,t1856,t1858,t1859,t186,t1860,t1861,t1863,t1864,t1865,t1866,t1867,t187,t1871,t1872,t1873,t1874,t1875,t1876,t1877,t1880,t1881,t1883,t1884,t1885,t1886,t1888,t1889,t189,t1890,t1892,t1893,t1896,t1897,t1898,t1899,t1900,t1901,t1902,t1903,t1905,t1907,t1908,t1909,t1911,t1912,t1913,t1914,t1917,t1918,t1919,t1924,t1927,t1928,t1931,t1932,t1934,t1936,t1938,t1939,t1940,t1941,t1942,t1944,t1945,t1946,t1949,t1950,t1951,t1952,t1953,t1954,t1955,t1957,t1959,t1960,t1962,t1963,t1969,t1970,t1971,t1974,t1975,t1976,t1977,t1978,t1980,t1982,t1984,t1985,t1986,t1988,t1993,t1997,t1998,t2,t2000,t2001,t2002,t2003,t2006,t2008,t2009,t2010,t2011,t2018,t2022,t2026,t2028,t2029,t2032,t2033,t2034,t2035,t2036,t2041,t2042,t2044,t2045,t2046,t2047,t2049,t2051,t2054,t2056,t2058,t2060,t2064,t2065,t2066,t2067,t2071,t2072,t2073,t2074,t2075,t2076,t2077,t2078,t208,t2080,t2081,t2085,t2088,t2089,t2090,t2095,t2096,t2098,t2100,t2103,t2105,t2108,t2109,t2111,t2115,t2119,t2125,t2130,t2132,t2139,t2140,t2141,t2142,t2147,t2148,t2149,t2151,t2152,t2161,t2163,t2164,t2165,t2171,t2173,t2177,t2179,t2180,t2181,t2182,t2183,t2184,t2187,t2193,t2195,t2196,t2197,t2198,t22,t2200,t2203,t2205,t2206,t2207,t2208,t221,t2212,t2215,t2217,t2219,t2220,t2224,t2227,t2228,t223,t2231,t2233,t2237,t2240,t2242,t2245,t2246,t2249,t2251,t2253,t2256,t2257,t2258,t2259,t2261,t2262,t2263,t2264,t2266,t2269,t2270,t2278,t2280,t2286,t2288,t2289,t2290,t2293,t2296,t2297,t23,t230,t2300,t2301,t2309,t231,t2310,t2311,t2312,t2313,t2315,t2316,t2319,t232,t2323,t2326,t2327,t2330,t2333,t2339,t234,t2341,t2343,t235,t2350,t2351,t2352,t2355,t2356,t2357,t2358,t2359,t236,t2360,t2363,t2365,t2366,t2367,t2369,t237,t2370,t2372,t2374,t2375,t2376,t2379,t238,t2380,t2382,t2383,t2384,t2385,t2387,t2388,t239,t2392,t2393,t2395,t2399,t24,t240,t2400,t2402,t2404,t2407,t2409,t241,t2411,t2418,t242,t2424,t2429,t243,t2435,t2439,t244,t2440,t2443,t2444,t2445,t2447,t2455,t2456,t2458,t2459,t2460,t2462,t2463,t2464,t2466,t2467,t2469,t2470,t2471,t2472,t2473,t2474,t2475,t2477,t2482,t2483,t2485,t2486,t2487,t2488,t2494,t2496,t25,t250,t2500,t2501,t2503,t2504,t2505,t2506,t2507,t2509,t251,t2510,t2513,t2514,t2516,t2517,t252,t2521,t2522,t2523,t2524,t2525,t253,t2533,t2534,t2536,t2537,t2538,t2539,t254,t2541,t2543,t2551,t2554,t2555,t2556,t2558,t2559,t2560,t2561,t2563,t2568,t2569,t2570,t2571,t2572,t2576,t2577,t2578,t258,t2581,t2584,t2585,t2586,t2587,t2589,t259,t2590,t2591,t2596,t2597,t2598,t2599,t26,t2601,t2602,t2603,t2604,t2606,t2609,t2610,t2611,t2612,t2613,t2614,t2615,t2617,t2618,t2620,t2621,t2622,t2623,t2624,t2627,t2628,t2629,t2630,t2631,t2633,t2634,t2635,t2637,t2638,t2640,t2641,t2642,t2643,t2644,t2646,t2647,t2648,t2651,t2652,t2653,t2654,t2655,t2656,t2657,t2659,t2660,t2661,t2662,t2663,t2664,t2665,t2666,t2667,t2669,t267,t2670,t2671,t2672,t2674,t2675,t2677,t2679,t268,t2680,t2681,t2684,t2685,t2687,t2689,t269,t2690,t2691,t2692,t2693,t2694,t2697,t2698,t2699,t27,t270,t2700,t2701,t2703,t2706,t2707,t2708,t271,t2710,t2711,t2714,t2717,t2718,t272,t2720,t2721,t2722,t2723,t2726,t2727,t2728,t2729,t273,t2732,t2734,t2735,t2737,t2738,t2739,t274,t2740,t2741,t2742,t2743,t2744,t2747,t2748,t275,t2751,t2753,t2754,t2756,t2757,t276,t2765,t2766,t2767,t277,t2771,t2774,t2775,t2776,t2777,t2780,t2781,t2783,t2788,t2789,t279,t2790,t2791,t2792,t2793,t2794,t2795,t2796,t2797,t2798,t2799,t28,t280,t2801,t2803,t2804,t2806,t2807,t2808,t281,t2810,t2811,t2812,t2813,t2814,t2816,t2817,t2818,t282,t2820,t2821,t2823,t2824,t2825,t2826,t2827,t2828,t2829,t283,t2832,t2833,t2837,t2838,t2839,t284,t2840,t2841,t2842,t2844,t2845,t2846,t2847,t2848,t285,t2852,t2854,t2855,t2857,t2858,t286,t2861,t2862,t2864,t2867,t2868,t2869,t287,t2871,t2878,t288,t2880,t2881,t2882,t2883,t2884,t2885,t2886,t2887,t289,t2891,t2895,t2897,t2898,t29,t290,t2900,t2901,t2903,t2905,t2907,t2908,t2909,t2911,t2912,t2914,t2915,t2917,t2919,t2920,t2921,t2922,t2923,t2924,t2925,t2926,t2929,t293,t2930,t2931,t2935,t2936,t2937,t2939,t2940,t2941,t2942,t2943,t2944,t2945,t2946,t2947,t2948,t2949,t295,t2950,t2952,t2953,t2954,t2955,t2956,t2957,t2959,t296,t2960,t2961,t2962,t2968,t2969,t297,t2970,t2972,t2973,t2974,t2976,t298,t2980,t2981,t2982,t2985,t2989,t2990,t2991,t2992,t2993,t2994,t2995,t2996,t2997,t2998,t2999,t3,t30,t3001,t3003,t3005,t3007,t3008,t3009,t301,t3011,t3013,t3016,t3018,t3020,t3021,t3022,t3023,t3025,t3026,t3030,t3031,t3032,t3035,t3037,t3038,t3039,t3042,t3045,t3049,t3051,t3052,t3055,t3056,t3057,t3059,t3060,t3062,t3064,t3065,t3066,t3067,t3068,t307,t3070,t3071,t3073,t3075,t3076,t3079,t308,t3080,t3082,t3083,t3084,t3085,t3086,t3088,t309,t3090,t3092,t3093,t3094,t3096,t3097,t3098,t31,t310,t3101,t3102,t3103,t3104,t3108,t311,t3112,t3113,t3114,t3115,t3116,t3118,t3119,t312,t3120,t3121,t3122,t3124,t3126,t3128,t3129,t313,t3130,t3131,t3132,t3133,t3138,t3139,t3140,t3141,t3142,t3143,t3147,t3148,t3149,t3152,t3153,t3154,t3155,t3156,t3159,t3161,t3162,t3163,t3165,t3166,t3167,t3168,t317,t3170,t3171,t3172,t3175,t3176,t3179,t318,t3181,t3182,t3186,t3187,t319,t3190,t3191,t3192,t3193,t3194,t3195,t3196,t32,t320,t3201,t3202,t3203,t3204,t3205,t3206,t3208,t3210,t3211,t3212,t3213,t3214,t3215,t3216,t3220,t3222,t3223,t3224,t3225,t3226,t3227,t3228,t3229,t3230,t3231,t3232,t3233,t3235,t3236,t3237,t3238,t3240,t3241,t3242,t3243,t3244,t3246,t3247,t3248,t3249,t3250,t3251,t3252,t3253,t3254,t3255,t3256,t3257,t3259,t3261,t3262,t3263,t3264,t3267,t3268,t3269,t327,t3272,t3273,t3274,t3275,t3276,t3277,t3279,t328,t3280,t3281,t3282,t3284,t3285,t3286,t3287,t3288,t3289,t329,t3290,t3291,t3292,t3293,t3294,t3295,t3296,t3297,t33,t330,t3300,t3301,t3302,t3304,t3306,t3307,t3309,t331,t3310,t3311,t3312,t3313,t3321,t3324,t3326,t3328,t3330,t3331,t3333,t3336,t3337,t3338,t3339,t3342,t3343,t3345,t3351,t3352,t3354,t3355,t3356,t3357,t3358,t3359,t3360,t3361,t3362,t3363,t3364,t3365,t3368,t3369,t3371,t3372,t3373,t3374,t3375,t3377,t3379,t338,t3381,t3383,t3385,t3386,t3393,t3394,t3395,t3396,t3398,t3399,t34,t3400,t3403,t3404,t3406,t3407,t3408,t3409,t3411,t3415,t342,t3421,t3422,t3423,t3424,t3425,t3427,t3428,t3429,t3433,t3436,t3440,t3441,t3442,t3443,t3444,t3445,t3446,t3458,t346,t3462,t3464,t3465,t3467,t3468,t347,t3473,t3474,t3476,t3477,t348,t3484,t3486,t3488,t349,t3490,t3497,t35,t3502,t3503,t3504,t3510,t3512,t3514,t3519,t3520,t3521,t3522,t3523,t3525,t3538,t3539,t3540,t3541,t3542,t3543,t3546,t3547,t3553,t3562,t3572,t3573,t3574,t3576,t3578,t3579,t358,t3581,t3582,t3584,t3585,t3586,t3589,t3590,t3591,t3592,t3593,t3594,t3595,t3596,t3598,t3599,t36,t3600,t3610,t3619,t3620,t3622,t3623,t3628,t3631,t3633,t3634,t3635,t3636,t3637,t3640,t3641,t3666,t3667,t3668,t3669,t3670,t3671,t3672,t3673,t3674,t3679,t37,t3723,t3726,t3779,t3780,t3781,t3786,t3811,t3812,t3816,t39,t4,t40,t427,t428,t429,t43,t431,t432,t433,t434,t435,t436,t438,t439,t441,t442,t443,t444,t446,t448,t45,t450,t451,t452,t453,t455,t456,t457,t458,t459,t46,t460,t461,t463,t464,t465,t466,t467,t468,t469,t483,t484,t49,t494,t495,t496,t5,t50,t51,t510,t511,t512,t515,t516,t517,t518,t522,t523,t524,t525,t526,t527,t528,t529,t530,t531,t533,t534,t535,t536,t537,t538,t542,t543,t545,t546,t547,t548,t549,t55,t550,t551,t552,t553,t554,t556,t557,t558,t561,t562,t563,t564,t565,t566,t567,t568,t569,t57,t570,t571,t572,t573,t574,t575,t576,t577,t578,t579,t58,t580,t581,t582,t583,t584,t585,t586,t587,t588,t589,t590,t591,t592,t593,t594,t595,t596,t597,t598,t599,t6,t600,t601,t602,t603,t604,t605,t606,t607,t608,t609,t61,t612,t613,t614,t615,t616,t617,t618,t619,t620,t621,t622,t624,t626,t629,t63,t631,t632,t633,t634,t635,t637,t639,t64,t640,t642,t643,t644,t646,t647,t648,t649,t650,t651,t652,t653,t654,t656,t657,t658,t660,t661,t662,t663,t664,t665,t667,t67,t673,t676,t677,t678,t685,t686,t687,t688,t689,t69,t691,t692,t693,t694,t696,t697,t698,t7,t70,t701,t702,t703,t704,t705,t707,t708,t71,t72,t721,t722,t723,t724,t725,t726,t728,t729,t73,t730,t731,t735,t74,t740,t743,t75,t754,t755,t756,t757,t759,t76,t760,t762,t769,t77,t770,t773,t774,t776,t777,t778,t78,t782,t785,t786,t787,t788,t79,t791,t792,t795,t796,t797,t8,t80,t800,t805,t806,t81,t813,t814,t815,t816,t817,t818,t819,t82,t827,t83,t831,t834,t835,t836,t837,t838,t839,t84,t840,t841,t842,t843,t845,t846,t847,t85,t853,t854,t855,t856,t857,t859,t86,t860,t863,t864,t866,t867,t87,t870,t871,t873,t876,t877,t878,t88,t880,t881,t882,t884,t885,t888,t889,t89,t890,t891,t896,t898,t899,t9,t90,t900,t902,t905,t907,t908,t91,t911,t92,t921,t922,t926,t927,t928,t930,t932,t933,t935,t939,t94,t940,t942,t946,t948,t949,t952,t958,t959,t961,t963,t966,t969,t97,t972,t973,t974,t975,t982,t983,t984,t987,t988,t992,t994,t999});
end
function C = ft_7(ct)
dq1 = ct{1};
dq2 = ct{2};
dq3 = ct{3};
dq4 = ct{4};
dq5 = ct{5};
dq6 = ct{6};
dq7 = ct{7};
t10 = ct{8};
t1001 = ct{9};
t1003 = ct{10};
t1004 = ct{11};
t1007 = ct{12};
t1008 = ct{13};
t1012 = ct{14};
t1014 = ct{15};
t1015 = ct{16};
t1016 = ct{17};
t1017 = ct{18};
t1018 = ct{19};
t1020 = ct{20};
t1021 = ct{21};
t1022 = ct{22};
t1023 = ct{23};
t1024 = ct{24};
t1025 = ct{25};
t1026 = ct{26};
t1034 = ct{27};
t1036 = ct{28};
t1038 = ct{29};
t1039 = ct{30};
t1040 = ct{31};
t1041 = ct{32};
t1044 = ct{33};
t1046 = ct{34};
t105 = ct{35};
t1051 = ct{36};
t1052 = ct{37};
t1053 = ct{38};
t1054 = ct{39};
t1055 = ct{40};
t1056 = ct{41};
t1058 = ct{42};
t1059 = ct{43};
t1060 = ct{44};
t1062 = ct{45};
t1066 = ct{46};
t1067 = ct{47};
t1069 = ct{48};
t107 = ct{49};
t1070 = ct{50};
t1072 = ct{51};
t1075 = ct{52};
t1077 = ct{53};
t1079 = ct{54};
t1081 = ct{55};
t1088 = ct{56};
t1090 = ct{57};
t1093 = ct{58};
t1094 = ct{59};
t1096 = ct{60};
t1097 = ct{61};
t11 = ct{62};
t1110 = ct{63};
t1113 = ct{64};
t1114 = ct{65};
t1115 = ct{66};
t1119 = ct{67};
t112 = ct{68};
t1123 = ct{69};
t1125 = ct{70};
t1126 = ct{71};
t1128 = ct{72};
t1130 = ct{73};
t1132 = ct{74};
t1136 = ct{75};
t1137 = ct{76};
t1138 = ct{77};
t114 = ct{78};
t1142 = ct{79};
t1143 = ct{80};
t1146 = ct{81};
t1159 = ct{82};
t1161 = ct{83};
t1166 = ct{84};
t1167 = ct{85};
t1172 = ct{86};
t1174 = ct{87};
t1175 = ct{88};
t1177 = ct{89};
t1178 = ct{90};
t1179 = ct{91};
t1180 = ct{92};
t1189 = ct{93};
t119 = ct{94};
t1190 = ct{95};
t1194 = ct{96};
t12 = ct{97};
t1200 = ct{98};
t1201 = ct{99};
t1203 = ct{100};
t1206 = ct{101};
t1207 = ct{102};
t1209 = ct{103};
t1211 = ct{104};
t1212 = ct{105};
t1213 = ct{106};
t1214 = ct{107};
t1215 = ct{108};
t1217 = ct{109};
t1218 = ct{110};
t1219 = ct{111};
t122 = ct{112};
t1220 = ct{113};
t1226 = ct{114};
t1231 = ct{115};
t1232 = ct{116};
t1256 = ct{117};
t1267 = ct{118};
t1268 = ct{119};
t1269 = ct{120};
t1273 = ct{121};
t1274 = ct{122};
t1275 = ct{123};
t1286 = ct{124};
t1295 = ct{125};
t1296 = ct{126};
t1299 = ct{127};
t13 = ct{128};
t130 = ct{129};
t1304 = ct{130};
t1312 = ct{131};
t1313 = ct{132};
t1315 = ct{133};
t1329 = ct{134};
t1330 = ct{135};
t1339 = ct{136};
t1341 = ct{137};
t1342 = ct{138};
t1346 = ct{139};
t1347 = ct{140};
t1350 = ct{141};
t1351 = ct{142};
t1352 = ct{143};
t1360 = ct{144};
t1368 = ct{145};
t1369 = ct{146};
t137 = ct{147};
t1374 = ct{148};
t1375 = ct{149};
t1386 = ct{150};
t1387 = ct{151};
t1389 = ct{152};
t139 = ct{153};
t1391 = ct{154};
t14 = ct{155};
t1412 = ct{156};
t1416 = ct{157};
t1417 = ct{158};
t1418 = ct{159};
t1423 = ct{160};
t1424 = ct{161};
t1431 = ct{162};
t1435 = ct{163};
t144 = ct{164};
t1441 = ct{165};
t1449 = ct{166};
t1455 = ct{167};
t1456 = ct{168};
t1462 = ct{169};
t1467 = ct{170};
t1472 = ct{171};
t1487 = ct{172};
t1488 = ct{173};
t1489 = ct{174};
t149 = ct{175};
t1497 = ct{176};
t1498 = ct{177};
t15 = ct{178};
t1506 = ct{179};
t151 = ct{180};
t1513 = ct{181};
t1515 = ct{182};
t1516 = ct{183};
t152 = ct{184};
t1526 = ct{185};
t1528 = ct{186};
t1529 = ct{187};
t1543 = ct{188};
t1546 = ct{189};
t1553 = ct{190};
t1554 = ct{191};
t1557 = ct{192};
t1564 = ct{193};
t1565 = ct{194};
t1569 = ct{195};
t1574 = ct{196};
t1577 = ct{197};
t1578 = ct{198};
t1579 = ct{199};
t1581 = ct{200};
t1582 = ct{201};
t1583 = ct{202};
t1584 = ct{203};
t1591 = ct{204};
t16 = ct{205};
t160 = ct{206};
t1601 = ct{207};
t1603 = ct{208};
t1604 = ct{209};
t1605 = ct{210};
t1606 = ct{211};
t1608 = ct{212};
t1613 = ct{213};
t1616 = ct{214};
t1619 = ct{215};
t1622 = ct{216};
t1625 = ct{217};
t1626 = ct{218};
t1627 = ct{219};
t1633 = ct{220};
t1634 = ct{221};
t1635 = ct{222};
t1636 = ct{223};
t1638 = ct{224};
t1642 = ct{225};
t1643 = ct{226};
t1644 = ct{227};
t1645 = ct{228};
t1647 = ct{229};
t1648 = ct{230};
t1649 = ct{231};
t165 = ct{232};
t1650 = ct{233};
t1651 = ct{234};
t1652 = ct{235};
t1654 = ct{236};
t1655 = ct{237};
t1657 = ct{238};
t1658 = ct{239};
t1660 = ct{240};
t1661 = ct{241};
t1662 = ct{242};
t1663 = ct{243};
t1667 = ct{244};
t1668 = ct{245};
t1672 = ct{246};
t1675 = ct{247};
t1678 = ct{248};
t1679 = ct{249};
t1680 = ct{250};
t1681 = ct{251};
t1682 = ct{252};
t1683 = ct{253};
t1685 = ct{254};
t1686 = ct{255};
t1687 = ct{256};
t1688 = ct{257};
t1694 = ct{258};
t1697 = ct{259};
t17 = ct{260};
t1700 = ct{261};
t1701 = ct{262};
t1702 = ct{263};
t1704 = ct{264};
t1705 = ct{265};
t1707 = ct{266};
t171 = ct{267};
t1710 = ct{268};
t1711 = ct{269};
t1715 = ct{270};
t1717 = ct{271};
t1718 = ct{272};
t1719 = ct{273};
t1720 = ct{274};
t1721 = ct{275};
t1723 = ct{276};
t1725 = ct{277};
t1726 = ct{278};
t1729 = ct{279};
t1731 = ct{280};
t1732 = ct{281};
t1734 = ct{282};
t1735 = ct{283};
t1736 = ct{284};
t1737 = ct{285};
t1738 = ct{286};
t1740 = ct{287};
t1742 = ct{288};
t1743 = ct{289};
t1745 = ct{290};
t1746 = ct{291};
t1748 = ct{292};
t1749 = ct{293};
t175 = ct{294};
t1750 = ct{295};
t1751 = ct{296};
t1752 = ct{297};
t1753 = ct{298};
t1755 = ct{299};
t1759 = ct{300};
t1760 = ct{301};
t1762 = ct{302};
t1765 = ct{303};
t1766 = ct{304};
t1769 = ct{305};
t1770 = ct{306};
t1771 = ct{307};
t1772 = ct{308};
t1773 = ct{309};
t1774 = ct{310};
t1775 = ct{311};
t1776 = ct{312};
t1778 = ct{313};
t1779 = ct{314};
t1780 = ct{315};
t1782 = ct{316};
t1786 = ct{317};
t1787 = ct{318};
t1790 = ct{319};
t1791 = ct{320};
t1792 = ct{321};
t1795 = ct{322};
t1797 = ct{323};
t1798 = ct{324};
t1799 = ct{325};
t180 = ct{326};
t1800 = ct{327};
t1801 = ct{328};
t1802 = ct{329};
t1803 = ct{330};
t1804 = ct{331};
t1805 = ct{332};
t1806 = ct{333};
t1807 = ct{334};
t1811 = ct{335};
t1812 = ct{336};
t1813 = ct{337};
t1814 = ct{338};
t1816 = ct{339};
t1817 = ct{340};
t1819 = ct{341};
t182 = ct{342};
t1822 = ct{343};
t1823 = ct{344};
t1830 = ct{345};
t1834 = ct{346};
t1835 = ct{347};
t1836 = ct{348};
t1837 = ct{349};
t1839 = ct{350};
t1840 = ct{351};
t1841 = ct{352};
t1842 = ct{353};
t1843 = ct{354};
t1846 = ct{355};
t1849 = ct{356};
t185 = ct{357};
t1850 = ct{358};
t1851 = ct{359};
t1852 = ct{360};
t1853 = ct{361};
t1854 = ct{362};
t1855 = ct{363};
t1856 = ct{364};
t1858 = ct{365};
t1859 = ct{366};
t186 = ct{367};
t1860 = ct{368};
t1861 = ct{369};
t1863 = ct{370};
t1864 = ct{371};
t1865 = ct{372};
t1866 = ct{373};
t1867 = ct{374};
t187 = ct{375};
t1871 = ct{376};
t1872 = ct{377};
t1873 = ct{378};
t1874 = ct{379};
t1875 = ct{380};
t1876 = ct{381};
t1877 = ct{382};
t1880 = ct{383};
t1881 = ct{384};
t1883 = ct{385};
t1884 = ct{386};
t1885 = ct{387};
t1886 = ct{388};
t1888 = ct{389};
t1889 = ct{390};
t189 = ct{391};
t1890 = ct{392};
t1892 = ct{393};
t1893 = ct{394};
t1896 = ct{395};
t1897 = ct{396};
t1898 = ct{397};
t1899 = ct{398};
t1900 = ct{399};
t1901 = ct{400};
t1902 = ct{401};
t1903 = ct{402};
t1905 = ct{403};
t1907 = ct{404};
t1908 = ct{405};
t1909 = ct{406};
t1911 = ct{407};
t1912 = ct{408};
t1913 = ct{409};
t1914 = ct{410};
t1917 = ct{411};
t1918 = ct{412};
t1919 = ct{413};
t1924 = ct{414};
t1927 = ct{415};
t1928 = ct{416};
t1931 = ct{417};
t1932 = ct{418};
t1934 = ct{419};
t1936 = ct{420};
t1938 = ct{421};
t1939 = ct{422};
t1940 = ct{423};
t1941 = ct{424};
t1942 = ct{425};
t1944 = ct{426};
t1945 = ct{427};
t1946 = ct{428};
t1949 = ct{429};
t1950 = ct{430};
t1951 = ct{431};
t1952 = ct{432};
t1953 = ct{433};
t1954 = ct{434};
t1955 = ct{435};
t1957 = ct{436};
t1959 = ct{437};
t1960 = ct{438};
t1962 = ct{439};
t1963 = ct{440};
t1969 = ct{441};
t1970 = ct{442};
t1971 = ct{443};
t1974 = ct{444};
t1975 = ct{445};
t1976 = ct{446};
t1977 = ct{447};
t1978 = ct{448};
t1980 = ct{449};
t1982 = ct{450};
t1984 = ct{451};
t1985 = ct{452};
t1986 = ct{453};
t1988 = ct{454};
t1993 = ct{455};
t1997 = ct{456};
t1998 = ct{457};
t2 = ct{458};
t2000 = ct{459};
t2001 = ct{460};
t2002 = ct{461};
t2003 = ct{462};
t2006 = ct{463};
t2008 = ct{464};
t2009 = ct{465};
t2010 = ct{466};
t2011 = ct{467};
t2018 = ct{468};
t2022 = ct{469};
t2026 = ct{470};
t2028 = ct{471};
t2029 = ct{472};
t2032 = ct{473};
t2033 = ct{474};
t2034 = ct{475};
t2035 = ct{476};
t2036 = ct{477};
t2041 = ct{478};
t2042 = ct{479};
t2044 = ct{480};
t2045 = ct{481};
t2046 = ct{482};
t2047 = ct{483};
t2049 = ct{484};
t2051 = ct{485};
t2054 = ct{486};
t2056 = ct{487};
t2058 = ct{488};
t2060 = ct{489};
t2064 = ct{490};
t2065 = ct{491};
t2066 = ct{492};
t2067 = ct{493};
t2071 = ct{494};
t2072 = ct{495};
t2073 = ct{496};
t2074 = ct{497};
t2075 = ct{498};
t2076 = ct{499};
t2077 = ct{500};
t2078 = ct{501};
t208 = ct{502};
t2080 = ct{503};
t2081 = ct{504};
t2085 = ct{505};
t2088 = ct{506};
t2089 = ct{507};
t2090 = ct{508};
t2095 = ct{509};
t2096 = ct{510};
t2098 = ct{511};
t2100 = ct{512};
t2103 = ct{513};
t2105 = ct{514};
t2108 = ct{515};
t2109 = ct{516};
t2111 = ct{517};
t2115 = ct{518};
t2119 = ct{519};
t2125 = ct{520};
t2130 = ct{521};
t2132 = ct{522};
t2139 = ct{523};
t2140 = ct{524};
t2141 = ct{525};
t2142 = ct{526};
t2147 = ct{527};
t2148 = ct{528};
t2149 = ct{529};
t2151 = ct{530};
t2152 = ct{531};
t2161 = ct{532};
t2163 = ct{533};
t2164 = ct{534};
t2165 = ct{535};
t2171 = ct{536};
t2173 = ct{537};
t2177 = ct{538};
t2179 = ct{539};
t2180 = ct{540};
t2181 = ct{541};
t2182 = ct{542};
t2183 = ct{543};
t2184 = ct{544};
t2187 = ct{545};
t2193 = ct{546};
t2195 = ct{547};
t2196 = ct{548};
t2197 = ct{549};
t2198 = ct{550};
t22 = ct{551};
t2200 = ct{552};
t2203 = ct{553};
t2205 = ct{554};
t2206 = ct{555};
t2207 = ct{556};
t2208 = ct{557};
t221 = ct{558};
t2212 = ct{559};
t2215 = ct{560};
t2217 = ct{561};
t2219 = ct{562};
t2220 = ct{563};
t2224 = ct{564};
t2227 = ct{565};
t2228 = ct{566};
t223 = ct{567};
t2231 = ct{568};
t2233 = ct{569};
t2237 = ct{570};
t2240 = ct{571};
t2242 = ct{572};
t2245 = ct{573};
t2246 = ct{574};
t2249 = ct{575};
t2251 = ct{576};
t2253 = ct{577};
t2256 = ct{578};
t2257 = ct{579};
t2258 = ct{580};
t2259 = ct{581};
t2261 = ct{582};
t2262 = ct{583};
t2263 = ct{584};
t2264 = ct{585};
t2266 = ct{586};
t2269 = ct{587};
t2270 = ct{588};
t2278 = ct{589};
t2280 = ct{590};
t2286 = ct{591};
t2288 = ct{592};
t2289 = ct{593};
t2290 = ct{594};
t2293 = ct{595};
t2296 = ct{596};
t2297 = ct{597};
t23 = ct{598};
t230 = ct{599};
t2300 = ct{600};
t2301 = ct{601};
t2309 = ct{602};
t231 = ct{603};
t2310 = ct{604};
t2311 = ct{605};
t2312 = ct{606};
t2313 = ct{607};
t2315 = ct{608};
t2316 = ct{609};
t2319 = ct{610};
t232 = ct{611};
t2323 = ct{612};
t2326 = ct{613};
t2327 = ct{614};
t2330 = ct{615};
t2333 = ct{616};
t2339 = ct{617};
t234 = ct{618};
t2341 = ct{619};
t2343 = ct{620};
t235 = ct{621};
t2350 = ct{622};
t2351 = ct{623};
t2352 = ct{624};
t2355 = ct{625};
t2356 = ct{626};
t2357 = ct{627};
t2358 = ct{628};
t2359 = ct{629};
t236 = ct{630};
t2360 = ct{631};
t2363 = ct{632};
t2365 = ct{633};
t2366 = ct{634};
t2367 = ct{635};
t2369 = ct{636};
t237 = ct{637};
t2370 = ct{638};
t2372 = ct{639};
t2374 = ct{640};
t2375 = ct{641};
t2376 = ct{642};
t2379 = ct{643};
t238 = ct{644};
t2380 = ct{645};
t2382 = ct{646};
t2383 = ct{647};
t2384 = ct{648};
t2385 = ct{649};
t2387 = ct{650};
t2388 = ct{651};
t239 = ct{652};
t2392 = ct{653};
t2393 = ct{654};
t2395 = ct{655};
t2399 = ct{656};
t24 = ct{657};
t240 = ct{658};
t2400 = ct{659};
t2402 = ct{660};
t2404 = ct{661};
t2407 = ct{662};
t2409 = ct{663};
t241 = ct{664};
t2411 = ct{665};
t2418 = ct{666};
t242 = ct{667};
t2424 = ct{668};
t2429 = ct{669};
t243 = ct{670};
t2435 = ct{671};
t2439 = ct{672};
t244 = ct{673};
t2440 = ct{674};
t2443 = ct{675};
t2444 = ct{676};
t2445 = ct{677};
t2447 = ct{678};
t2455 = ct{679};
t2456 = ct{680};
t2458 = ct{681};
t2459 = ct{682};
t2460 = ct{683};
t2462 = ct{684};
t2463 = ct{685};
t2464 = ct{686};
t2466 = ct{687};
t2467 = ct{688};
t2469 = ct{689};
t2470 = ct{690};
t2471 = ct{691};
t2472 = ct{692};
t2473 = ct{693};
t2474 = ct{694};
t2475 = ct{695};
t2477 = ct{696};
t2482 = ct{697};
t2483 = ct{698};
t2485 = ct{699};
t2486 = ct{700};
t2487 = ct{701};
t2488 = ct{702};
t2494 = ct{703};
t2496 = ct{704};
t25 = ct{705};
t250 = ct{706};
t2500 = ct{707};
t2501 = ct{708};
t2503 = ct{709};
t2504 = ct{710};
t2505 = ct{711};
t2506 = ct{712};
t2507 = ct{713};
t2509 = ct{714};
t251 = ct{715};
t2510 = ct{716};
t2513 = ct{717};
t2514 = ct{718};
t2516 = ct{719};
t2517 = ct{720};
t252 = ct{721};
t2521 = ct{722};
t2522 = ct{723};
t2523 = ct{724};
t2524 = ct{725};
t2525 = ct{726};
t253 = ct{727};
t2533 = ct{728};
t2534 = ct{729};
t2536 = ct{730};
t2537 = ct{731};
t2538 = ct{732};
t2539 = ct{733};
t254 = ct{734};
t2541 = ct{735};
t2543 = ct{736};
t2551 = ct{737};
t2554 = ct{738};
t2555 = ct{739};
t2556 = ct{740};
t2558 = ct{741};
t2559 = ct{742};
t2560 = ct{743};
t2561 = ct{744};
t2563 = ct{745};
t2568 = ct{746};
t2569 = ct{747};
t2570 = ct{748};
t2571 = ct{749};
t2572 = ct{750};
t2576 = ct{751};
t2577 = ct{752};
t2578 = ct{753};
t258 = ct{754};
t2581 = ct{755};
t2584 = ct{756};
t2585 = ct{757};
t2586 = ct{758};
t2587 = ct{759};
t2589 = ct{760};
t259 = ct{761};
t2590 = ct{762};
t2591 = ct{763};
t2596 = ct{764};
t2597 = ct{765};
t2598 = ct{766};
t2599 = ct{767};
t26 = ct{768};
t2601 = ct{769};
t2602 = ct{770};
t2603 = ct{771};
t2604 = ct{772};
t2606 = ct{773};
t2609 = ct{774};
t2610 = ct{775};
t2611 = ct{776};
t2612 = ct{777};
t2613 = ct{778};
t2614 = ct{779};
t2615 = ct{780};
t2617 = ct{781};
t2618 = ct{782};
t2620 = ct{783};
t2621 = ct{784};
t2622 = ct{785};
t2623 = ct{786};
t2624 = ct{787};
t2627 = ct{788};
t2628 = ct{789};
t2629 = ct{790};
t2630 = ct{791};
t2631 = ct{792};
t2633 = ct{793};
t2634 = ct{794};
t2635 = ct{795};
t2637 = ct{796};
t2638 = ct{797};
t2640 = ct{798};
t2641 = ct{799};
t2642 = ct{800};
t2643 = ct{801};
t2644 = ct{802};
t2646 = ct{803};
t2647 = ct{804};
t2648 = ct{805};
t2651 = ct{806};
t2652 = ct{807};
t2653 = ct{808};
t2654 = ct{809};
t2655 = ct{810};
t2656 = ct{811};
t2657 = ct{812};
t2659 = ct{813};
t2660 = ct{814};
t2661 = ct{815};
t2662 = ct{816};
t2663 = ct{817};
t2664 = ct{818};
t2665 = ct{819};
t2666 = ct{820};
t2667 = ct{821};
t2669 = ct{822};
t267 = ct{823};
t2670 = ct{824};
t2671 = ct{825};
t2672 = ct{826};
t2674 = ct{827};
t2675 = ct{828};
t2677 = ct{829};
t2679 = ct{830};
t268 = ct{831};
t2680 = ct{832};
t2681 = ct{833};
t2684 = ct{834};
t2685 = ct{835};
t2687 = ct{836};
t2689 = ct{837};
t269 = ct{838};
t2690 = ct{839};
t2691 = ct{840};
t2692 = ct{841};
t2693 = ct{842};
t2694 = ct{843};
t2697 = ct{844};
t2698 = ct{845};
t2699 = ct{846};
t27 = ct{847};
t270 = ct{848};
t2700 = ct{849};
t2701 = ct{850};
t2703 = ct{851};
t2706 = ct{852};
t2707 = ct{853};
t2708 = ct{854};
t271 = ct{855};
t2710 = ct{856};
t2711 = ct{857};
t2714 = ct{858};
t2717 = ct{859};
t2718 = ct{860};
t272 = ct{861};
t2720 = ct{862};
t2721 = ct{863};
t2722 = ct{864};
t2723 = ct{865};
t2726 = ct{866};
t2727 = ct{867};
t2728 = ct{868};
t2729 = ct{869};
t273 = ct{870};
t2732 = ct{871};
t2734 = ct{872};
t2735 = ct{873};
t2737 = ct{874};
t2738 = ct{875};
t2739 = ct{876};
t274 = ct{877};
t2740 = ct{878};
t2741 = ct{879};
t2742 = ct{880};
t2743 = ct{881};
t2744 = ct{882};
t2747 = ct{883};
t2748 = ct{884};
t275 = ct{885};
t2751 = ct{886};
t2753 = ct{887};
t2754 = ct{888};
t2756 = ct{889};
t2757 = ct{890};
t276 = ct{891};
t2765 = ct{892};
t2766 = ct{893};
t2767 = ct{894};
t277 = ct{895};
t2771 = ct{896};
t2774 = ct{897};
t2775 = ct{898};
t2776 = ct{899};
t2777 = ct{900};
t2780 = ct{901};
t2781 = ct{902};
t2783 = ct{903};
t2788 = ct{904};
t2789 = ct{905};
t279 = ct{906};
t2790 = ct{907};
t2791 = ct{908};
t2792 = ct{909};
t2793 = ct{910};
t2794 = ct{911};
t2795 = ct{912};
t2796 = ct{913};
t2797 = ct{914};
t2798 = ct{915};
t2799 = ct{916};
t28 = ct{917};
t280 = ct{918};
t2801 = ct{919};
t2803 = ct{920};
t2804 = ct{921};
t2806 = ct{922};
t2807 = ct{923};
t2808 = ct{924};
t281 = ct{925};
t2810 = ct{926};
t2811 = ct{927};
t2812 = ct{928};
t2813 = ct{929};
t2814 = ct{930};
t2816 = ct{931};
t2817 = ct{932};
t2818 = ct{933};
t282 = ct{934};
t2820 = ct{935};
t2821 = ct{936};
t2823 = ct{937};
